simulink model "PMSMDriveThermal"  (R2025b)
(part 21 of 24)

  Battery (Table-Based)25 : batteryecm_lib/Battery (Table-Based)  SOC_vec=[0.1, 0.188889, 0.277778, 0.366667, 0.455556, 0.544444, 0.633333, 0.722222, 0.811111, 0.9]  T_dependence=simscape.enum.tablebattery.temperature_dependence.yes  prm_dir=simscape.enum.tablebattery.prm_dir.noCurrentDirectionality  T_vec=[30, 32.5, 35, 38] degC  V0_mat=|  V0_vec=[3.5057, 3.566, 3.6337, 3.7127, 3.9259, 4.0777, 4.1928] V  V_range=[0, inf] V  R0_mat=|  R0_vec=[.0085, .0085, .0087, .0082, .0083, .0085, .0085] Ohm  R0_dis_mat=[.0117, .0085, .009; .011, .0085, .009; .0114, .0087, .0092; .0107, .0082, .0088; .0107, .0083, .0091; .0113, .0085, .0089; .0116, .0085, .0089] Ohm  R0_dis_vec=[.0085, .0085, .0087, .0082, .0083, .0085, .0085] Ohm  R0_ch_mat=[.0117, .0085, .009; .011, .0085, .009; .0114, .0087, .0092; .0107, .0082, .0088; .0107, .0083, .0091; .0113, .0085, .0089; .0116, .0085, .0089] Ohm  R0_ch_vec=[.0085, .0085, .0087, .0082, .0083, .0085, .0085] Ohm  AH=5 A*hr  prm_leak=simscape.enum.tablebattery.prm_leak.disabled  Rleak_vec=[8000, 7000, 6000] Ohm  Rleak=7e3 Ohm  extrapolation_option=simscape.enum.extrapolation.nearest  SOC_port=simscape.enum.tablebattery.enable.no  prm_dyn=simscape.enum.tablebattery.prm_dyn.rc2  R1_mat=|  R1_vec=[.0029, .0024, .0026, .0016, .0023, .0018, .0017] Ohm  tau1_mat=|  tau1_vec=[36, 45, 105, 29, 77, 33, 39] s  R2_mat=|  R2_vec=[.0029, .0024, .0026, .0016, .0023, .0018, .0017] Ohm  tau2_mat=|  tau2_vec=[36, 45, 105, 29, 77, 33, 39] s  R3_mat=[.0109, .0029, .0013; .0069, .0024, .0012; .0047, .0026, .0013; .0034, .0016, .001; .0033, .0023, .0014; .0033, .0018, .0011; .0028, .0017, .0011] Ohm  R3_vec=[.0029, .0024, .0026, .0016, .0023, .0018, .0017] Ohm  tau3_mat=[20, 36, 39; 31, 45, 39; 109, 105, 61; 36, 29, 26; 59, 77, 67; 40, 33, 29; 25, 39, 33] s  tau3_vec=[36, 45, 105, 29, 77, 33, 39] s  R4_mat=[.0109, .0029, .0013; .0069, .0024, .0012; .0047, .0026, .0013; .0034, .0016, .001; .0033, .0023, .0014; .0033, .0018, .0011; .0028, .0017, .0011] Ohm  R4_vec=[.0029, .0024, .0026, .0016, .0023, .0018, .0017] Ohm  tau4_mat=[20, 36, 39; 31, 45, 39; 109, 105, 61; 36, 29, 26; 59, 77, 67; 40, 33, 29; 25, 39, 33] s  tau4_vec=[36, 45, 105, 29, 77, 33, 39] s  R5_mat=[.0109, .0029, .0013; .0069, .0024, .0012; .0047, .0026, .0013; .0034, .0016, .001; .0033, .0023, .0014; .0033, .0018, .0011; .0028, .0017, .0011] Ohm  R5_vec=[.0029, .0024, .0026, .0016, .0023, .0018, .0017] Ohm  tau5_mat=[20, 36, 39; 31, 45, 39; 109, 105, 61; 36, 29, 26; 59, 77, 67; 40, 33, 29; 25, 39, 33] s  tau5_vec=[36, 45, 105, 29, 77, 33, 39] s  prm_fade=simscape.enum.tablebattery.prm_fade.disabled  N0=100  dV0=0  dR0=0  dAH=0  dRleak=0  dR1=0  dR2=0  dR3=0  dR4=0  dR5=0  N0vec=[0, 100, 200, 300]  Tfadevec=[298.15, 323.15] K  dV0vec=[0, 0, 0, 0]  dR0vec=[0, 0, 0, 0]  dAHvec=[0, 0, 0, 0]  dRleakvec=[0, 0, 0, 0]  dR1vec=[0, 0, 0, 0]  dR2vec=[0, 0, 0, 0]  dR3vec=[0, 0, 0, 0]  dR4vec=[0, 0, 0, 0]  dR5vec=[0, 0, 0, 0]  dV0mat=[0, 0; 0, 0; 0, 0; 0, 0]  dR0mat=[0, 0; 0, 0; 0, 0; 0, 0]  dAHmat=[0, 0; 0, 0; 0, 0; 0, 0]  dRleakmat=[0, 0; 0, 0; 0, 0; 0, 0]  dR1mat=[0, 0; 0, 0; 0, 0; 0, 0]  dR2mat=[0, 0; 0, 0; 0, 0; 0, 0]  dR3mat=[0, 0; 0, 0; 0, 0; 0, 0]  dR4mat=[0, 0; 0, 0; 0, 0; 0, 0]  dR5mat=[0, 0; 0, 0; 0, 0; 0, 0]  prm_age_modeling=simscape.enum.tablebattery.prm_age_modeling.equation  storage_dt_age_vec=[0] d  storage_T_age_vec=[273] K  prm_age_OCV=simscape.enum.tablebattery.prm_age_OCV.OCV  OCV_age=0.9  SOC_age=0.6  prm_age_resistance=simscape.enum.tablebattery.prm_age.disabled  OCV_scaling_age_resistance=2.2134e6  OCV_offset_age_resistance=1.632e6  temp_exp_age_resistance=0.515833569 V  t_exp_age_resistance=0.75  T_age_vec_resistance=[273.15, 298.15, 323.15] K  dt_age_vec_resistance=[0, 90, 180, 270] d  dR0_age_vec=[0, 0, 0]  t_meas_dR0_age=100 d  dR0_age_mat=[0, 0, 0; 0, 0, 0; 0, 0, 0; 0, 0, 0]  prm_age_capacity=simscape.enum.tablebattery.prm_age.disabled  OCV_scaling_age_capacity=1.5097e07  OCV_offset_age_capacity=8.3625e06  temp_exp_age_capacity=0.6011 V  t_exp_age_capacity=0.75  T_age_vec_capacity=[273.15, 298.15, 323.15] K  dt_age_vec_capacity=[0, 90, 180, 270] d  dAH_age_vec=[0, 0, 0]  t_meas_dAH_age=100 d  dAH_age_mat=[0, 0, 0; 0, 0, 0; 0, 0, 0; 0, 0, 0]  thermal_port=simscape.enum.thermaleffects.omit  temperature=298.15 K  thermal_mass=100 J/K  i_specify=off  i_priority=None  i=0 A  i_nominal_specify=off  i_nominal_value=1  i_nominal_unit=A  v_specify=off  v_priority=None  v=0 V  v_nominal_specify=off  v_nominal_value=1  v_nominal_unit=V  stateOfCharge_specify=on  stateOfCharge_priority=High  stateOfCharge=1  stateOfCharge_nominal_specify=off  stateOfCharge_nominal_value=1  stateOfCharge_nominal_unit=1  num_cycles_specify=off  num_cycles_priority=High  num_cycles=0  num_cycles_nominal_specify=off  num_cycles_nominal_value=1  num_cycles_nominal_unit=1  cell_temperature_specify=off  cell_temperature_priority=High  cell_temperature=298.15 K  cell_temperature_nominal_specify=off  cell_temperature_nominal_value=1  cell_temperature_nominal_unit=K
      V0_mat=|
      | [3.0263, 3.218033, 3.364889, 3.493933, 3.610678, 3.733744, 3.85405, 3.950717, 4.040478, 4.0819;
      |  3.0376, 3.2248, 3.370311, 3.498533, 3.615311, 3.736956, 3.845633, 3.929256, 4.040056, 4.0821;
      |  3.0439, 3.227633, 3.3731, 3.5007, 3.616611, 3.737589, 3.8457, 3.9287, 4.039133, 4.0826;
      |  3.0283, 3.217989, 3.364589, 3.493767, 3.609467, 3.731156, 3.8417, 3.925833, 4.036322, 4.0821]' V
      R0_mat=|
      | [0.011867, 0.008993, 0.007674, 0.006911, 0.006648, 0.006648, 0.006528, 0.006157, 0.005996, 0.0073;
      |  0.0109, 0.006456, 0.005381, 0.005078, 0.005, 0.005044, 0.005511, 0.006407, 0.006522, 0.005367;
      |  0.0102, 0.007978, 0.006793, 0.0062, 0.006033, 0.005441, 0.0051, 0.005707, 0.005037, 0.005067;
      |  0.0101, 0.007759, 0.006637, 0.006022, 0.005741, 0.005667, 0.005311, 0.004911, 0.005859, 0.004733]' Ohm
      R1_mat=|
      | [0.007451, 0.008294, 0.007745, 0.007391;
      |  0.003783, 0.00363, 0.004415, 0.004051;
      |  0.002841, 0.00298, 0.003698, 0.003391;
      |  0.003185, 0.002661, 0.003493, 0.00379;
      |  0.00379, 0.003147, 0.004204, 0.004229;
      |  0.004015, 0.003677, 0.004233, 0.004481;
      |  0.003791, 0.004051, 0.003886, 0.004189;
      |  0.003416, 0.004883, 0.004387, 0.003743;
      |  0.00328, 0.005238, 0.003472, 0.004883;
      |  0.004816, 0.004218, 0.003847, 0.003891] Ohm
      tau1_mat=|
      | [8.156247, 6.866126, 6.747335, 6.573366;
      |  6.436096, 6.88158, 6.206576, 5.30011;
      |  7.074429, 7.267109, 6.564215, 5.759928;
      |  8.61232, 7.062398, 6.553799, 7.485573;
      |  10.88135, 8.569373, 8.681328, 8.99043;
      |  11.88702, 10.35435, 10.74073, 9.985533;
      |  11.15433, 10.61987, 10.52072, 10.95124;
      |  10.33388, 9.573709, 9.987626, 10.94588;
      |  9.883806, 9.219359, 8.513241, 9.109378;
      |  11.2706, 10.03414, 9.643065, 10.06297] s
      R2_mat=|
      | [0.040653, 0.04799, 0.046915, 0.044404;
      |  0.026828, 0.033189, 0.032279, 0.030363;
      |  0.019744, 0.025225, 0.021211, 0.019613;
      |  0.012414, 0.014827, 0.017004, 0.016763;
      |  0.007363, 0.008356, 0.01135, 0.010173;
      |  0.005882, 0.007703, 0.006532, 0.005526;
      |  0.006739, 0.007058, 0.006772, 0.005603;
      |  0.008222, 0.004287, 0.009601, 0.005034;
      |  0.008985, 0.007821, 0.008932, 0.006662;
      |  0.004704, 0.003171, 0.002422, 0.004036] Ohm
      tau2_mat=|
      | [131.6948, 137.0217, 141.2851, 129.3807;
      |  146.2759, 158.6208, 157.255, 143.944;
      |  158.5443, 177.3225, 156.7434, 144.0735;
      |  144.8009, 123.279, 145.0945, 176.1753;
      |  158.7596, 137.3241, 203.2495, 189.2199;
      |  149.8847, 154.5014, 161.1061, 146.3519;
      |  135.3572, 173.7062, 166.0613, 159.34;
      |  123.823, 144.5727, 209.652, 117.4544;
      |  111.7616, 98.04929, 114.3433, 98.05822;
      |  125.3862, 75.97092, 110.7081, 120.3015] s
      settings: InternalSimscapePortConfiguration="{\"Bottom\":[],\"Left\":[{\"id\":\"p\",\"label\":\"+\",\"type\":\"foundation.electrical.electrical\"}],\"Right\":[{\"id\":\"n\",\"label\":\"-\",\"type\":\"foundation.electrical.electrical\"}],\"Top\":[]}"
      settings: LibrarySourceBlock=|
      | batt_lib/Cells/Battery
      | (Table-Based)
  Battery (Table-Based)26 : batteryecm_lib/Battery (Table-Based)  SOC_vec=[0.1, 0.188889, 0.277778, 0.366667, 0.455556, 0.544444, 0.633333, 0.722222, 0.811111, 0.9]  T_dependence=simscape.enum.tablebattery.temperature_dependence.yes  prm_dir=simscape.enum.tablebattery.prm_dir.noCurrentDirectionality  T_vec=[30, 32.5, 35, 38] degC  V0_mat=|  V0_vec=[3.5057, 3.566, 3.6337, 3.7127, 3.9259, 4.0777, 4.1928] V  V_range=[0, inf] V  R0_mat=|  R0_vec=[.0085, .0085, .0087, .0082, .0083, .0085, .0085] Ohm  R0_dis_mat=[.0117, .0085, .009; .011, .0085, .009; .0114, .0087, .0092; .0107, .0082, .0088; .0107, .0083, .0091; .0113, .0085, .0089; .0116, .0085, .0089] Ohm  R0_dis_vec=[.0085, .0085, .0087, .0082, .0083, .0085, .0085] Ohm  R0_ch_mat=[.0117, .0085, .009; .011, .0085, .009; .0114, .0087, .0092; .0107, .0082, .0088; .0107, .0083, .0091; .0113, .0085, .0089; .0116, .0085, .0089] Ohm  R0_ch_vec=[.0085, .0085, .0087, .0082, .0083, .0085, .0085] Ohm  AH=5 A*hr  prm_leak=simscape.enum.tablebattery.prm_leak.disabled  Rleak_vec=[8000, 7000, 6000] Ohm  Rleak=7e3 Ohm  extrapolation_option=simscape.enum.extrapolation.nearest  SOC_port=simscape.enum.tablebattery.enable.no  prm_dyn=simscape.enum.tablebattery.prm_dyn.rc2  R1_mat=|  R1_vec=[.0029, .0024, .0026, .0016, .0023, .0018, .0017] Ohm  tau1_mat=|  tau1_vec=[36, 45, 105, 29, 77, 33, 39] s  R2_mat=|  R2_vec=[.0029, .0024, .0026, .0016, .0023, .0018, .0017] Ohm  tau2_mat=|  tau2_vec=[36, 45, 105, 29, 77, 33, 39] s  R3_mat=[.0109, .0029, .0013; .0069, .0024, .0012; .0047, .0026, .0013; .0034, .0016, .001; .0033, .0023, .0014; .0033, .0018, .0011; .0028, .0017, .0011] Ohm  R3_vec=[.0029, .0024, .0026, .0016, .0023, .0018, .0017] Ohm  tau3_mat=[20, 36, 39; 31, 45, 39; 109, 105, 61; 36, 29, 26; 59, 77, 67; 40, 33, 29; 25, 39, 33] s  tau3_vec=[36, 45, 105, 29, 77, 33, 39] s  R4_mat=[.0109, .0029, .0013; .0069, .0024, .0012; .0047, .0026, .0013; .0034, .0016, .001; .0033, .0023, .0014; .0033, .0018, .0011; .0028, .0017, .0011] Ohm  R4_vec=[.0029, .0024, .0026, .0016, .0023, .0018, .0017] Ohm  tau4_mat=[20, 36, 39; 31, 45, 39; 109, 105, 61; 36, 29, 26; 59, 77, 67; 40, 33, 29; 25, 39, 33] s  tau4_vec=[36, 45, 105, 29, 77, 33, 39] s  R5_mat=[.0109, .0029, .0013; .0069, .0024, .0012; .0047, .0026, .0013; .0034, .0016, .001; .0033, .0023, .0014; .0033, .0018, .0011; .0028, .0017, .0011] Ohm  R5_vec=[.0029, .0024, .0026, .0016, .0023, .0018, .0017] Ohm  tau5_mat=[20, 36, 39; 31, 45, 39; 109, 105, 61; 36, 29, 26; 59, 77, 67; 40, 33, 29; 25, 39, 33] s  tau5_vec=[36, 45, 105, 29, 77, 33, 39] s  prm_fade=simscape.enum.tablebattery.prm_fade.disabled  N0=100  dV0=0  dR0=0  dAH=0  dRleak=0  dR1=0  dR2=0  dR3=0  dR4=0  dR5=0  N0vec=[0, 100, 200, 300]  Tfadevec=[298.15, 323.15] K  dV0vec=[0, 0, 0, 0]  dR0vec=[0, 0, 0, 0]  dAHvec=[0, 0, 0, 0]  dRleakvec=[0, 0, 0, 0]  dR1vec=[0, 0, 0, 0]  dR2vec=[0, 0, 0, 0]  dR3vec=[0, 0, 0, 0]  dR4vec=[0, 0, 0, 0]  dR5vec=[0, 0, 0, 0]  dV0mat=[0, 0; 0, 0; 0, 0; 0, 0]  dR0mat=[0, 0; 0, 0; 0, 0; 0, 0]  dAHmat=[0, 0; 0, 0; 0, 0; 0, 0]  dRleakmat=[0, 0; 0, 0; 0, 0; 0, 0]  dR1mat=[0, 0; 0, 0; 0, 0; 0, 0]  dR2mat=[0, 0; 0, 0; 0, 0; 0, 0]  dR3mat=[0, 0; 0, 0; 0, 0; 0, 0]  dR4mat=[0, 0; 0, 0; 0, 0; 0, 0]  dR5mat=[0, 0; 0, 0; 0, 0; 0, 0]  prm_age_modeling=simscape.enum.tablebattery.prm_age_modeling.equation  storage_dt_age_vec=[0] d  storage_T_age_vec=[273] K  prm_age_OCV=simscape.enum.tablebattery.prm_age_OCV.OCV  OCV_age=0.9  SOC_age=0.6  prm_age_resistance=simscape.enum.tablebattery.prm_age.disabled  OCV_scaling_age_resistance=2.2134e6  OCV_offset_age_resistance=1.632e6  temp_exp_age_resistance=0.515833569 V  t_exp_age_resistance=0.75  T_age_vec_resistance=[273.15, 298.15, 323.15] K  dt_age_vec_resistance=[0, 90, 180, 270] d  dR0_age_vec=[0, 0, 0]  t_meas_dR0_age=100 d  dR0_age_mat=[0, 0, 0; 0, 0, 0; 0, 0, 0; 0, 0, 0]  prm_age_capacity=simscape.enum.tablebattery.prm_age.disabled  OCV_scaling_age_capacity=1.5097e07  OCV_offset_age_capacity=8.3625e06  temp_exp_age_capacity=0.6011 V  t_exp_age_capacity=0.75  T_age_vec_capacity=[273.15, 298.15, 323.15] K  dt_age_vec_capacity=[0, 90, 180, 270] d  dAH_age_vec=[0, 0, 0]  t_meas_dAH_age=100 d  dAH_age_mat=[0, 0, 0; 0, 0, 0; 0, 0, 0; 0, 0, 0]  thermal_port=simscape.enum.thermaleffects.omit  temperature=298.15 K  thermal_mass=100 J/K  i_specify=off  i_priority=None  i=0 A  i_nominal_specify=off  i_nominal_value=1  i_nominal_unit=A  v_specify=off  v_priority=None  v=0 V  v_nominal_specify=off  v_nominal_value=1  v_nominal_unit=V  stateOfCharge_specify=on  stateOfCharge_priority=High  stateOfCharge=1  stateOfCharge_nominal_specify=off  stateOfCharge_nominal_value=1  stateOfCharge_nominal_unit=1  num_cycles_specify=off  num_cycles_priority=High  num_cycles=0  num_cycles_nominal_specify=off  num_cycles_nominal_value=1  num_cycles_nominal_unit=1  cell_temperature_specify=off  cell_temperature_priority=High  cell_temperature=298.15 K  cell_temperature_nominal_specify=off  cell_temperature_nominal_value=1  cell_temperature_nominal_unit=K
      V0_mat=|
      | [3.0263, 3.218033, 3.364889, 3.493933, 3.610678, 3.733744, 3.85405, 3.950717, 4.040478, 4.0819;
      |  3.0376, 3.2248, 3.370311, 3.498533, 3.615311, 3.736956, 3.845633, 3.929256, 4.040056, 4.0821;
      |  3.0439, 3.227633, 3.3731, 3.5007, 3.616611, 3.737589, 3.8457, 3.9287, 4.039133, 4.0826;
      |  3.0283, 3.217989, 3.364589, 3.493767, 3.609467, 3.731156, 3.8417, 3.925833, 4.036322, 4.0821]' V
      R0_mat=|
      | [0.011867, 0.008993, 0.007674, 0.006911, 0.006648, 0.006648, 0.006528, 0.006157, 0.005996, 0.0073;
      |  0.0109, 0.006456, 0.005381, 0.005078, 0.005, 0.005044, 0.005511, 0.006407, 0.006522, 0.005367;
      |  0.0102, 0.007978, 0.006793, 0.0062, 0.006033, 0.005441, 0.0051, 0.005707, 0.005037, 0.005067;
      |  0.0101, 0.007759, 0.006637, 0.006022, 0.005741, 0.005667, 0.005311, 0.004911, 0.005859, 0.004733]' Ohm
      R1_mat=|
      | [0.007451, 0.008294, 0.007745, 0.007391;
      |  0.003783, 0.00363, 0.004415, 0.004051;
      |  0.002841, 0.00298, 0.003698, 0.003391;
      |  0.003185, 0.002661, 0.003493, 0.00379;
      |  0.00379, 0.003147, 0.004204, 0.004229;
      |  0.004015, 0.003677, 0.004233, 0.004481;
      |  0.003791, 0.004051, 0.003886, 0.004189;
      |  0.003416, 0.004883, 0.004387, 0.003743;
      |  0.00328, 0.005238, 0.003472, 0.004883;
      |  0.004816, 0.004218, 0.003847, 0.003891] Ohm
      tau1_mat=|
      | [8.156247, 6.866126, 6.747335, 6.573366;
      |  6.436096, 6.88158, 6.206576, 5.30011;
      |  7.074429, 7.267109, 6.564215, 5.759928;
      |  8.61232, 7.062398, 6.553799, 7.485573;
      |  10.88135, 8.569373, 8.681328, 8.99043;
      |  11.88702, 10.35435, 10.74073, 9.985533;
      |  11.15433, 10.61987, 10.52072, 10.95124;
      |  10.33388, 9.573709, 9.987626, 10.94588;
      |  9.883806, 9.219359, 8.513241, 9.109378;
      |  11.2706, 10.03414, 9.643065, 10.06297] s
      R2_mat=|
      | [0.040653, 0.04799, 0.046915, 0.044404;
      |  0.026828, 0.033189, 0.032279, 0.030363;
      |  0.019744, 0.025225, 0.021211, 0.019613;
      |  0.012414, 0.014827, 0.017004, 0.016763;
      |  0.007363, 0.008356, 0.01135, 0.010173;
      |  0.005882, 0.007703, 0.006532, 0.005526;
      |  0.006739, 0.007058, 0.006772, 0.005603;
      |  0.008222, 0.004287, 0.009601, 0.005034;
      |  0.008985, 0.007821, 0.008932, 0.006662;
      |  0.004704, 0.003171, 0.002422, 0.004036] Ohm
      tau2_mat=|
      | [131.6948, 137.0217, 141.2851, 129.3807;
      |  146.2759, 158.6208, 157.255, 143.944;
      |  158.5443, 177.3225, 156.7434, 144.0735;
      |  144.8009, 123.279, 145.0945, 176.1753;
      |  158.7596, 137.3241, 203.2495, 189.2199;
      |  149.8847, 154.5014, 161.1061, 146.3519;
      |  135.3572, 173.7062, 166.0613, 159.34;
      |  123.823, 144.5727, 209.652, 117.4544;
      |  111.7616, 98.04929, 114.3433, 98.05822;
      |  125.3862, 75.97092, 110.7081, 120.3015] s
      settings: InternalSimscapePortConfiguration="{\"Bottom\":[],\"Left\":[{\"id\":\"p\",\"label\":\"+\",\"type\":\"foundation.electrical.electrical\"}],\"Right\":[{\"id\":\"n\",\"label\":\"-\",\"type\":\"foundation.electrical.electrical\"}],\"Top\":[]}"
      settings: LibrarySourceBlock=|
      | batt_lib/Cells/Battery
      | (Table-Based)
  Battery (Table-Based)27 : batteryecm_lib/Battery (Table-Based)  SOC_vec=[0.1, 0.188889, 0.277778, 0.366667, 0.455556, 0.544444, 0.633333, 0.722222, 0.811111, 0.9]  T_dependence=simscape.enum.tablebattery.temperature_dependence.yes  prm_dir=simscape.enum.tablebattery.prm_dir.noCurrentDirectionality  T_vec=[30, 32.5, 35, 38] degC  V0_mat=|  V0_vec=[3.5057, 3.566, 3.6337, 3.7127, 3.9259, 4.0777, 4.1928] V  V_range=[0, inf] V  R0_mat=|  R0_vec=[.0085, .0085, .0087, .0082, .0083, .0085, .0085] Ohm  R0_dis_mat=[.0117, .0085, .009; .011, .0085, .009; .0114, .0087, .0092; .0107, .0082, .0088; .0107, .0083, .0091; .0113, .0085, .0089; .0116, .0085, .0089] Ohm  R0_dis_vec=[.0085, .0085, .0087, .0082, .0083, .0085, .0085] Ohm  R0_ch_mat=[.0117, .0085, .009; .011, .0085, .009; .0114, .0087, .0092; .0107, .0082, .0088; .0107, .0083, .0091; .0113, .0085, .0089; .0116, .0085, .0089] Ohm  R0_ch_vec=[.0085, .0085, .0087, .0082, .0083, .0085, .0085] Ohm  AH=5 A*hr  prm_leak=simscape.enum.tablebattery.prm_leak.disabled  Rleak_vec=[8000, 7000, 6000] Ohm  Rleak=7e3 Ohm  extrapolation_option=simscape.enum.extrapolation.nearest  SOC_port=simscape.enum.tablebattery.enable.no  prm_dyn=simscape.enum.tablebattery.prm_dyn.rc2  R1_mat=|  R1_vec=[.0029, .0024, .0026, .0016, .0023, .0018, .0017] Ohm  tau1_mat=|  tau1_vec=[36, 45, 105, 29, 77, 33, 39] s  R2_mat=|  R2_vec=[.0029, .0024, .0026, .0016, .0023, .0018, .0017] Ohm  tau2_mat=|  tau2_vec=[36, 45, 105, 29, 77, 33, 39] s  R3_mat=[.0109, .0029, .0013; .0069, .0024, .0012; .0047, .0026, .0013; .0034, .0016, .001; .0033, .0023, .0014; .0033, .0018, .0011; .0028, .0017, .0011] Ohm  R3_vec=[.0029, .0024, .0026, .0016, .0023, .0018, .0017] Ohm  tau3_mat=[20, 36, 39; 31, 45, 39; 109, 105, 61; 36, 29, 26; 59, 77, 67; 40, 33, 29; 25, 39, 33] s  tau3_vec=[36, 45, 105, 29, 77, 33, 39] s  R4_mat=[.0109, .0029, .0013; .0069, .0024, .0012; .0047, .0026, .0013; .0034, .0016, .001; .0033, .0023, .0014; .0033, .0018, .0011; .0028, .0017, .0011] Ohm  R4_vec=[.0029, .0024, .0026, .0016, .0023, .0018, .0017] Ohm  tau4_mat=[20, 36, 39; 31, 45, 39; 109, 105, 61; 36, 29, 26; 59, 77, 67; 40, 33, 29; 25, 39, 33] s  tau4_vec=[36, 45, 105, 29, 77, 33, 39] s  R5_mat=[.0109, .0029, .0013; .0069, .0024, .0012; .0047, .0026, .0013; .0034, .0016, .001; .0033, .0023, .0014; .0033, .0018, .0011; .0028, .0017, .0011] Ohm  R5_vec=[.0029, .0024, .0026, .0016, .0023, .0018, .0017] Ohm  tau5_mat=[20, 36, 39; 31, 45, 39; 109, 105, 61; 36, 29, 26; 59, 77, 67; 40, 33, 29; 25, 39, 33] s  tau5_vec=[36, 45, 105, 29, 77, 33, 39] s  prm_fade=simscape.enum.tablebattery.prm_fade.disabled  N0=100  dV0=0  dR0=0  dAH=0  dRleak=0  dR1=0  dR2=0  dR3=0  dR4=0  dR5=0  N0vec=[0, 100, 200, 300]  Tfadevec=[298.15, 323.15] K  dV0vec=[0, 0, 0, 0]  dR0vec=[0, 0, 0, 0]  dAHvec=[0, 0, 0, 0]  dRleakvec=[0, 0, 0, 0]  dR1vec=[0, 0, 0, 0]  dR2vec=[0, 0, 0, 0]  dR3vec=[0, 0, 0, 0]  dR4vec=[0, 0, 0, 0]  dR5vec=[0, 0, 0, 0]  dV0mat=[0, 0; 0, 0; 0, 0; 0, 0]  dR0mat=[0, 0; 0, 0; 0, 0; 0, 0]  dAHmat=[0, 0; 0, 0; 0, 0; 0, 0]  dRleakmat=[0, 0; 0, 0; 0, 0; 0, 0]  dR1mat=[0, 0; 0, 0; 0, 0; 0, 0]  dR2mat=[0, 0; 0, 0; 0, 0; 0, 0]  dR3mat=[0, 0; 0, 0; 0, 0; 0, 0]  dR4mat=[0, 0; 0, 0; 0, 0; 0, 0]  dR5mat=[0, 0; 0, 0; 0, 0; 0, 0]  prm_age_modeling=simscape.enum.tablebattery.prm_age_modeling.equation  storage_dt_age_vec=[0] d  storage_T_age_vec=[273] K  prm_age_OCV=simscape.enum.tablebattery.prm_age_OCV.OCV  OCV_age=0.9  SOC_age=0.6  prm_age_resistance=simscape.enum.tablebattery.prm_age.disabled  OCV_scaling_age_resistance=2.2134e6  OCV_offset_age_resistance=1.632e6  temp_exp_age_resistance=0.515833569 V  t_exp_age_resistance=0.75  T_age_vec_resistance=[273.15, 298.15, 323.15] K  dt_age_vec_resistance=[0, 90, 180, 270] d  dR0_age_vec=[0, 0, 0]  t_meas_dR0_age=100 d  dR0_age_mat=[0, 0, 0; 0, 0, 0; 0, 0, 0; 0, 0, 0]  prm_age_capacity=simscape.enum.tablebattery.prm_age.disabled  OCV_scaling_age_capacity=1.5097e07  OCV_offset_age_capacity=8.3625e06  temp_exp_age_capacity=0.6011 V  t_exp_age_capacity=0.75  T_age_vec_capacity=[273.15, 298.15, 323.15] K  dt_age_vec_capacity=[0, 90, 180, 270] d  dAH_age_vec=[0, 0, 0]  t_meas_dAH_age=100 d  dAH_age_mat=[0, 0, 0; 0, 0, 0; 0, 0, 0; 0, 0, 0]  thermal_port=simscape.enum.thermaleffects.omit  temperature=298.15 K  thermal_mass=100 J/K  i_specify=off  i_priority=None  i=0 A  i_nominal_specify=off  i_nominal_value=1  i_nominal_unit=A  v_specify=off  v_priority=None  v=0 V  v_nominal_specify=off  v_nominal_value=1  v_nominal_unit=V  stateOfCharge_specify=on  stateOfCharge_priority=High  stateOfCharge=1  stateOfCharge_nominal_specify=off  stateOfCharge_nominal_value=1  stateOfCharge_nominal_unit=1  num_cycles_specify=off  num_cycles_priority=High  num_cycles=0  num_cycles_nominal_specify=off  num_cycles_nominal_value=1  num_cycles_nominal_unit=1  cell_temperature_specify=off  cell_temperature_priority=High  cell_temperature=298.15 K  cell_temperature_nominal_specify=off  cell_temperature_nominal_value=1  cell_temperature_nominal_unit=K
      V0_mat=|
      | [3.0263, 3.218033, 3.364889, 3.493933, 3.610678, 3.733744, 3.85405, 3.950717, 4.040478, 4.0819;
      |  3.0376, 3.2248, 3.370311, 3.498533, 3.615311, 3.736956, 3.845633, 3.929256, 4.040056, 4.0821;
      |  3.0439, 3.227633, 3.3731, 3.5007, 3.616611, 3.737589, 3.8457, 3.9287, 4.039133, 4.0826;
      |  3.0283, 3.217989, 3.364589, 3.493767, 3.609467, 3.731156, 3.8417, 3.925833, 4.036322, 4.0821]' V
      R0_mat=|
      | [0.011867, 0.008993, 0.007674, 0.006911, 0.006648, 0.006648, 0.006528, 0.006157, 0.005996, 0.0073;
      |  0.0109, 0.006456, 0.005381, 0.005078, 0.005, 0.005044, 0.005511, 0.006407, 0.006522, 0.005367;
      |  0.0102, 0.007978, 0.006793, 0.0062, 0.006033, 0.005441, 0.0051, 0.005707, 0.005037, 0.005067;
      |  0.0101, 0.007759, 0.006637, 0.006022, 0.005741, 0.005667, 0.005311, 0.004911, 0.005859, 0.004733]' Ohm
      R1_mat=|
      | [0.007451, 0.008294, 0.007745, 0.007391;
      |  0.003783, 0.00363, 0.004415, 0.004051;
      |  0.002841, 0.00298, 0.003698, 0.003391;
      |  0.003185, 0.002661, 0.003493, 0.00379;
      |  0.00379, 0.003147, 0.004204, 0.004229;
      |  0.004015, 0.003677, 0.004233, 0.004481;
      |  0.003791, 0.004051, 0.003886, 0.004189;
      |  0.003416, 0.004883, 0.004387, 0.003743;
      |  0.00328, 0.005238, 0.003472, 0.004883;
      |  0.004816, 0.004218, 0.003847, 0.003891] Ohm
      tau1_mat=|
      | [8.156247, 6.866126, 6.747335, 6.573366;
      |  6.436096, 6.88158, 6.206576, 5.30011;
      |  7.074429, 7.267109, 6.564215, 5.759928;
      |  8.61232, 7.062398, 6.553799, 7.485573;
      |  10.88135, 8.569373, 8.681328, 8.99043;
      |  11.88702, 10.35435, 10.74073, 9.985533;
      |  11.15433, 10.61987, 10.52072, 10.95124;
      |  10.33388, 9.573709, 9.987626, 10.94588;
      |  9.883806, 9.219359, 8.513241, 9.109378;
      |  11.2706, 10.03414, 9.643065, 10.06297] s
      R2_mat=|
      | [0.040653, 0.04799, 0.046915, 0.044404;
      |  0.026828, 0.033189, 0.032279, 0.030363;
      |  0.019744, 0.025225, 0.021211, 0.019613;
      |  0.012414, 0.014827, 0.017004, 0.016763;
      |  0.007363, 0.008356, 0.01135, 0.010173;
      |  0.005882, 0.007703, 0.006532, 0.005526;
      |  0.006739, 0.007058, 0.006772, 0.005603;
      |  0.008222, 0.004287, 0.009601, 0.005034;
      |  0.008985, 0.007821, 0.008932, 0.006662;
      |  0.004704, 0.003171, 0.002422, 0.004036] Ohm
      tau2_mat=|
      | [131.6948, 137.0217, 141.2851, 129.3807;
      |  146.2759, 158.6208, 157.255, 143.944;
      |  158.5443, 177.3225, 156.7434, 144.0735;
      |  144.8009, 123.279, 145.0945, 176.1753;
      |  158.7596, 137.3241, 203.2495, 189.2199;
      |  149.8847, 154.5014, 161.1061, 146.3519;
      |  135.3572, 173.7062, 166.0613, 159.34;
      |  123.823, 144.5727, 209.652, 117.4544;
      |  111.7616, 98.04929, 114.3433, 98.05822;
      |  125.3862, 75.97092, 110.7081, 120.3015] s
      settings: InternalSimscapePortConfiguration="{\"Bottom\":[],\"Left\":[{\"id\":\"p\",\"label\":\"+\",\"type\":\"foundation.electrical.electrical\"}],\"Right\":[{\"id\":\"n\",\"label\":\"-\",\"type\":\"foundation.electrical.electrical\"}],\"Top\":[]}"
      settings: LibrarySourceBlock=|
      | batt_lib/Cells/Battery
      | (Table-Based)
  Battery (Table-Based)28 : batteryecm_lib/Battery (Table-Based)  SOC_vec=[0.1, 0.188889, 0.277778, 0.366667, 0.455556, 0.544444, 0.633333, 0.722222, 0.811111, 0.9]  T_dependence=simscape.enum.tablebattery.temperature_dependence.yes  prm_dir=simscape.enum.tablebattery.prm_dir.noCurrentDirectionality  T_vec=[30, 32.5, 35, 38] degC  V0_mat=|  V0_vec=[3.5057, 3.566, 3.6337, 3.7127, 3.9259, 4.0777, 4.1928] V  V_range=[0, inf] V  R0_mat=|  R0_vec=[.0085, .0085, .0087, .0082, .0083, .0085, .0085] Ohm  R0_dis_mat=[.0117, .0085, .009; .011, .0085, .009; .0114, .0087, .0092; .0107, .0082, .0088; .0107, .0083, .0091; .0113, .0085, .0089; .0116, .0085, .0089] Ohm  R0_dis_vec=[.0085, .0085, .0087, .0082, .0083, .0085, .0085] Ohm  R0_ch_mat=[.0117, .0085, .009; .011, .0085, .009; .0114, .0087, .0092; .0107, .0082, .0088; .0107, .0083, .0091; .0113, .0085, .0089; .0116, .0085, .0089] Ohm  R0_ch_vec=[.0085, .0085, .0087, .0082, .0083, .0085, .0085] Ohm  AH=5 A*hr  prm_leak=simscape.enum.tablebattery.prm_leak.disabled  Rleak_vec=[8000, 7000, 6000] Ohm  Rleak=7e3 Ohm  extrapolation_option=simscape.enum.extrapolation.nearest  SOC_port=simscape.enum.tablebattery.enable.no  prm_dyn=simscape.enum.tablebattery.prm_dyn.rc2  R1_mat=|  R1_vec=[.0029, .0024, .0026, .0016, .0023, .0018, .0017] Ohm  tau1_mat=|  tau1_vec=[36, 45, 105, 29, 77, 33, 39] s  R2_mat=|  R2_vec=[.0029, .0024, .0026, .0016, .0023, .0018, .0017] Ohm  tau2_mat=|  tau2_vec=[36, 45, 105, 29, 77, 33, 39] s  R3_mat=[.0109, .0029, .0013; .0069, .0024, .0012; .0047, .0026, .0013; .0034, .0016, .001; .0033, .0023, .0014; .0033, .0018, .0011; .0028, .0017, .0011] Ohm  R3_vec=[.0029, .0024, .0026, .0016, .0023, .0018, .0017] Ohm  tau3_mat=[20, 36, 39; 31, 45, 39; 109, 105, 61; 36, 29, 26; 59, 77, 67; 40, 33, 29; 25, 39, 33] s  tau3_vec=[36, 45, 105, 29, 77, 33, 39] s  R4_mat=[.0109, .0029, .0013; .0069, .0024, .0012; .0047, .0026, .0013; .0034, .0016, .001; .0033, .0023, .0014; .0033, .0018, .0011; .0028, .0017, .0011] Ohm  R4_vec=[.0029, .0024, .0026, .0016, .0023, .0018, .0017] Ohm  tau4_mat=[20, 36, 39; 31, 45, 39; 109, 105, 61; 36, 29, 26; 59, 77, 67; 40, 33, 29; 25, 39, 33] s  tau4_vec=[36, 45, 105, 29, 77, 33, 39] s  R5_mat=[.0109, .0029, .0013; .0069, .0024, .0012; .0047, .0026, .0013; .0034, .0016, .001; .0033, .0023, .0014; .0033, .0018, .0011; .0028, .0017, .0011] Ohm  R5_vec=[.0029, .0024, .0026, .0016, .0023, .0018, .0017] Ohm  tau5_mat=[20, 36, 39; 31, 45, 39; 109, 105, 61; 36, 29, 26; 59, 77, 67; 40, 33, 29; 25, 39, 33] s  tau5_vec=[36, 45, 105, 29, 77, 33, 39] s  prm_fade=simscape.enum.tablebattery.prm_fade.disabled  N0=100  dV0=0  dR0=0  dAH=0  dRleak=0  dR1=0  dR2=0  dR3=0  dR4=0  dR5=0  N0vec=[0, 100, 200, 300]  Tfadevec=[298.15, 323.15] K  dV0vec=[0, 0, 0, 0]  dR0vec=[0, 0, 0, 0]  dAHvec=[0, 0, 0, 0]  dRleakvec=[0, 0, 0, 0]  dR1vec=[0, 0, 0, 0]  dR2vec=[0, 0, 0, 0]  dR3vec=[0, 0, 0, 0]  dR4vec=[0, 0, 0, 0]  dR5vec=[0, 0, 0, 0]  dV0mat=[0, 0; 0, 0; 0, 0; 0, 0]  dR0mat=[0, 0; 0, 0; 0, 0; 0, 0]  dAHmat=[0, 0; 0, 0; 0, 0; 0, 0]  dRleakmat=[0, 0; 0, 0; 0, 0; 0, 0]  dR1mat=[0, 0; 0, 0; 0, 0; 0, 0]  dR2mat=[0, 0; 0, 0; 0, 0; 0, 0]  dR3mat=[0, 0; 0, 0; 0, 0; 0, 0]  dR4mat=[0, 0; 0, 0; 0, 0; 0, 0]  dR5mat=[0, 0; 0, 0; 0, 0; 0, 0]  prm_age_modeling=simscape.enum.tablebattery.prm_age_modeling.equation  storage_dt_age_vec=[0] d  storage_T_age_vec=[273] K  prm_age_OCV=simscape.enum.tablebattery.prm_age_OCV.OCV  OCV_age=0.9  SOC_age=0.6  prm_age_resistance=simscape.enum.tablebattery.prm_age.disabled  OCV_scaling_age_resistance=2.2134e6  OCV_offset_age_resistance=1.632e6  temp_exp_age_resistance=0.515833569 V  t_exp_age_resistance=0.75  T_age_vec_resistance=[273.15, 298.15, 323.15] K  dt_age_vec_resistance=[0, 90, 180, 270] d  dR0_age_vec=[0, 0, 0]  t_meas_dR0_age=100 d  dR0_age_mat=[0, 0, 0; 0, 0, 0; 0, 0, 0; 0, 0, 0]  prm_age_capacity=simscape.enum.tablebattery.prm_age.disabled  OCV_scaling_age_capacity=1.5097e07  OCV_offset_age_capacity=8.3625e06  temp_exp_age_capacity=0.6011 V  t_exp_age_capacity=0.75  T_age_vec_capacity=[273.15, 298.15, 323.15] K  dt_age_vec_capacity=[0, 90, 180, 270] d  dAH_age_vec=[0, 0, 0]  t_meas_dAH_age=100 d  dAH_age_mat=[0, 0, 0; 0, 0, 0; 0, 0, 0; 0, 0, 0]  thermal_port=simscape.enum.thermaleffects.omit  temperature=298.15 K  thermal_mass=100 J/K  i_specify=off  i_priority=None  i=0 A  i_nominal_specify=off  i_nominal_value=1  i_nominal_unit=A  v_specify=off  v_priority=None  v=0 V  v_nominal_specify=off  v_nominal_value=1  v_nominal_unit=V  stateOfCharge_specify=off  stateOfCharge_priority=High  stateOfCharge=1  stateOfCharge_nominal_specify=off  stateOfCharge_nominal_value=1  stateOfCharge_nominal_unit=1  num_cycles_specify=off  num_cycles_priority=High  num_cycles=0  num_cycles_nominal_specify=off  num_cycles_nominal_value=1  num_cycles_nominal_unit=1  cell_temperature_specify=off  cell_temperature_priority=High  cell_temperature=298.15 K  cell_temperature_nominal_specify=off  cell_temperature_nominal_value=1  cell_temperature_nominal_unit=K
      V0_mat=|
      | [3.0263, 3.218033, 3.364889, 3.493933, 3.610678, 3.733744, 3.85405, 3.950717, 4.040478, 4.0819;
      |  3.0376, 3.2248, 3.370311, 3.498533, 3.615311, 3.736956, 3.845633, 3.929256, 4.040056, 4.0821;
      |  3.0439, 3.227633, 3.3731, 3.5007, 3.616611, 3.737589, 3.8457, 3.9287, 4.039133, 4.0826;
      |  3.0283, 3.217989, 3.364589, 3.493767, 3.609467, 3.731156, 3.8417, 3.925833, 4.036322, 4.0821]' V
      R0_mat=|
      | [0.011867, 0.008993, 0.007674, 0.006911, 0.006648, 0.006648, 0.006528, 0.006157, 0.005996, 0.0073;
      |  0.0109, 0.006456, 0.005381, 0.005078, 0.005, 0.005044, 0.005511, 0.006407, 0.006522, 0.005367;
      |  0.0102, 0.007978, 0.006793, 0.0062, 0.006033, 0.005441, 0.0051, 0.005707, 0.005037, 0.005067;
      |  0.0101, 0.007759, 0.006637, 0.006022, 0.005741, 0.005667, 0.005311, 0.004911, 0.005859, 0.004733]' Ohm
      R1_mat=|
      | [0.007451, 0.008294, 0.007745, 0.007391;
      |  0.003783, 0.00363, 0.004415, 0.004051;
      |  0.002841, 0.00298, 0.003698, 0.003391;
      |  0.003185, 0.002661, 0.003493, 0.00379;
      |  0.00379, 0.003147, 0.004204, 0.004229;
      |  0.004015, 0.003677, 0.004233, 0.004481;
      |  0.003791, 0.004051, 0.003886, 0.004189;
      |  0.003416, 0.004883, 0.004387, 0.003743;
      |  0.00328, 0.005238, 0.003472, 0.004883;
      |  0.004816, 0.004218, 0.003847, 0.003891] Ohm
      tau1_mat=|
      | [8.156247, 6.866126, 6.747335, 6.573366;
      |  6.436096, 6.88158, 6.206576, 5.30011;
      |  7.074429, 7.267109, 6.564215, 5.759928;
      |  8.61232, 7.062398, 6.553799, 7.485573;
      |  10.88135, 8.569373, 8.681328, 8.99043;
      |  11.88702, 10.35435, 10.74073, 9.985533;
      |  11.15433, 10.61987, 10.52072, 10.95124;
      |  10.33388, 9.573709, 9.987626, 10.94588;
      |  9.883806, 9.219359, 8.513241, 9.109378;
      |  11.2706, 10.03414, 9.643065, 10.06297] s
      R2_mat=|
      | [0.040653, 0.04799, 0.046915, 0.044404;
      |  0.026828, 0.033189, 0.032279, 0.030363;
      |  0.019744, 0.025225, 0.021211, 0.019613;
      |  0.012414, 0.014827, 0.017004, 0.016763;
      |  0.007363, 0.008356, 0.01135, 0.010173;
      |  0.005882, 0.007703, 0.006532, 0.005526;
      |  0.006739, 0.007058, 0.006772, 0.005603;
      |  0.008222, 0.004287, 0.009601, 0.005034;
      |  0.008985, 0.007821, 0.008932, 0.006662;
      |  0.004704, 0.003171, 0.002422, 0.004036] Ohm
      tau2_mat=|
      | [131.6948, 137.0217, 141.2851, 129.3807;
      |  146.2759, 158.6208, 157.255, 143.944;
      |  158.5443, 177.3225, 156.7434, 144.0735;
      |  144.8009, 123.279, 145.0945, 176.1753;
      |  158.7596, 137.3241, 203.2495, 189.2199;
      |  149.8847, 154.5014, 161.1061, 146.3519;
      |  135.3572, 173.7062, 166.0613, 159.34;
      |  123.823, 144.5727, 209.652, 117.4544;
      |  111.7616, 98.04929, 114.3433, 98.05822;
      |  125.3862, 75.97092, 110.7081, 120.3015] s
      settings: InternalSimscapePortConfiguration="{\"Bottom\":[],\"Left\":[{\"id\":\"p\",\"label\":\"+\",\"type\":\"foundation.electrical.electrical\"}],\"Right\":[{\"id\":\"n\",\"label\":\"-\",\"type\":\"foundation.electrical.electrical\"}],\"Top\":[]}"
      settings: LibrarySourceBlock=|
      | batt_lib/Cells/Battery
      | (Table-Based)
  Battery (Table-Based)29 : batteryecm_lib/Battery (Table-Based)  SOC_vec=[0.1, 0.188889, 0.277778, 0.366667, 0.455556, 0.544444, 0.633333, 0.722222, 0.811111, 0.9]  T_dependence=simscape.enum.tablebattery.temperature_dependence.yes  prm_dir=simscape.enum.tablebattery.prm_dir.noCurrentDirectionality  T_vec=[30, 32.5, 35, 38] degC  V0_mat=|  V0_vec=[3.5057, 3.566, 3.6337, 3.7127, 3.9259, 4.0777, 4.1928] V  V_range=[0, inf] V  R0_mat=|  R0_vec=[.0085, .0085, .0087, .0082, .0083, .0085, .0085] Ohm  R0_dis_mat=[.0117, .0085, .009; .011, .0085, .009; .0114, .0087, .0092; .0107, .0082, .0088; .0107, .0083, .0091; .0113, .0085, .0089; .0116, .0085, .0089] Ohm  R0_dis_vec=[.0085, .0085, .0087, .0082, .0083, .0085, .0085] Ohm  R0_ch_mat=[.0117, .0085, .009; .011, .0085, .009; .0114, .0087, .0092; .0107, .0082, .0088; .0107, .0083, .0091; .0113, .0085, .0089; .0116, .0085, .0089] Ohm  R0_ch_vec=[.0085, .0085, .0087, .0082, .0083, .0085, .0085] Ohm  AH=5 A*hr  prm_leak=simscape.enum.tablebattery.prm_leak.disabled  Rleak_vec=[8000, 7000, 6000] Ohm  Rleak=7e3 Ohm  extrapolation_option=simscape.enum.extrapolation.nearest  SOC_port=simscape.enum.tablebattery.enable.no  prm_dyn=simscape.enum.tablebattery.prm_dyn.rc2  R1_mat=|  R1_vec=[.0029, .0024, .0026, .0016, .0023, .0018, .0017] Ohm  tau1_mat=|  tau1_vec=[36, 45, 105, 29, 77, 33, 39] s  R2_mat=|  R2_vec=[.0029, .0024, .0026, .0016, .0023, .0018, .0017] Ohm  tau2_mat=|  tau2_vec=[36, 45, 105, 29, 77, 33, 39] s  R3_mat=[.0109, .0029, .0013; .0069, .0024, .0012; .0047, .0026, .0013; .0034, .0016, .001; .0033, .0023, .0014; .0033, .0018, .0011; .0028, .0017, .0011] Ohm  R3_vec=[.0029, .0024, .0026, .0016, .0023, .0018, .0017] Ohm  tau3_mat=[20, 36, 39; 31, 45, 39; 109, 105, 61; 36, 29, 26; 59, 77, 67; 40, 33, 29; 25, 39, 33] s  tau3_vec=[36, 45, 105, 29, 77, 33, 39] s  R4_mat=[.0109, .0029, .0013; .0069, .0024, .0012; .0047, .0026, .0013; .0034, .0016, .001; .0033, .0023, .0014; .0033, .0018, .0011; .0028, .0017, .0011] Ohm  R4_vec=[.0029, .0024, .0026, .0016, .0023, .0018, .0017] Ohm  tau4_mat=[20, 36, 39; 31, 45, 39; 109, 105, 61; 36, 29, 26; 59, 77, 67; 40, 33, 29; 25, 39, 33] s  tau4_vec=[36, 45, 105, 29, 77, 33, 39] s  R5_mat=[.0109, .0029, .0013; .0069, .0024, .0012; .0047, .0026, .0013; .0034, .0016, .001; .0033, .0023, .0014; .0033, .0018, .0011; .0028, .0017, .0011] Ohm  R5_vec=[.0029, .0024, .0026, .0016, .0023, .0018, .0017] Ohm  tau5_mat=[20, 36, 39; 31, 45, 39; 109, 105, 61; 36, 29, 26; 59, 77, 67; 40, 33, 29; 25, 39, 33] s  tau5_vec=[36, 45, 105, 29, 77, 33, 39] s  prm_fade=simscape.enum.tablebattery.prm_fade.disabled  N0=100  dV0=0  dR0=0  dAH=0  dRleak=0  dR1=0  dR2=0  dR3=0  dR4=0  dR5=0  N0vec=[0, 100, 200, 300]  Tfadevec=[298.15, 323.15] K  dV0vec=[0, 0, 0, 0]  dR0vec=[0, 0, 0, 0]  dAHvec=[0, 0, 0, 0]  dRleakvec=[0, 0, 0, 0]  dR1vec=[0, 0, 0, 0]  dR2vec=[0, 0, 0, 0]  dR3vec=[0, 0, 0, 0]  dR4vec=[0, 0, 0, 0]  dR5vec=[0, 0, 0, 0]  dV0mat=[0, 0; 0, 0; 0, 0; 0, 0]  dR0mat=[0, 0; 0, 0; 0, 0; 0, 0]  dAHmat=[0, 0; 0, 0; 0, 0; 0, 0]  dRleakmat=[0, 0; 0, 0; 0, 0; 0, 0]  dR1mat=[0, 0; 0, 0; 0, 0; 0, 0]  dR2mat=[0, 0; 0, 0; 0, 0; 0, 0]  dR3mat=[0, 0; 0, 0; 0, 0; 0, 0]  dR4mat=[0, 0; 0, 0; 0, 0; 0, 0]  dR5mat=[0, 0; 0, 0; 0, 0; 0, 0]  prm_age_modeling=simscape.enum.tablebattery.prm_age_modeling.equation  storage_dt_age_vec=[0] d  storage_T_age_vec=[273] K  prm_age_OCV=simscape.enum.tablebattery.prm_age_OCV.OCV  OCV_age=0.9  SOC_age=0.6  prm_age_resistance=simscape.enum.tablebattery.prm_age.disabled  OCV_scaling_age_resistance=2.2134e6  OCV_offset_age_resistance=1.632e6  temp_exp_age_resistance=0.515833569 V  t_exp_age_resistance=0.75  T_age_vec_resistance=[273.15, 298.15, 323.15] K  dt_age_vec_resistance=[0, 90, 180, 270] d  dR0_age_vec=[0, 0, 0]  t_meas_dR0_age=100 d  dR0_age_mat=[0, 0, 0; 0, 0, 0; 0, 0, 0; 0, 0, 0]  prm_age_capacity=simscape.enum.tablebattery.prm_age.disabled  OCV_scaling_age_capacity=1.5097e07  OCV_offset_age_capacity=8.3625e06  temp_exp_age_capacity=0.6011 V  t_exp_age_capacity=0.75  T_age_vec_capacity=[273.15, 298.15, 323.15] K  dt_age_vec_capacity=[0, 90, 180, 270] d  dAH_age_vec=[0, 0, 0]  t_meas_dAH_age=100 d  dAH_age_mat=[0, 0, 0; 0, 0, 0; 0, 0, 0; 0, 0, 0]  thermal_port=simscape.enum.thermaleffects.omit  temperature=298.15 K  thermal_mass=100 J/K  i_specify=off  i_priority=None  i=0 A  i_nominal_specify=off  i_nominal_value=1  i_nominal_unit=A  v_specify=off  v_priority=None  v=0 V  v_nominal_specify=off  v_nominal_value=1  v_nominal_unit=V  stateOfCharge_specify=on  stateOfCharge_priority=High  stateOfCharge=1  stateOfCharge_nominal_specify=off  stateOfCharge_nominal_value=1  stateOfCharge_nominal_unit=1  num_cycles_specify=off  num_cycles_priority=High  num_cycles=0  num_cycles_nominal_specify=off  num_cycles_nominal_value=1  num_cycles_nominal_unit=1  cell_temperature_specify=off  cell_temperature_priority=High  cell_temperature=298.15 K  cell_temperature_nominal_specify=off  cell_temperature_nominal_value=1  cell_temperature_nominal_unit=K
      V0_mat=|
      | [3.0263, 3.218033, 3.364889, 3.493933, 3.610678, 3.733744, 3.85405, 3.950717, 4.040478, 4.0819;
      |  3.0376, 3.2248, 3.370311, 3.498533, 3.615311, 3.736956, 3.845633, 3.929256, 4.040056, 4.0821;
      |  3.0439, 3.227633, 3.3731, 3.5007, 3.616611, 3.737589, 3.8457, 3.9287, 4.039133, 4.0826;
      |  3.0283, 3.217989, 3.364589, 3.493767, 3.609467, 3.731156, 3.8417, 3.925833, 4.036322, 4.0821]' V
      R0_mat=|
      | [0.011867, 0.008993, 0.007674, 0.006911, 0.006648, 0.006648, 0.006528, 0.006157, 0.005996, 0.0073;
      |  0.0109, 0.006456, 0.005381, 0.005078, 0.005, 0.005044, 0.005511, 0.006407, 0.006522, 0.005367;
      |  0.0102, 0.007978, 0.006793, 0.0062, 0.006033, 0.005441, 0.0051, 0.005707, 0.005037, 0.005067;
      |  0.0101, 0.007759, 0.006637, 0.006022, 0.005741, 0.005667, 0.005311, 0.004911, 0.005859, 0.004733]' Ohm
      R1_mat=|
      | [0.007451, 0.008294, 0.007745, 0.007391;
      |  0.003783, 0.00363, 0.004415, 0.004051;
      |  0.002841, 0.00298, 0.003698, 0.003391;
      |  0.003185, 0.002661, 0.003493, 0.00379;
      |  0.00379, 0.003147, 0.004204, 0.004229;
      |  0.004015, 0.003677, 0.004233, 0.004481;
      |  0.003791, 0.004051, 0.003886, 0.004189;
      |  0.003416, 0.004883, 0.004387, 0.003743;
      |  0.00328, 0.005238, 0.003472, 0.004883;
      |  0.004816, 0.004218, 0.003847, 0.003891] Ohm
      tau1_mat=|
      | [8.156247, 6.866126, 6.747335, 6.573366;
      |  6.436096, 6.88158, 6.206576, 5.30011;
      |  7.074429, 7.267109, 6.564215, 5.759928;
      |  8.61232, 7.062398, 6.553799, 7.485573;
      |  10.88135, 8.569373, 8.681328, 8.99043;
      |  11.88702, 10.35435, 10.74073, 9.985533;
      |  11.15433, 10.61987, 10.52072, 10.95124;
      |  10.33388, 9.573709, 9.987626, 10.94588;
      |  9.883806, 9.219359, 8.513241, 9.109378;
      |  11.2706, 10.03414, 9.643065, 10.06297] s
      R2_mat=|
      | [0.040653, 0.04799, 0.046915, 0.044404;
      |  0.026828, 0.033189, 0.032279, 0.030363;
      |  0.019744, 0.025225, 0.021211, 0.019613;
      |  0.012414, 0.014827, 0.017004, 0.016763;
      |  0.007363, 0.008356, 0.01135, 0.010173;
      |  0.005882, 0.007703, 0.006532, 0.005526;
      |  0.006739, 0.007058, 0.006772, 0.005603;
      |  0.008222, 0.004287, 0.009601, 0.005034;
      |  0.008985, 0.007821, 0.008932, 0.006662;
      |  0.004704, 0.003171, 0.002422, 0.004036] Ohm
      tau2_mat=|
      | [131.6948, 137.0217, 141.2851, 129.3807;
      |  146.2759, 158.6208, 157.255, 143.944;
      |  158.5443, 177.3225, 156.7434, 144.0735;
      |  144.8009, 123.279, 145.0945, 176.1753;
      |  158.7596, 137.3241, 203.2495, 189.2199;
      |  149.8847, 154.5014, 161.1061, 146.3519;
      |  135.3572, 173.7062, 166.0613, 159.34;
      |  123.823, 144.5727, 209.652, 117.4544;
      |  111.7616, 98.04929, 114.3433, 98.05822;
      |  125.3862, 75.97092, 110.7081, 120.3015] s
      settings: InternalSimscapePortConfiguration="{\"Bottom\":[],\"Left\":[{\"id\":\"p\",\"label\":\"+\",\"type\":\"foundation.electrical.electrical\"}],\"Right\":[{\"id\":\"n\",\"label\":\"-\",\"type\":\"foundation.electrical.electrical\"}],\"Top\":[]}"
      settings: LibrarySourceBlock=|
      | batt_lib/Cells/Battery
      | (Table-Based)
  Battery (Table-Based)3 : batteryecm_lib/Battery (Table-Based)  SOC_vec=[0.1, 0.188889, 0.277778, 0.366667, 0.455556, 0.544444, 0.633333, 0.722222, 0.811111, 0.9]  T_dependence=simscape.enum.tablebattery.temperature_dependence.yes  prm_dir=simscape.enum.tablebattery.prm_dir.noCurrentDirectionality  T_vec=[30, 32.5, 35, 38] degC  V0_mat=|  V0_vec=[3.5057, 3.566, 3.6337, 3.7127, 3.9259, 4.0777, 4.1928] V  V_range=[0, inf] V  R0_mat=|  R0_vec=[.0085, .0085, .0087, .0082, .0083, .0085, .0085] Ohm  R0_dis_mat=[.0117, .0085, .009; .011, .0085, .009; .0114, .0087, .0092; .0107, .0082, .0088; .0107, .0083, .0091; .0113, .0085, .0089; .0116, .0085, .0089] Ohm  R0_dis_vec=[.0085, .0085, .0087, .0082, .0083, .0085, .0085] Ohm  R0_ch_mat=[.0117, .0085, .009; .011, .0085, .009; .0114, .0087, .0092; .0107, .0082, .0088; .0107, .0083, .0091; .0113, .0085, .0089; .0116, .0085, .0089] Ohm  R0_ch_vec=[.0085, .0085, .0087, .0082, .0083, .0085, .0085] Ohm  AH=5 A*hr  prm_leak=simscape.enum.tablebattery.prm_leak.disabled  Rleak_vec=[8000, 7000, 6000] Ohm  Rleak=7e3 Ohm  extrapolation_option=simscape.enum.extrapolation.nearest  SOC_port=simscape.enum.tablebattery.enable.no  prm_dyn=simscape.enum.tablebattery.prm_dyn.rc2  R1_mat=|  R1_vec=[.0029, .0024, .0026, .0016, .0023, .0018, .0017] Ohm  tau1_mat=|  tau1_vec=[36, 45, 105, 29, 77, 33, 39] s  R2_mat=|  R2_vec=[.0029, .0024, .0026, .0016, .0023, .0018, .0017] Ohm  tau2_mat=|  tau2_vec=[36, 45, 105, 29, 77, 33, 39] s  R3_mat=[.0109, .0029, .0013; .0069, .0024, .0012; .0047, .0026, .0013; .0034, .0016, .001; .0033, .0023, .0014; .0033, .0018, .0011; .0028, .0017, .0011] Ohm  R3_vec=[.0029, .0024, .0026, .0016, .0023, .0018, .0017] Ohm  tau3_mat=[20, 36, 39; 31, 45, 39; 109, 105, 61; 36, 29, 26; 59, 77, 67; 40, 33, 29; 25, 39, 33] s  tau3_vec=[36, 45, 105, 29, 77, 33, 39] s  R4_mat=[.0109, .0029, .0013; .0069, .0024, .0012; .0047, .0026, .0013; .0034, .0016, .001; .0033, .0023, .0014; .0033, .0018, .0011; .0028, .0017, .0011] Ohm  R4_vec=[.0029, .0024, .0026, .0016, .0023, .0018, .0017] Ohm  tau4_mat=[20, 36, 39; 31, 45, 39; 109, 105, 61; 36, 29, 26; 59, 77, 67; 40, 33, 29; 25, 39, 33] s  tau4_vec=[36, 45, 105, 29, 77, 33, 39] s  R5_mat=[.0109, .0029, .0013; .0069, .0024, .0012; .0047, .0026, .0013; .0034, .0016, .001; .0033, .0023, .0014; .0033, .0018, .0011; .0028, .0017, .0011] Ohm  R5_vec=[.0029, .0024, .0026, .0016, .0023, .0018, .0017] Ohm  tau5_mat=[20, 36, 39; 31, 45, 39; 109, 105, 61; 36, 29, 26; 59, 77, 67; 40, 33, 29; 25, 39, 33] s  tau5_vec=[36, 45, 105, 29, 77, 33, 39] s  prm_fade=simscape.enum.tablebattery.prm_fade.disabled  N0=100  dV0=0  dR0=0  dAH=0  dRleak=0  dR1=0  dR2=0  dR3=0  dR4=0  dR5=0  N0vec=[0, 100, 200, 300]  Tfadevec=[298.15, 323.15] K  dV0vec=[0, 0, 0, 0]  dR0vec=[0, 0, 0, 0]  dAHvec=[0, 0, 0, 0]  dRleakvec=[0, 0, 0, 0]  dR1vec=[0, 0, 0, 0]  dR2vec=[0, 0, 0, 0]  dR3vec=[0, 0, 0, 0]  dR4vec=[0, 0, 0, 0]  dR5vec=[0, 0, 0, 0]  dV0mat=[0, 0; 0, 0; 0, 0; 0, 0]  dR0mat=[0, 0; 0, 0; 0, 0; 0, 0]  dAHmat=[0, 0; 0, 0; 0, 0; 0, 0]  dRleakmat=[0, 0; 0, 0; 0, 0; 0, 0]  dR1mat=[0, 0; 0, 0; 0, 0; 0, 0]  dR2mat=[0, 0; 0, 0; 0, 0; 0, 0]  dR3mat=[0, 0; 0, 0; 0, 0; 0, 0]  dR4mat=[0, 0; 0, 0; 0, 0; 0, 0]  dR5mat=[0, 0; 0, 0; 0, 0; 0, 0]  prm_age_modeling=simscape.enum.tablebattery.prm_age_modeling.equation  storage_dt_age_vec=[0] d  storage_T_age_vec=[273] K  prm_age_OCV=simscape.enum.tablebattery.prm_age_OCV.OCV  OCV_age=0.9  SOC_age=0.6  prm_age_resistance=simscape.enum.tablebattery.prm_age.disabled  OCV_scaling_age_resistance=2.2134e6  OCV_offset_age_resistance=1.632e6  temp_exp_age_resistance=0.515833569 V  t_exp_age_resistance=0.75  T_age_vec_resistance=[273.15, 298.15, 323.15] K  dt_age_vec_resistance=[0, 90, 180, 270] d  dR0_age_vec=[0, 0, 0]  t_meas_dR0_age=100 d  dR0_age_mat=[0, 0, 0; 0, 0, 0; 0, 0, 0; 0, 0, 0]  prm_age_capacity=simscape.enum.tablebattery.prm_age.disabled  OCV_scaling_age_capacity=1.5097e07  OCV_offset_age_capacity=8.3625e06  temp_exp_age_capacity=0.6011 V  t_exp_age_capacity=0.75  T_age_vec_capacity=[273.15, 298.15, 323.15] K  dt_age_vec_capacity=[0, 90, 180, 270] d  dAH_age_vec=[0, 0, 0]  t_meas_dAH_age=100 d  dAH_age_mat=[0, 0, 0; 0, 0, 0; 0, 0, 0; 0, 0, 0]  thermal_port=simscape.enum.thermaleffects.omit  temperature=298.15 K  thermal_mass=100 J/K  i_specify=off  i_priority=None  i=0 A  i_nominal_specify=off  i_nominal_value=1  i_nominal_unit=A  v_specify=off  v_priority=None  v=0 V  v_nominal_specify=off  v_nominal_value=1  v_nominal_unit=V  stateOfCharge_specify=on  stateOfCharge_priority=High  stateOfCharge=1  stateOfCharge_nominal_specify=off  stateOfCharge_nominal_value=1  stateOfCharge_nominal_unit=1  num_cycles_specify=off  num_cycles_priority=High  num_cycles=0  num_cycles_nominal_specify=off  num_cycles_nominal_value=1  num_cycles_nominal_unit=1  cell_temperature_specify=off  cell_temperature_priority=High  cell_temperature=298.15 K  cell_temperature_nominal_specify=off  cell_temperature_nominal_value=1  cell_temperature_nominal_unit=K
      V0_mat=|
      | [3.0263, 3.218033, 3.364889, 3.493933, 3.610678, 3.733744, 3.85405, 3.950717, 4.040478, 4.0819;
      |  3.0376, 3.2248, 3.370311, 3.498533, 3.615311, 3.736956, 3.845633, 3.929256, 4.040056, 4.0821;
      |  3.0439, 3.227633, 3.3731, 3.5007, 3.616611, 3.737589, 3.8457, 3.9287, 4.039133, 4.0826;
      |  3.0283, 3.217989, 3.364589, 3.493767, 3.609467, 3.731156, 3.8417, 3.925833, 4.036322, 4.0821]' V
      R0_mat=|
      | [0.011867, 0.008993, 0.007674, 0.006911, 0.006648, 0.006648, 0.006528, 0.006157, 0.005996, 0.0073;
      |  0.0109, 0.006456, 0.005381, 0.005078, 0.005, 0.005044, 0.005511, 0.006407, 0.006522, 0.005367;
      |  0.0102, 0.007978, 0.006793, 0.0062, 0.006033, 0.005441, 0.0051, 0.005707, 0.005037, 0.005067;
      |  0.0101, 0.007759, 0.006637, 0.006022, 0.005741, 0.005667, 0.005311, 0.004911, 0.005859, 0.004733]' Ohm
      R1_mat=|
      | [0.007451, 0.008294, 0.007745, 0.007391;
      |  0.003783, 0.00363, 0.004415, 0.004051;
      |  0.002841, 0.00298, 0.003698, 0.003391;
      |  0.003185, 0.002661, 0.003493, 0.00379;
      |  0.00379, 0.003147, 0.004204, 0.004229;
      |  0.004015, 0.003677, 0.004233, 0.004481;
      |  0.003791, 0.004051, 0.003886, 0.004189;
      |  0.003416, 0.004883, 0.004387, 0.003743;
      |  0.00328, 0.005238, 0.003472, 0.004883;
      |  0.004816, 0.004218, 0.003847, 0.003891] Ohm
      tau1_mat=|
      | [8.156247, 6.866126, 6.747335, 6.573366;
      |  6.436096, 6.88158, 6.206576, 5.30011;
      |  7.074429, 7.267109, 6.564215, 5.759928;
      |  8.61232, 7.062398, 6.553799, 7.485573;
      |  10.88135, 8.569373, 8.681328, 8.99043;
      |  11.88702, 10.35435, 10.74073, 9.985533;
      |  11.15433, 10.61987, 10.52072, 10.95124;
      |  10.33388, 9.573709, 9.987626, 10.94588;
      |  9.883806, 9.219359, 8.513241, 9.109378;
      |  11.2706, 10.03414, 9.643065, 10.06297] s
      R2_mat=|
      | [0.040653, 0.04799, 0.046915, 0.044404;
      |  0.026828, 0.033189, 0.032279, 0.030363;
      |  0.019744, 0.025225, 0.021211, 0.019613;
      |  0.012414, 0.014827, 0.017004, 0.016763;
      |  0.007363, 0.008356, 0.01135, 0.010173;
      |  0.005882, 0.007703, 0.006532, 0.005526;
      |  0.006739, 0.007058, 0.006772, 0.005603;
      |  0.008222, 0.004287, 0.009601, 0.005034;
      |  0.008985, 0.007821, 0.008932, 0.006662;
      |  0.004704, 0.003171, 0.002422, 0.004036] Ohm
      tau2_mat=|
      | [131.6948, 137.0217, 141.2851, 129.3807;
      |  146.2759, 158.6208, 157.255, 143.944;
      |  158.5443, 177.3225, 156.7434, 144.0735;
      |  144.8009, 123.279, 145.0945, 176.1753;
      |  158.7596, 137.3241, 203.2495, 189.2199;
      |  149.8847, 154.5014, 161.1061, 146.3519;
      |  135.3572, 173.7062, 166.0613, 159.34;
      |  123.823, 144.5727, 209.652, 117.4544;
      |  111.7616, 98.04929, 114.3433, 98.05822;
      |  125.3862, 75.97092, 110.7081, 120.3015] s
      settings: InternalSimscapePortConfiguration="{\"Bottom\":[],\"Left\":[{\"id\":\"p\",\"label\":\"+\",\"type\":\"foundation.electrical.electrical\"}],\"Right\":[{\"id\":\"n\",\"label\":\"-\",\"type\":\"foundation.electrical.electrical\"}],\"Top\":[]}"
      settings: LibrarySourceBlock=|
      | batt_lib/Cells/Battery
      | (Table-Based)
  Battery (Table-Based)30 : batteryecm_lib/Battery (Table-Based)  SOC_vec=[0.1, 0.188889, 0.277778, 0.366667, 0.455556, 0.544444, 0.633333, 0.722222, 0.811111, 0.9]  T_dependence=simscape.enum.tablebattery.temperature_dependence.yes  prm_dir=simscape.enum.tablebattery.prm_dir.noCurrentDirectionality  T_vec=[30, 32.5, 35, 38] degC  V0_mat=|  V0_vec=[3.5057, 3.566, 3.6337, 3.7127, 3.9259, 4.0777, 4.1928] V  V_range=[0, inf] V  R0_mat=|  R0_vec=[.0085, .0085, .0087, .0082, .0083, .0085, .0085] Ohm  R0_dis_mat=[.0117, .0085, .009; .011, .0085, .009; .0114, .0087, .0092; .0107, .0082, .0088; .0107, .0083, .0091; .0113, .0085, .0089; .0116, .0085, .0089] Ohm  R0_dis_vec=[.0085, .0085, .0087, .0082, .0083, .0085, .0085] Ohm  R0_ch_mat=[.0117, .0085, .009; .011, .0085, .009; .0114, .0087, .0092; .0107, .0082, .0088; .0107, .0083, .0091; .0113, .0085, .0089; .0116, .0085, .0089] Ohm  R0_ch_vec=[.0085, .0085, .0087, .0082, .0083, .0085, .0085] Ohm  AH=5 A*hr  prm_leak=simscape.enum.tablebattery.prm_leak.disabled  Rleak_vec=[8000, 7000, 6000] Ohm  Rleak=7e3 Ohm  extrapolation_option=simscape.enum.extrapolation.nearest  SOC_port=simscape.enum.tablebattery.enable.no  prm_dyn=simscape.enum.tablebattery.prm_dyn.rc2  R1_mat=|  R1_vec=[.0029, .0024, .0026, .0016, .0023, .0018, .0017] Ohm  tau1_mat=|  tau1_vec=[36, 45, 105, 29, 77, 33, 39] s  R2_mat=|  R2_vec=[.0029, .0024, .0026, .0016, .0023, .0018, .0017] Ohm  tau2_mat=|  tau2_vec=[36, 45, 105, 29, 77, 33, 39] s  R3_mat=[.0109, .0029, .0013; .0069, .0024, .0012; .0047, .0026, .0013; .0034, .0016, .001; .0033, .0023, .0014; .0033, .0018, .0011; .0028, .0017, .0011] Ohm  R3_vec=[.0029, .0024, .0026, .0016, .0023, .0018, .0017] Ohm  tau3_mat=[20, 36, 39; 31, 45, 39; 109, 105, 61; 36, 29, 26; 59, 77, 67; 40, 33, 29; 25, 39, 33] s  tau3_vec=[36, 45, 105, 29, 77, 33, 39] s  R4_mat=[.0109, .0029, .0013; .0069, .0024, .0012; .0047, .0026, .0013; .0034, .0016, .001; .0033, .0023, .0014; .0033, .0018, .0011; .0028, .0017, .0011] Ohm  R4_vec=[.0029, .0024, .0026, .0016, .0023, .0018, .0017] Ohm  tau4_mat=[20, 36, 39; 31, 45, 39; 109, 105, 61; 36, 29, 26; 59, 77, 67; 40, 33, 29; 25, 39, 33] s  tau4_vec=[36, 45, 105, 29, 77, 33, 39] s  R5_mat=[.0109, .0029, .0013; .0069, .0024, .0012; .0047, .0026, .0013; .0034, .0016, .001; .0033, .0023, .0014; .0033, .0018, .0011; .0028, .0017, .0011] Ohm  R5_vec=[.0029, .0024, .0026, .0016, .0023, .0018, .0017] Ohm  tau5_mat=[20, 36, 39; 31, 45, 39; 109, 105, 61; 36, 29, 26; 59, 77, 67; 40, 33, 29; 25, 39, 33] s  tau5_vec=[36, 45, 105, 29, 77, 33, 39] s  prm_fade=simscape.enum.tablebattery.prm_fade.disabled  N0=100  dV0=0  dR0=0  dAH=0  dRleak=0  dR1=0  dR2=0  dR3=0  dR4=0  dR5=0  N0vec=[0, 100, 200, 300]  Tfadevec=[298.15, 323.15] K  dV0vec=[0, 0, 0, 0]  dR0vec=[0, 0, 0, 0]  dAHvec=[0, 0, 0, 0]  dRleakvec=[0, 0, 0, 0]  dR1vec=[0, 0, 0, 0]  dR2vec=[0, 0, 0, 0]  dR3vec=[0, 0, 0, 0]  dR4vec=[0, 0, 0, 0]  dR5vec=[0, 0, 0, 0]  dV0mat=[0, 0; 0, 0; 0, 0; 0, 0]  dR0mat=[0, 0; 0, 0; 0, 0; 0, 0]  dAHmat=[0, 0; 0, 0; 0, 0; 0, 0]  dRleakmat=[0, 0; 0, 0; 0, 0; 0, 0]  dR1mat=[0, 0; 0, 0; 0, 0; 0, 0]  dR2mat=[0, 0; 0, 0; 0, 0; 0, 0]  dR3mat=[0, 0; 0, 0; 0, 0; 0, 0]  dR4mat=[0, 0; 0, 0; 0, 0; 0, 0]  dR5mat=[0, 0; 0, 0; 0, 0; 0, 0]  prm_age_modeling=simscape.enum.tablebattery.prm_age_modeling.equation  storage_dt_age_vec=[0] d  storage_T_age_vec=[273] K  prm_age_OCV=simscape.enum.tablebattery.prm_age_OCV.OCV  OCV_age=0.9  SOC_age=0.6  prm_age_resistance=simscape.enum.tablebattery.prm_age.disabled  OCV_scaling_age_resistance=2.2134e6  OCV_offset_age_resistance=1.632e6  temp_exp_age_resistance=0.515833569 V  t_exp_age_resistance=0.75  T_age_vec_resistance=[273.15, 298.15, 323.15] K  dt_age_vec_resistance=[0, 90, 180, 270] d  dR0_age_vec=[0, 0, 0]  t_meas_dR0_age=100 d  dR0_age_mat=[0, 0, 0; 0, 0, 0; 0, 0, 0; 0, 0, 0]  prm_age_capacity=simscape.enum.tablebattery.prm_age.disabled  OCV_scaling_age_capacity=1.5097e07  OCV_offset_age_capacity=8.3625e06  temp_exp_age_capacity=0.6011 V  t_exp_age_capacity=0.75  T_age_vec_capacity=[273.15, 298.15, 323.15] K  dt_age_vec_capacity=[0, 90, 180, 270] d  dAH_age_vec=[0, 0, 0]  t_meas_dAH_age=100 d  dAH_age_mat=[0, 0, 0; 0, 0, 0; 0, 0, 0; 0, 0, 0]  thermal_port=simscape.enum.thermaleffects.omit  temperature=298.15 K  thermal_mass=100 J/K  i_specify=off  i_priority=None  i=0 A  i_nominal_specify=off  i_nominal_value=1  i_nominal_unit=A  v_specify=off  v_priority=None  v=0 V  v_nominal_specify=off  v_nominal_value=1  v_nominal_unit=V  stateOfCharge_specify=on  stateOfCharge_priority=High  stateOfCharge=1  stateOfCharge_nominal_specify=off  stateOfCharge_nominal_value=1  stateOfCharge_nominal_unit=1  num_cycles_specify=off  num_cycles_priority=High  num_cycles=0  num_cycles_nominal_specify=off  num_cycles_nominal_value=1  num_cycles_nominal_unit=1  cell_temperature_specify=off  cell_temperature_priority=High  cell_temperature=298.15 K  cell_temperature_nominal_specify=off  cell_temperature_nominal_value=1  cell_temperature_nominal_unit=K
      V0_mat=|
      | [3.0263, 3.218033, 3.364889, 3.493933, 3.610678, 3.733744, 3.85405, 3.950717, 4.040478, 4.0819;
      |  3.0376, 3.2248, 3.370311, 3.498533, 3.615311, 3.736956, 3.845633, 3.929256, 4.040056, 4.0821;
      |  3.0439, 3.227633, 3.3731, 3.5007, 3.616611, 3.737589, 3.8457, 3.9287, 4.039133, 4.0826;
      |  3.0283, 3.217989, 3.364589, 3.493767, 3.609467, 3.731156, 3.8417, 3.925833, 4.036322, 4.0821]' V
      R0_mat=|
      | [0.011867, 0.008993, 0.007674, 0.006911, 0.006648, 0.006648, 0.006528, 0.006157, 0.005996, 0.0073;
      |  0.0109, 0.006456, 0.005381, 0.005078, 0.005, 0.005044, 0.005511, 0.006407, 0.006522, 0.005367;
      |  0.0102, 0.007978, 0.006793, 0.0062, 0.006033, 0.005441, 0.0051, 0.005707, 0.005037, 0.005067;
      |  0.0101, 0.007759, 0.006637, 0.006022, 0.005741, 0.005667, 0.005311, 0.004911, 0.005859, 0.004733]' Ohm
      R1_mat=|
      | [0.007451, 0.008294, 0.007745, 0.007391;
      |  0.003783, 0.00363, 0.004415, 0.004051;
      |  0.002841, 0.00298, 0.003698, 0.003391;
      |  0.003185, 0.002661, 0.003493, 0.00379;
      |  0.00379, 0.003147, 0.004204, 0.004229;
      |  0.004015, 0.003677, 0.004233, 0.004481;
      |  0.003791, 0.004051, 0.003886, 0.004189;
      |  0.003416, 0.004883, 0.004387, 0.003743;
      |  0.00328, 0.005238, 0.003472, 0.004883;
      |  0.004816, 0.004218, 0.003847, 0.003891] Ohm
      tau1_mat=|
      | [8.156247, 6.866126, 6.747335, 6.573366;
      |  6.436096, 6.88158, 6.206576, 5.30011;
      |  7.074429, 7.267109, 6.564215, 5.759928;
      |  8.61232, 7.062398, 6.553799, 7.485573;
      |  10.88135, 8.569373, 8.681328, 8.99043;
      |  11.88702, 10.35435, 10.74073, 9.985533;
      |  11.15433, 10.61987, 10.52072, 10.95124;
      |  10.33388, 9.573709, 9.987626, 10.94588;
      |  9.883806, 9.219359, 8.513241, 9.109378;
      |  11.2706, 10.03414, 9.643065, 10.06297] s
      R2_mat=|
      | [0.040653, 0.04799, 0.046915, 0.044404;
      |  0.026828, 0.033189, 0.032279, 0.030363;
      |  0.019744, 0.025225, 0.021211, 0.019613;
      |  0.012414, 0.014827, 0.017004, 0.016763;
      |  0.007363, 0.008356, 0.01135, 0.010173;
      |  0.005882, 0.007703, 0.006532, 0.005526;
      |  0.006739, 0.007058, 0.006772, 0.005603;
      |  0.008222, 0.004287, 0.009601, 0.005034;
      |  0.008985, 0.007821, 0.008932, 0.006662;
      |  0.004704, 0.003171, 0.002422, 0.004036] Ohm
      tau2_mat=|
      | [131.6948, 137.0217, 141.2851, 129.3807;
      |  146.2759, 158.6208, 157.255, 143.944;
      |  158.5443, 177.3225, 156.7434, 144.0735;
      |  144.8009, 123.279, 145.0945, 176.1753;
      |  158.7596, 137.3241, 203.2495, 189.2199;
      |  149.8847, 154.5014, 161.1061, 146.3519;
      |  135.3572, 173.7062, 166.0613, 159.34;
      |  123.823, 144.5727, 209.652, 117.4544;
      |  111.7616, 98.04929, 114.3433, 98.05822;
      |  125.3862, 75.97092, 110.7081, 120.3015] s
      settings: InternalSimscapePortConfiguration="{\"Bottom\":[],\"Left\":[{\"id\":\"p\",\"label\":\"+\",\"type\":\"foundation.electrical.electrical\"}],\"Right\":[{\"id\":\"n\",\"label\":\"-\",\"type\":\"foundation.electrical.electrical\"}],\"Top\":[]}"
      settings: LibrarySourceBlock=|
      | batt_lib/Cells/Battery
      | (Table-Based)
  Battery (Table-Based)31 : batteryecm_lib/Battery (Table-Based)  SOC_vec=[0.1, 0.188889, 0.277778, 0.366667, 0.455556, 0.544444, 0.633333, 0.722222, 0.811111, 0.9]  T_dependence=simscape.enum.tablebattery.temperature_dependence.yes  prm_dir=simscape.enum.tablebattery.prm_dir.noCurrentDirectionality  T_vec=[30, 32.5, 35, 38] degC  V0_mat=|  V0_vec=[3.5057, 3.566, 3.6337, 3.7127, 3.9259, 4.0777, 4.1928] V  V_range=[0, inf] V  R0_mat=|  R0_vec=[.0085, .0085, .0087, .0082, .0083, .0085, .0085] Ohm  R0_dis_mat=[.0117, .0085, .009; .011, .0085, .009; .0114, .0087, .0092; .0107, .0082, .0088; .0107, .0083, .0091; .0113, .0085, .0089; .0116, .0085, .0089] Ohm  R0_dis_vec=[.0085, .0085, .0087, .0082, .0083, .0085, .0085] Ohm  R0_ch_mat=[.0117, .0085, .009; .011, .0085, .009; .0114, .0087, .0092; .0107, .0082, .0088; .0107, .0083, .0091; .0113, .0085, .0089; .0116, .0085, .0089] Ohm  R0_ch_vec=[.0085, .0085, .0087, .0082, .0083, .0085, .0085] Ohm  AH=5 A*hr  prm_leak=simscape.enum.tablebattery.prm_leak.disabled  Rleak_vec=[8000, 7000, 6000] Ohm  Rleak=7e3 Ohm  extrapolation_option=simscape.enum.extrapolation.nearest  SOC_port=simscape.enum.tablebattery.enable.no  prm_dyn=simscape.enum.tablebattery.prm_dyn.rc2  R1_mat=|  R1_vec=[.0029, .0024, .0026, .0016, .0023, .0018, .0017] Ohm  tau1_mat=|  tau1_vec=[36, 45, 105, 29, 77, 33, 39] s  R2_mat=|  R2_vec=[.0029, .0024, .0026, .0016, .0023, .0018, .0017] Ohm  tau2_mat=|  tau2_vec=[36, 45, 105, 29, 77, 33, 39] s  R3_mat=[.0109, .0029, .0013; .0069, .0024, .0012; .0047, .0026, .0013; .0034, .0016, .001; .0033, .0023, .0014; .0033, .0018, .0011; .0028, .0017, .0011] Ohm  R3_vec=[.0029, .0024, .0026, .0016, .0023, .0018, .0017] Ohm  tau3_mat=[20, 36, 39; 31, 45, 39; 109, 105, 61; 36, 29, 26; 59, 77, 67; 40, 33, 29; 25, 39, 33] s  tau3_vec=[36, 45, 105, 29, 77, 33, 39] s  R4_mat=[.0109, .0029, .0013; .0069, .0024, .0012; .0047, .0026, .0013; .0034, .0016, .001; .0033, .0023, .0014; .0033, .0018, .0011; .0028, .0017, .0011] Ohm  R4_vec=[.0029, .0024, .0026, .0016, .0023, .0018, .0017] Ohm  tau4_mat=[20, 36, 39; 31, 45, 39; 109, 105, 61; 36, 29, 26; 59, 77, 67; 40, 33, 29; 25, 39, 33] s  tau4_vec=[36, 45, 105, 29, 77, 33, 39] s  R5_mat=[.0109, .0029, .0013; .0069, .0024, .0012; .0047, .0026, .0013; .0034, .0016, .001; .0033, .0023, .0014; .0033, .0018, .0011; .0028, .0017, .0011] Ohm  R5_vec=[.0029, .0024, .0026, .0016, .0023, .0018, .0017] Ohm  tau5_mat=[20, 36, 39; 31, 45, 39; 109, 105, 61; 36, 29, 26; 59, 77, 67; 40, 33, 29; 25, 39, 33] s  tau5_vec=[36, 45, 105, 29, 77, 33, 39] s  prm_fade=simscape.enum.tablebattery.prm_fade.disabled  N0=100  dV0=0  dR0=0  dAH=0  dRleak=0  dR1=0  dR2=0  dR3=0  dR4=0  dR5=0  N0vec=[0, 100, 200, 300]  Tfadevec=[298.15, 323.15] K  dV0vec=[0, 0, 0, 0]  dR0vec=[0, 0, 0, 0]  dAHvec=[0, 0, 0, 0]  dRleakvec=[0, 0, 0, 0]  dR1vec=[0, 0, 0, 0]  dR2vec=[0, 0, 0, 0]  dR3vec=[0, 0, 0, 0]  dR4vec=[0, 0, 0, 0]  dR5vec=[0, 0, 0, 0]  dV0mat=[0, 0; 0, 0; 0, 0; 0, 0]  dR0mat=[0, 0; 0, 0; 0, 0; 0, 0]  dAHmat=[0, 0; 0, 0; 0, 0; 0, 0]  dRleakmat=[0, 0; 0, 0; 0, 0; 0, 0]  dR1mat=[0, 0; 0, 0; 0, 0; 0, 0]  dR2mat=[0, 0; 0, 0; 0, 0; 0, 0]  dR3mat=[0, 0; 0, 0; 0, 0; 0, 0]  dR4mat=[0, 0; 0, 0; 0, 0; 0, 0]  dR5mat=[0, 0; 0, 0; 0, 0; 0, 0]  prm_age_modeling=simscape.enum.tablebattery.prm_age_modeling.equation  storage_dt_age_vec=[0] d  storage_T_age_vec=[273] K  prm_age_OCV=simscape.enum.tablebattery.prm_age_OCV.OCV  OCV_age=0.9  SOC_age=0.6  prm_age_resistance=simscape.enum.tablebattery.prm_age.disabled  OCV_scaling_age_resistance=2.2134e6  OCV_offset_age_resistance=1.632e6  temp_exp_age_resistance=0.515833569 V  t_exp_age_resistance=0.75  T_age_vec_resistance=[273.15, 298.15, 323.15] K  dt_age_vec_resistance=[0, 90, 180, 270] d  dR0_age_vec=[0, 0, 0]  t_meas_dR0_age=100 d  dR0_age_mat=[0, 0, 0; 0, 0, 0; 0, 0, 0; 0, 0, 0]  prm_age_capacity=simscape.enum.tablebattery.prm_age.disabled  OCV_scaling_age_capacity=1.5097e07  OCV_offset_age_capacity=8.3625e06  temp_exp_age_capacity=0.6011 V  t_exp_age_capacity=0.75  T_age_vec_capacity=[273.15, 298.15, 323.15] K  dt_age_vec_capacity=[0, 90, 180, 270] d  dAH_age_vec=[0, 0, 0]  t_meas_dAH_age=100 d  dAH_age_mat=[0, 0, 0; 0, 0, 0; 0, 0, 0; 0, 0, 0]  thermal_port=simscape.enum.thermaleffects.omit  temperature=298.15 K  thermal_mass=100 J/K  i_specify=off  i_priority=None  i=0 A  i_nominal_specify=off  i_nominal_value=1  i_nominal_unit=A  v_specify=off  v_priority=None  v=0 V  v_nominal_specify=off  v_nominal_value=1  v_nominal_unit=V  stateOfCharge_specify=on  stateOfCharge_priority=High  stateOfCharge=1  stateOfCharge_nominal_specify=off  stateOfCharge_nominal_value=1  stateOfCharge_nominal_unit=1  num_cycles_specify=off  num_cycles_priority=High  num_cycles=0  num_cycles_nominal_specify=off  num_cycles_nominal_value=1  num_cycles_nominal_unit=1  cell_temperature_specify=off  cell_temperature_priority=High  cell_temperature=298.15 K  cell_temperature_nominal_specify=off  cell_temperature_nominal_value=1  cell_temperature_nominal_unit=K
      V0_mat=|
      | [3.0263, 3.218033, 3.364889, 3.493933, 3.610678, 3.733744, 3.85405, 3.950717, 4.040478, 4.0819;
      |  3.0376, 3.2248, 3.370311, 3.498533, 3.615311, 3.736956, 3.845633, 3.929256, 4.040056, 4.0821;
      |  3.0439, 3.227633, 3.3731, 3.5007, 3.616611, 3.737589, 3.8457, 3.9287, 4.039133, 4.0826;
      |  3.0283, 3.217989, 3.364589, 3.493767, 3.609467, 3.731156, 3.8417, 3.925833, 4.036322, 4.0821]' V
      R0_mat=|
      | [0.011867, 0.008993, 0.007674, 0.006911, 0.006648, 0.006648, 0.006528, 0.006157, 0.005996, 0.0073;
      |  0.0109, 0.006456, 0.005381, 0.005078, 0.005, 0.005044, 0.005511, 0.006407, 0.006522, 0.005367;
      |  0.0102, 0.007978, 0.006793, 0.0062, 0.006033, 0.005441, 0.0051, 0.005707, 0.005037, 0.005067;
      |  0.0101, 0.007759, 0.006637, 0.006022, 0.005741, 0.005667, 0.005311, 0.004911, 0.005859, 0.004733]' Ohm
      R1_mat=|
      | [0.007451, 0.008294, 0.007745, 0.007391;
      |  0.003783, 0.00363, 0.004415, 0.004051;
      |  0.002841, 0.00298, 0.003698, 0.003391;
      |  0.003185, 0.002661, 0.003493, 0.00379;
      |  0.00379, 0.003147, 0.004204, 0.004229;
      |  0.004015, 0.003677, 0.004233, 0.004481;
      |  0.003791, 0.004051, 0.003886, 0.004189;
      |  0.003416, 0.004883, 0.004387, 0.003743;
      |  0.00328, 0.005238, 0.003472, 0.004883;
      |  0.004816, 0.004218, 0.003847, 0.003891] Ohm
      tau1_mat=|
      | [8.156247, 6.866126, 6.747335, 6.573366;
      |  6.436096, 6.88158, 6.206576, 5.30011;
      |  7.074429, 7.267109, 6.564215, 5.759928;
      |  8.61232, 7.062398, 6.553799, 7.485573;
      |  10.88135, 8.569373, 8.681328, 8.99043;
      |  11.88702, 10.35435, 10.74073, 9.985533;
      |  11.15433, 10.61987, 10.52072, 10.95124;
      |  10.33388, 9.573709, 9.987626, 10.94588;
      |  9.883806, 9.219359, 8.513241, 9.109378;
      |  11.2706, 10.03414, 9.643065, 10.06297] s
      R2_mat=|
      | [0.040653, 0.04799, 0.046915, 0.044404;
      |  0.026828, 0.033189, 0.032279, 0.030363;
      |  0.019744, 0.025225, 0.021211, 0.019613;
      |  0.012414, 0.014827, 0.017004, 0.016763;
      |  0.007363, 0.008356, 0.01135, 0.010173;
      |  0.005882, 0.007703, 0.006532, 0.005526;
      |  0.006739, 0.007058, 0.006772, 0.005603;
      |  0.008222, 0.004287, 0.009601, 0.005034;
      |  0.008985, 0.007821, 0.008932, 0.006662;
      |  0.004704, 0.003171, 0.002422, 0.004036] Ohm
      tau2_mat=|
      | [131.6948, 137.0217, 141.2851, 129.3807;
      |  146.2759, 158.6208, 157.255, 143.944;
      |  158.5443, 177.3225, 156.7434, 144.0735;
      |  144.8009, 123.279, 145.0945, 176.1753;
      |  158.7596, 137.3241, 203.2495, 189.2199;
      |  149.8847, 154.5014, 161.1061, 146.3519;
      |  135.3572, 173.7062, 166.0613, 159.34;
      |  123.823, 144.5727, 209.652, 117.4544;
      |  111.7616, 98.04929, 114.3433, 98.05822;
      |  125.3862, 75.97092, 110.7081, 120.3015] s
      settings: InternalSimscapePortConfiguration="{\"Bottom\":[],\"Left\":[{\"id\":\"p\",\"label\":\"+\",\"type\":\"foundation.electrical.electrical\"}],\"Right\":[{\"id\":\"n\",\"label\":\"-\",\"type\":\"foundation.electrical.electrical\"}],\"Top\":[]}"
      settings: LibrarySourceBlock=|
      | batt_lib/Cells/Battery
      | (Table-Based)
  Battery (Table-Based)32 : batteryecm_lib/Battery (Table-Based)  SOC_vec=[0.1, 0.188889, 0.277778, 0.366667, 0.455556, 0.544444, 0.633333, 0.722222, 0.811111, 0.9]  T_dependence=simscape.enum.tablebattery.temperature_dependence.yes  prm_dir=simscape.enum.tablebattery.prm_dir.noCurrentDirectionality  T_vec=[30, 32.5, 35, 38] degC  V0_mat=|  V0_vec=[3.5057, 3.566, 3.6337, 3.7127, 3.9259, 4.0777, 4.1928] V  V_range=[0, inf] V  R0_mat=|  R0_vec=[.0085, .0085, .0087, .0082, .0083, .0085, .0085] Ohm  R0_dis_mat=[.0117, .0085, .009; .011, .0085, .009; .0114, .0087, .0092; .0107, .0082, .0088; .0107, .0083, .0091; .0113, .0085, .0089; .0116, .0085, .0089] Ohm  R0_dis_vec=[.0085, .0085, .0087, .0082, .0083, .0085, .0085] Ohm  R0_ch_mat=[.0117, .0085, .009; .011, .0085, .009; .0114, .0087, .0092; .0107, .0082, .0088; .0107, .0083, .0091; .0113, .0085, .0089; .0116, .0085, .0089] Ohm  R0_ch_vec=[.0085, .0085, .0087, .0082, .0083, .0085, .0085] Ohm  AH=5 A*hr  prm_leak=simscape.enum.tablebattery.prm_leak.disabled  Rleak_vec=[8000, 7000, 6000] Ohm  Rleak=7e3 Ohm  extrapolation_option=simscape.enum.extrapolation.nearest  SOC_port=simscape.enum.tablebattery.enable.no  prm_dyn=simscape.enum.tablebattery.prm_dyn.rc2  R1_mat=|  R1_vec=[.0029, .0024, .0026, .0016, .0023, .0018, .0017] Ohm  tau1_mat=|  tau1_vec=[36, 45, 105, 29, 77, 33, 39] s  R2_mat=|  R2_vec=[.0029, .0024, .0026, .0016, .0023, .0018, .0017] Ohm  tau2_mat=|  tau2_vec=[36, 45, 105, 29, 77, 33, 39] s  R3_mat=[.0109, .0029, .0013; .0069, .0024, .0012; .0047, .0026, .0013; .0034, .0016, .001; .0033, .0023, .0014; .0033, .0018, .0011; .0028, .0017, .0011] Ohm  R3_vec=[.0029, .0024, .0026, .0016, .0023, .0018, .0017] Ohm  tau3_mat=[20, 36, 39; 31, 45, 39; 109, 105, 61; 36, 29, 26; 59, 77, 67; 40, 33, 29; 25, 39, 33] s  tau3_vec=[36, 45, 105, 29, 77, 33, 39] s  R4_mat=[.0109, .0029, .0013; .0069, .0024, .0012; .0047, .0026, .0013; .0034, .0016, .001; .0033, .0023, .0014; .0033, .0018, .0011; .0028, .0017, .0011] Ohm  R4_vec=[.0029, .0024, .0026, .0016, .0023, .0018, .0017] Ohm  tau4_mat=[20, 36, 39; 31, 45, 39; 109, 105, 61; 36, 29, 26; 59, 77, 67; 40, 33, 29; 25, 39, 33] s  tau4_vec=[36, 45, 105, 29, 77, 33, 39] s  R5_mat=[.0109, .0029, .0013; .0069, .0024, .0012; .0047, .0026, .0013; .0034, .0016, .001; .0033, .0023, .0014; .0033, .0018, .0011; .0028, .0017, .0011] Ohm  R5_vec=[.0029, .0024, .0026, .0016, .0023, .0018, .0017] Ohm  tau5_mat=[20, 36, 39; 31, 45, 39; 109, 105, 61; 36, 29, 26; 59, 77, 67; 40, 33, 29; 25, 39, 33] s  tau5_vec=[36, 45, 105, 29, 77, 33, 39] s  prm_fade=simscape.enum.tablebattery.prm_fade.disabled  N0=100  dV0=0  dR0=0  dAH=0  dRleak=0  dR1=0  dR2=0  dR3=0  dR4=0  dR5=0  N0vec=[0, 100, 200, 300]  Tfadevec=[298.15, 323.15] K  dV0vec=[0, 0, 0, 0]  dR0vec=[0, 0, 0, 0]  dAHvec=[0, 0, 0, 0]  dRleakvec=[0, 0, 0, 0]  dR1vec=[0, 0, 0, 0]  dR2vec=[0, 0, 0, 0]  dR3vec=[0, 0, 0, 0]  dR4vec=[0, 0, 0, 0]  dR5vec=[0, 0, 0, 0]  dV0mat=[0, 0; 0, 0; 0, 0; 0, 0]  dR0mat=[0, 0; 0, 0; 0, 0; 0, 0]  dAHmat=[0, 0; 0, 0; 0, 0; 0, 0]  dRleakmat=[0, 0; 0, 0; 0, 0; 0, 0]  dR1mat=[0, 0; 0, 0; 0, 0; 0, 0]  dR2mat=[0, 0; 0, 0; 0, 0; 0, 0]  dR3mat=[0, 0; 0, 0; 0, 0; 0, 0]  dR4mat=[0, 0; 0, 0; 0, 0; 0, 0]  dR5mat=[0, 0; 0, 0; 0, 0; 0, 0]  prm_age_modeling=simscape.enum.tablebattery.prm_age_modeling.equation  storage_dt_age_vec=[0] d  storage_T_age_vec=[273] K  prm_age_OCV=simscape.enum.tablebattery.prm_age_OCV.OCV  OCV_age=0.9  SOC_age=0.6  prm_age_resistance=simscape.enum.tablebattery.prm_age.disabled  OCV_scaling_age_resistance=2.2134e6  OCV_offset_age_resistance=1.632e6  temp_exp_age_resistance=0.515833569 V  t_exp_age_resistance=0.75  T_age_vec_resistance=[273.15, 298.15, 323.15] K  dt_age_vec_resistance=[0, 90, 180, 270] d  dR0_age_vec=[0, 0, 0]  t_meas_dR0_age=100 d  dR0_age_mat=[0, 0, 0; 0, 0, 0; 0, 0, 0; 0, 0, 0]  prm_age_capacity=simscape.enum.tablebattery.prm_age.disabled  OCV_scaling_age_capacity=1.5097e07  OCV_offset_age_capacity=8.3625e06  temp_exp_age_capacity=0.6011 V  t_exp_age_capacity=0.75  T_age_vec_capacity=[273.15, 298.15, 323.15] K  dt_age_vec_capacity=[0, 90, 180, 270] d  dAH_age_vec=[0, 0, 0]  t_meas_dAH_age=100 d  dAH_age_mat=[0, 0, 0; 0, 0, 0; 0, 0, 0; 0, 0, 0]  thermal_port=simscape.enum.thermaleffects.omit  temperature=298.15 K  thermal_mass=100 J/K  i_specify=off  i_priority=None  i=0 A  i_nominal_specify=off  i_nominal_value=1  i_nominal_unit=A  v_specify=off  v_priority=None  v=0 V  v_nominal_specify=off  v_nominal_value=1  v_nominal_unit=V  stateOfCharge_specify=on  stateOfCharge_priority=High  stateOfCharge=1  stateOfCharge_nominal_specify=off  stateOfCharge_nominal_value=1  stateOfCharge_nominal_unit=1  num_cycles_specify=off  num_cycles_priority=High  num_cycles=0  num_cycles_nominal_specify=off  num_cycles_nominal_value=1  num_cycles_nominal_unit=1  cell_temperature_specify=off  cell_temperature_priority=High  cell_temperature=298.15 K  cell_temperature_nominal_specify=off  cell_temperature_nominal_value=1  cell_temperature_nominal_unit=K
      V0_mat=|
      | [3.0263, 3.218033, 3.364889, 3.493933, 3.610678, 3.733744, 3.85405, 3.950717, 4.040478, 4.0819;
      |  3.0376, 3.2248, 3.370311, 3.498533, 3.615311, 3.736956, 3.845633, 3.929256, 4.040056, 4.0821;
      |  3.0439, 3.227633, 3.3731, 3.5007, 3.616611, 3.737589, 3.8457, 3.9287, 4.039133, 4.0826;
      |  3.0283, 3.217989, 3.364589, 3.493767, 3.609467, 3.731156, 3.8417, 3.925833, 4.036322, 4.0821]' V
      R0_mat=|
      | [0.011867, 0.008993, 0.007674, 0.006911, 0.006648, 0.006648, 0.006528, 0.006157, 0.005996, 0.0073;
      |  0.0109, 0.006456, 0.005381, 0.005078, 0.005, 0.005044, 0.005511, 0.006407, 0.006522, 0.005367;
      |  0.0102, 0.007978, 0.006793, 0.0062, 0.006033, 0.005441, 0.0051, 0.005707, 0.005037, 0.005067;
      |  0.0101, 0.007759, 0.006637, 0.006022, 0.005741, 0.005667, 0.005311, 0.004911, 0.005859, 0.004733]' Ohm
      R1_mat=|
      | [0.007451, 0.008294, 0.007745, 0.007391;
      |  0.003783, 0.00363, 0.004415, 0.004051;
      |  0.002841, 0.00298, 0.003698, 0.003391;
      |  0.003185, 0.002661, 0.003493, 0.00379;
      |  0.00379, 0.003147, 0.004204, 0.004229;
      |  0.004015, 0.003677, 0.004233, 0.004481;
      |  0.003791, 0.004051, 0.003886, 0.004189;
      |  0.003416, 0.004883, 0.004387, 0.003743;
      |  0.00328, 0.005238, 0.003472, 0.004883;
      |  0.004816, 0.004218, 0.003847, 0.003891] Ohm
      tau1_mat=|
      | [8.156247, 6.866126, 6.747335, 6.573366;
      |  6.436096, 6.88158, 6.206576, 5.30011;
      |  7.074429, 7.267109, 6.564215, 5.759928;
      |  8.61232, 7.062398, 6.553799, 7.485573;
      |  10.88135, 8.569373, 8.681328, 8.99043;
      |  11.88702, 10.35435, 10.74073, 9.985533;
      |  11.15433, 10.61987, 10.52072, 10.95124;
      |  10.33388, 9.573709, 9.987626, 10.94588;
      |  9.883806, 9.219359, 8.513241, 9.109378;
      |  11.2706, 10.03414, 9.643065, 10.06297] s
      R2_mat=|
      | [0.040653, 0.04799, 0.046915, 0.044404;
      |  0.026828, 0.033189, 0.032279, 0.030363;
      |  0.019744, 0.025225, 0.021211, 0.019613;
      |  0.012414, 0.014827, 0.017004, 0.016763;
      |  0.007363, 0.008356, 0.01135, 0.010173;
      |  0.005882, 0.007703, 0.006532, 0.005526;
      |  0.006739, 0.007058, 0.006772, 0.005603;
      |  0.008222, 0.004287, 0.009601, 0.005034;
      |  0.008985, 0.007821, 0.008932, 0.006662;
      |  0.004704, 0.003171, 0.002422, 0.004036] Ohm
      tau2_mat=|
      | [131.6948, 137.0217, 141.2851, 129.3807;
      |  146.2759, 158.6208, 157.255, 143.944;
      |  158.5443, 177.3225, 156.7434, 144.0735;
      |  144.8009, 123.279, 145.0945, 176.1753;
      |  158.7596, 137.3241, 203.2495, 189.2199;
      |  149.8847, 154.5014, 161.1061, 146.3519;
      |  135.3572, 173.7062, 166.0613, 159.34;
      |  123.823, 144.5727, 209.652, 117.4544;
      |  111.7616, 98.04929, 114.3433, 98.05822;
      |  125.3862, 75.97092, 110.7081, 120.3015] s
      settings: InternalSimscapePortConfiguration="{\"Bottom\":[],\"Left\":[{\"id\":\"p\",\"label\":\"+\",\"type\":\"foundation.electrical.electrical\"}],\"Right\":[{\"id\":\"n\",\"label\":\"-\",\"type\":\"foundation.electrical.electrical\"}],\"Top\":[]}"
      settings: LibrarySourceBlock=|
      | batt_lib/Cells/Battery
      | (Table-Based)
  Battery (Table-Based)33 : batteryecm_lib/Battery (Table-Based)  SOC_vec=[0.1, 0.188889, 0.277778, 0.366667, 0.455556, 0.544444, 0.633333, 0.722222, 0.811111, 0.9]  T_dependence=simscape.enum.tablebattery.temperature_dependence.yes  prm_dir=simscape.enum.tablebattery.prm_dir.noCurrentDirectionality  T_vec=[30, 32.5, 35, 38] degC  V0_mat=|  V0_vec=[3.5057, 3.566, 3.6337, 3.7127, 3.9259, 4.0777, 4.1928] V  V_range=[0, inf] V  R0_mat=|  R0_vec=[.0085, .0085, .0087, .0082, .0083, .0085, .0085] Ohm  R0_dis_mat=[.0117, .0085, .009; .011, .0085, .009; .0114, .0087, .0092; .0107, .0082, .0088; .0107, .0083, .0091; .0113, .0085, .0089; .0116, .0085, .0089] Ohm  R0_dis_vec=[.0085, .0085, .0087, .0082, .0083, .0085, .0085] Ohm  R0_ch_mat=[.0117, .0085, .009; .011, .0085, .009; .0114, .0087, .0092; .0107, .0082, .0088; .0107, .0083, .0091; .0113, .0085, .0089; .0116, .0085, .0089] Ohm  R0_ch_vec=[.0085, .0085, .0087, .0082, .0083, .0085, .0085] Ohm  AH=5 A*hr  prm_leak=simscape.enum.tablebattery.prm_leak.disabled  Rleak_vec=[8000, 7000, 6000] Ohm  Rleak=7e3 Ohm  extrapolation_option=simscape.enum.extrapolation.nearest  SOC_port=simscape.enum.tablebattery.enable.no  prm_dyn=simscape.enum.tablebattery.prm_dyn.rc2  R1_mat=|  R1_vec=[.0029, .0024, .0026, .0016, .0023, .0018, .0017] Ohm  tau1_mat=|  tau1_vec=[36, 45, 105, 29, 77, 33, 39] s  R2_mat=|  R2_vec=[.0029, .0024, .0026, .0016, .0023, .0018, .0017] Ohm  tau2_mat=|  tau2_vec=[36, 45, 105, 29, 77, 33, 39] s  R3_mat=[.0109, .0029, .0013; .0069, .0024, .0012; .0047, .0026, .0013; .0034, .0016, .001; .0033, .0023, .0014; .0033, .0018, .0011; .0028, .0017, .0011] Ohm  R3_vec=[.0029, .0024, .0026, .0016, .0023, .0018, .0017] Ohm  tau3_mat=[20, 36, 39; 31, 45, 39; 109, 105, 61; 36, 29, 26; 59, 77, 67; 40, 33, 29; 25, 39, 33] s  tau3_vec=[36, 45, 105, 29, 77, 33, 39] s  R4_mat=[.0109, .0029, .0013; .0069, .0024, .0012; .0047, .0026, .0013; .0034, .0016, .001; .0033, .0023, .0014; .0033, .0018, .0011; .0028, .0017, .0011] Ohm  R4_vec=[.0029, .0024, .0026, .0016, .0023, .0018, .0017] Ohm  tau4_mat=[20, 36, 39; 31, 45, 39; 109, 105, 61; 36, 29, 26; 59, 77, 67; 40, 33, 29; 25, 39, 33] s  tau4_vec=[36, 45, 105, 29, 77, 33, 39] s  R5_mat=[.0109, .0029, .0013; .0069, .0024, .0012; .0047, .0026, .0013; .0034, .0016, .001; .0033, .0023, .0014; .0033, .0018, .0011; .0028, .0017, .0011] Ohm  R5_vec=[.0029, .0024, .0026, .0016, .0023, .0018, .0017] Ohm  tau5_mat=[20, 36, 39; 31, 45, 39; 109, 105, 61; 36, 29, 26; 59, 77, 67; 40, 33, 29; 25, 39, 33] s  tau5_vec=[36, 45, 105, 29, 77, 33, 39] s  prm_fade=simscape.enum.tablebattery.prm_fade.disabled  N0=100  dV0=0  dR0=0  dAH=0  dRleak=0  dR1=0  dR2=0  dR3=0  dR4=0  dR5=0  N0vec=[0, 100, 200, 300]  Tfadevec=[298.15, 323.15] K  dV0vec=[0, 0, 0, 0]  dR0vec=[0, 0, 0, 0]  dAHvec=[0, 0, 0, 0]  dRleakvec=[0, 0, 0, 0]  dR1vec=[0, 0, 0, 0]  dR2vec=[0, 0, 0, 0]  dR3vec=[0, 0, 0, 0]  dR4vec=[0, 0, 0, 0]  dR5vec=[0, 0, 0, 0]  dV0mat=[0, 0; 0, 0; 0, 0; 0, 0]  dR0mat=[0, 0; 0, 0; 0, 0; 0, 0]  dAHmat=[0, 0; 0, 0; 0, 0; 0, 0]  dRleakmat=[0, 0; 0, 0; 0, 0; 0, 0]  dR1mat=[0, 0; 0, 0; 0, 0; 0, 0]  dR2mat=[0, 0; 0, 0; 0, 0; 0, 0]  dR3mat=[0, 0; 0, 0; 0, 0; 0, 0]  dR4mat=[0, 0; 0, 0; 0, 0; 0, 0]  dR5mat=[0, 0; 0, 0; 0, 0; 0, 0]  prm_age_modeling=simscape.enum.tablebattery.prm_age_modeling.equation  storage_dt_age_vec=[0] d  storage_T_age_vec=[273] K  prm_age_OCV=simscape.enum.tablebattery.prm_age_OCV.OCV  OCV_age=0.9  SOC_age=0.6  prm_age_resistance=simscape.enum.tablebattery.prm_age.disabled  OCV_scaling_age_resistance=2.2134e6  OCV_offset_age_resistance=1.632e6  temp_exp_age_resistance=0.515833569 V  t_exp_age_resistance=0.75  T_age_vec_resistance=[273.15, 298.15, 323.15] K  dt_age_vec_resistance=[0, 90, 180, 270] d  dR0_age_vec=[0, 0, 0]  t_meas_dR0_age=100 d  dR0_age_mat=[0, 0, 0; 0, 0, 0; 0, 0, 0; 0, 0, 0]  prm_age_capacity=simscape.enum.tablebattery.prm_age.disabled  OCV_scaling_age_capacity=1.5097e07  OCV_offset_age_capacity=8.3625e06  temp_exp_age_capacity=0.6011 V  t_exp_age_capacity=0.75  T_age_vec_capacity=[273.15, 298.15, 323.15] K  dt_age_vec_capacity=[0, 90, 180, 270] d  dAH_age_vec=[0, 0, 0]  t_meas_dAH_age=100 d  dAH_age_mat=[0, 0, 0; 0, 0, 0; 0, 0, 0; 0, 0, 0]  thermal_port=simscape.enum.thermaleffects.omit  temperature=298.15 K  thermal_mass=100 J/K  i_specify=off  i_priority=None  i=0 A  i_nominal_specify=off  i_nominal_value=1  i_nominal_unit=A  v_specify=off  v_priority=None  v=0 V  v_nominal_specify=off  v_nominal_value=1  v_nominal_unit=V  stateOfCharge_specify=on  stateOfCharge_priority=High  stateOfCharge=1  stateOfCharge_nominal_specify=off  stateOfCharge_nominal_value=1  stateOfCharge_nominal_unit=1  num_cycles_specify=off  num_cycles_priority=High  num_cycles=0  num_cycles_nominal_specify=off  num_cycles_nominal_value=1  num_cycles_nominal_unit=1  cell_temperature_specify=off  cell_temperature_priority=High  cell_temperature=298.15 K  cell_temperature_nominal_specify=off  cell_temperature_nominal_value=1  cell_temperature_nominal_unit=K
      V0_mat=|
      | [3.0263, 3.218033, 3.364889, 3.493933, 3.610678, 3.733744, 3.85405, 3.950717, 4.040478, 4.0819;
      |  3.0376, 3.2248, 3.370311, 3.498533, 3.615311, 3.736956, 3.845633, 3.929256, 4.040056, 4.0821;
      |  3.0439, 3.227633, 3.3731, 3.5007, 3.616611, 3.737589, 3.8457, 3.9287, 4.039133, 4.0826;
      |  3.0283, 3.217989, 3.364589, 3.493767, 3.609467, 3.731156, 3.8417, 3.925833, 4.036322, 4.0821]' V
      R0_mat=|
      | [0.011867, 0.008993, 0.007674, 0.006911, 0.006648, 0.006648, 0.006528, 0.006157, 0.005996, 0.0073;
      |  0.0109, 0.006456, 0.005381, 0.005078, 0.005, 0.005044, 0.005511, 0.006407, 0.006522, 0.005367;
      |  0.0102, 0.007978, 0.006793, 0.0062, 0.006033, 0.005441, 0.0051, 0.005707, 0.005037, 0.005067;
      |  0.0101, 0.007759, 0.006637, 0.006022, 0.005741, 0.005667, 0.005311, 0.004911, 0.005859, 0.004733]' Ohm
      R1_mat=|
      | [0.007451, 0.008294, 0.007745, 0.007391;
      |  0.003783, 0.00363, 0.004415, 0.004051;
      |  0.002841, 0.00298, 0.003698, 0.003391;
      |  0.003185, 0.002661, 0.003493, 0.00379;
      |  0.00379, 0.003147, 0.004204, 0.004229;
      |  0.004015, 0.003677, 0.004233, 0.004481;
      |  0.003791, 0.004051, 0.003886, 0.004189;
      |  0.003416, 0.004883, 0.004387, 0.003743;
      |  0.00328, 0.005238, 0.003472, 0.004883;
      |  0.004816, 0.004218, 0.003847, 0.003891] Ohm
      tau1_mat=|
      | [8.156247, 6.866126, 6.747335, 6.573366;
      |  6.436096, 6.88158, 6.206576, 5.30011;
      |  7.074429, 7.267109, 6.564215, 5.759928;
      |  8.61232, 7.062398, 6.553799, 7.485573;
      |  10.88135, 8.569373, 8.681328, 8.99043;
      |  11.88702, 10.35435, 10.74073, 9.985533;
      |  11.15433, 10.61987, 10.52072, 10.95124;
      |  10.33388, 9.573709, 9.987626, 10.94588;
      |  9.883806, 9.219359, 8.513241, 9.109378;
      |  11.2706, 10.03414, 9.643065, 10.06297] s
      R2_mat=|
      | [0.040653, 0.04799, 0.046915, 0.044404;
      |  0.026828, 0.033189, 0.032279, 0.030363;
      |  0.019744, 0.025225, 0.021211, 0.019613;
      |  0.012414, 0.014827, 0.017004, 0.016763;
      |  0.007363, 0.008356, 0.01135, 0.010173;
      |  0.005882, 0.007703, 0.006532, 0.005526;
      |  0.006739, 0.007058, 0.006772, 0.005603;
      |  0.008222, 0.004287, 0.009601, 0.005034;
      |  0.008985, 0.007821, 0.008932, 0.006662;
      |  0.004704, 0.003171, 0.002422, 0.004036] Ohm
      tau2_mat=|
      | [131.6948, 137.0217, 141.2851, 129.3807;
      |  146.2759, 158.6208, 157.255, 143.944;
      |  158.5443, 177.3225, 156.7434, 144.0735;
      |  144.8009, 123.279, 145.0945, 176.1753;
      |  158.7596, 137.3241, 203.2495, 189.2199;
      |  149.8847, 154.5014, 161.1061, 146.3519;
      |  135.3572, 173.7062, 166.0613, 159.34;
      |  123.823, 144.5727, 209.652, 117.4544;
      |  111.7616, 98.04929, 114.3433, 98.05822;
      |  125.3862, 75.97092, 110.7081, 120.3015] s
      settings: InternalSimscapePortConfiguration="{\"Bottom\":[],\"Left\":[{\"id\":\"p\",\"label\":\"+\",\"type\":\"foundation.electrical.electrical\"}],\"Right\":[{\"id\":\"n\",\"label\":\"-\",\"type\":\"foundation.electrical.electrical\"}],\"Top\":[]}"
      settings: LibrarySourceBlock=|
      | batt_lib/Cells/Battery
      | (Table-Based)
  Battery (Table-Based)34 : batteryecm_lib/Battery (Table-Based)  SOC_vec=[0.1, 0.188889, 0.277778, 0.366667, 0.455556, 0.544444, 0.633333, 0.722222, 0.811111, 0.9]  T_dependence=simscape.enum.tablebattery.temperature_dependence.yes  prm_dir=simscape.enum.tablebattery.prm_dir.noCurrentDirectionality  T_vec=[30, 32.5, 35, 38] degC  V0_mat=|  V0_vec=[3.5057, 3.566, 3.6337, 3.7127, 3.9259, 4.0777, 4.1928] V  V_range=[0, inf] V  R0_mat=|  R0_vec=[.0085, .0085, .0087, .0082, .0083, .0085, .0085] Ohm  R0_dis_mat=[.0117, .0085, .009; .011, .0085, .009; .0114, .0087, .0092; .0107, .0082, .0088; .0107, .0083, .0091; .0113, .0085, .0089; .0116, .0085, .0089] Ohm  R0_dis_vec=[.0085, .0085, .0087, .0082, .0083, .0085, .0085] Ohm  R0_ch_mat=[.0117, .0085, .009; .011, .0085, .009; .0114, .0087, .0092; .0107, .0082, .0088; .0107, .0083, .0091; .0113, .0085, .0089; .0116, .0085, .0089] Ohm  R0_ch_vec=[.0085, .0085, .0087, .0082, .0083, .0085, .0085] Ohm  AH=5 A*hr  prm_leak=simscape.enum.tablebattery.prm_leak.disabled  Rleak_vec=[8000, 7000, 6000] Ohm  Rleak=7e3 Ohm  extrapolation_option=simscape.enum.extrapolation.nearest  SOC_port=simscape.enum.tablebattery.enable.no  prm_dyn=simscape.enum.tablebattery.prm_dyn.rc2  R1_mat=|  R1_vec=[.0029, .0024, .0026, .0016, .0023, .0018, .0017] Ohm  tau1_mat=|  tau1_vec=[36, 45, 105, 29, 77, 33, 39] s  R2_mat=|  R2_vec=[.0029, .0024, .0026, .0016, .0023, .0018, .0017] Ohm  tau2_mat=|  tau2_vec=[36, 45, 105, 29, 77, 33, 39] s  R3_mat=[.0109, .0029, .0013; .0069, .0024, .0012; .0047, .0026, .0013; .0034, .0016, .001; .0033, .0023, .0014; .0033, .0018, .0011; .0028, .0017, .0011] Ohm  R3_vec=[.0029, .0024, .0026, .0016, .0023, .0018, .0017] Ohm  tau3_mat=[20, 36, 39; 31, 45, 39; 109, 105, 61; 36, 29, 26; 59, 77, 67; 40, 33, 29; 25, 39, 33] s  tau3_vec=[36, 45, 105, 29, 77, 33, 39] s  R4_mat=[.0109, .0029, .0013; .0069, .0024, .0012; .0047, .0026, .0013; .0034, .0016, .001; .0033, .0023, .0014; .0033, .0018, .0011; .0028, .0017, .0011] Ohm  R4_vec=[.0029, .0024, .0026, .0016, .0023, .0018, .0017] Ohm  tau4_mat=[20, 36, 39; 31, 45, 39; 109, 105, 61; 36, 29, 26; 59, 77, 67; 40, 33, 29; 25, 39, 33] s  tau4_vec=[36, 45, 105, 29, 77, 33, 39] s  R5_mat=[.0109, .0029, .0013; .0069, .0024, .0012; .0047, .0026, .0013; .0034, .0016, .001; .0033, .0023, .0014; .0033, .0018, .0011; .0028, .0017, .0011] Ohm  R5_vec=[.0029, .0024, .0026, .0016, .0023, .0018, .0017] Ohm  tau5_mat=[20, 36, 39; 31, 45, 39; 109, 105, 61; 36, 29, 26; 59, 77, 67; 40, 33, 29; 25, 39, 33] s  tau5_vec=[36, 45, 105, 29, 77, 33, 39] s  prm_fade=simscape.enum.tablebattery.prm_fade.disabled  N0=100  dV0=0  dR0=0  dAH=0  dRleak=0  dR1=0  dR2=0  dR3=0  dR4=0  dR5=0  N0vec=[0, 100, 200, 300]  Tfadevec=[298.15, 323.15] K  dV0vec=[0, 0, 0, 0]  dR0vec=[0, 0, 0, 0]  dAHvec=[0, 0, 0, 0]  dRleakvec=[0, 0, 0, 0]  dR1vec=[0, 0, 0, 0]  dR2vec=[0, 0, 0, 0]  dR3vec=[0, 0, 0, 0]  dR4vec=[0, 0, 0, 0]  dR5vec=[0, 0, 0, 0]  dV0mat=[0, 0; 0, 0; 0, 0; 0, 0]  dR0mat=[0, 0; 0, 0; 0, 0; 0, 0]  dAHmat=[0, 0; 0, 0; 0, 0; 0, 0]  dRleakmat=[0, 0; 0, 0; 0, 0; 0, 0]  dR1mat=[0, 0; 0, 0; 0, 0; 0, 0]  dR2mat=[0, 0; 0, 0; 0, 0; 0, 0]  dR3mat=[0, 0; 0, 0; 0, 0; 0, 0]  dR4mat=[0, 0; 0, 0; 0, 0; 0, 0]  dR5mat=[0, 0; 0, 0; 0, 0; 0, 0]  prm_age_modeling=simscape.enum.tablebattery.prm_age_modeling.equation  storage_dt_age_vec=[0] d  storage_T_age_vec=[273] K  prm_age_OCV=simscape.enum.tablebattery.prm_age_OCV.OCV  OCV_age=0.9  SOC_age=0.6  prm_age_resistance=simscape.enum.tablebattery.prm_age.disabled  OCV_scaling_age_resistance=2.2134e6  OCV_offset_age_resistance=1.632e6  temp_exp_age_resistance=0.515833569 V  t_exp_age_resistance=0.75  T_age_vec_resistance=[273.15, 298.15, 323.15] K  dt_age_vec_resistance=[0, 90, 180, 270] d  dR0_age_vec=[0, 0, 0]  t_meas_dR0_age=100 d  dR0_age_mat=[0, 0, 0; 0, 0, 0; 0, 0, 0; 0, 0, 0]  prm_age_capacity=simscape.enum.tablebattery.prm_age.disabled  OCV_scaling_age_capacity=1.5097e07  OCV_offset_age_capacity=8.3625e06  temp_exp_age_capacity=0.6011 V  t_exp_age_capacity=0.75  T_age_vec_capacity=[273.15, 298.15, 323.15] K  dt_age_vec_capacity=[0, 90, 180, 270] d  dAH_age_vec=[0, 0, 0]  t_meas_dAH_age=100 d  dAH_age_mat=[0, 0, 0; 0, 0, 0; 0, 0, 0; 0, 0, 0]  thermal_port=simscape.enum.thermaleffects.omit  temperature=298.15 K  thermal_mass=100 J/K  i_specify=off  i_priority=None  i=0 A  i_nominal_specify=off  i_nominal_value=1  i_nominal_unit=A  v_specify=off  v_priority=None  v=0 V  v_nominal_specify=off  v_nominal_value=1  v_nominal_unit=V  stateOfCharge_specify=on  stateOfCharge_priority=High  stateOfCharge=1  stateOfCharge_nominal_specify=off  stateOfCharge_nominal_value=1  stateOfCharge_nominal_unit=1  num_cycles_specify=off  num_cycles_priority=High  num_cycles=0  num_cycles_nominal_specify=off  num_cycles_nominal_value=1  num_cycles_nominal_unit=1  cell_temperature_specify=off  cell_temperature_priority=High  cell_temperature=298.15 K  cell_temperature_nominal_specify=off  cell_temperature_nominal_value=1  cell_temperature_nominal_unit=K
      V0_mat=|
      | [3.0263, 3.218033, 3.364889, 3.493933, 3.610678, 3.733744, 3.85405, 3.950717, 4.040478, 4.0819;
      |  3.0376, 3.2248, 3.370311, 3.498533, 3.615311, 3.736956, 3.845633, 3.929256, 4.040056, 4.0821;
      |  3.0439, 3.227633, 3.3731, 3.5007, 3.616611, 3.737589, 3.8457, 3.9287, 4.039133, 4.0826;
      |  3.0283, 3.217989, 3.364589, 3.493767, 3.609467, 3.731156, 3.8417, 3.925833, 4.036322, 4.0821]' V
      R0_mat=|
      | [0.011867, 0.008993, 0.007674, 0.006911, 0.006648, 0.006648, 0.006528, 0.006157, 0.005996, 0.0073;
      |  0.0109, 0.006456, 0.005381, 0.005078, 0.005, 0.005044, 0.005511, 0.006407, 0.006522, 0.005367;
      |  0.0102, 0.007978, 0.006793, 0.0062, 0.006033, 0.005441, 0.0051, 0.005707, 0.005037, 0.005067;
      |  0.0101, 0.007759, 0.006637, 0.006022, 0.005741, 0.005667, 0.005311, 0.004911, 0.005859, 0.004733]' Ohm
      R1_mat=|
      | [0.007451, 0.008294, 0.007745, 0.007391;
      |  0.003783, 0.00363, 0.004415, 0.004051;
      |  0.002841, 0.00298, 0.003698, 0.003391;
      |  0.003185, 0.002661, 0.003493, 0.00379;
      |  0.00379, 0.003147, 0.004204, 0.004229;
      |  0.004015, 0.003677, 0.004233, 0.004481;
      |  0.003791, 0.004051, 0.003886, 0.004189;
      |  0.003416, 0.004883, 0.004387, 0.003743;
      |  0.00328, 0.005238, 0.003472, 0.004883;
      |  0.004816, 0.004218, 0.003847, 0.003891] Ohm
      tau1_mat=|
      | [8.156247, 6.866126, 6.747335, 6.573366;
      |  6.436096, 6.88158, 6.206576, 5.30011;
      |  7.074429, 7.267109, 6.564215, 5.759928;
      |  8.61232, 7.062398, 6.553799, 7.485573;
      |  10.88135, 8.569373, 8.681328, 8.99043;
      |  11.88702, 10.35435, 10.74073, 9.985533;
      |  11.15433, 10.61987, 10.52072, 10.95124;
      |  10.33388, 9.573709, 9.987626, 10.94588;
      |  9.883806, 9.219359, 8.513241, 9.109378;
      |  11.2706, 10.03414, 9.643065, 10.06297] s
      R2_mat=|
      | [0.040653, 0.04799, 0.046915, 0.044404;
      |  0.026828, 0.033189, 0.032279, 0.030363;
      |  0.019744, 0.025225, 0.021211, 0.019613;
      |  0.012414, 0.014827, 0.017004, 0.016763;
      |  0.007363, 0.008356, 0.01135, 0.010173;
      |  0.005882, 0.007703, 0.006532, 0.005526;
      |  0.006739, 0.007058, 0.006772, 0.005603;
      |  0.008222, 0.004287, 0.009601, 0.005034;
      |  0.008985, 0.007821, 0.008932, 0.006662;
      |  0.004704, 0.003171, 0.002422, 0.004036] Ohm
      tau2_mat=|
      | [131.6948, 137.0217, 141.2851, 129.3807;
      |  146.2759, 158.6208, 157.255, 143.944;
      |  158.5443, 177.3225, 156.7434, 144.0735;
      |  144.8009, 123.279, 145.0945, 176.1753;
      |  158.7596, 137.3241, 203.2495, 189.2199;
      |  149.8847, 154.5014, 161.1061, 146.3519;
      |  135.3572, 173.7062, 166.0613, 159.34;
      |  123.823, 144.5727, 209.652, 117.4544;
      |  111.7616, 98.04929, 114.3433, 98.05822;
      |  125.3862, 75.97092, 110.7081, 120.3015] s
      settings: InternalSimscapePortConfiguration="{\"Bottom\":[],\"Left\":[{\"id\":\"p\",\"label\":\"+\",\"type\":\"foundation.electrical.electrical\"}],\"Right\":[{\"id\":\"n\",\"label\":\"-\",\"type\":\"foundation.electrical.electrical\"}],\"Top\":[]}"
      settings: LibrarySourceBlock=|
      | batt_lib/Cells/Battery
      | (Table-Based)
  Battery (Table-Based)35 : batteryecm_lib/Battery (Table-Based)  SOC_vec=[0.1, 0.188889, 0.277778, 0.366667, 0.455556, 0.544444, 0.633333, 0.722222, 0.811111, 0.9]  T_dependence=simscape.enum.tablebattery.temperature_dependence.yes  prm_dir=simscape.enum.tablebattery.prm_dir.noCurrentDirectionality  T_vec=[30, 32.5, 35, 38] degC  V0_mat=|  V0_vec=[3.5057, 3.566, 3.6337, 3.7127, 3.9259, 4.0777, 4.1928] V  V_range=[0, inf] V  R0_mat=|  R0_vec=[.0085, .0085, .0087, .0082, .0083, .0085, .0085] Ohm  R0_dis_mat=[.0117, .0085, .009; .011, .0085, .009; .0114, .0087, .0092; .0107, .0082, .0088; .0107, .0083, .0091; .0113, .0085, .0089; .0116, .0085, .0089] Ohm  R0_dis_vec=[.0085, .0085, .0087, .0082, .0083, .0085, .0085] Ohm  R0_ch_mat=[.0117, .0085, .009; .011, .0085, .009; .0114, .0087, .0092; .0107, .0082, .0088; .0107, .0083, .0091; .0113, .0085, .0089; .0116, .0085, .0089] Ohm  R0_ch_vec=[.0085, .0085, .0087, .0082, .0083, .0085, .0085] Ohm  AH=5 A*hr  prm_leak=simscape.enum.tablebattery.prm_leak.disabled  Rleak_vec=[8000, 7000, 6000] Ohm  Rleak=7e3 Ohm  extrapolation_option=simscape.enum.extrapolation.nearest  SOC_port=simscape.enum.tablebattery.enable.no  prm_dyn=simscape.enum.tablebattery.prm_dyn.rc2  R1_mat=|  R1_vec=[.0029, .0024, .0026, .0016, .0023, .0018, .0017] Ohm  tau1_mat=|  tau1_vec=[36, 45, 105, 29, 77, 33, 39] s  R2_mat=|  R2_vec=[.0029, .0024, .0026, .0016, .0023, .0018, .0017] Ohm  tau2_mat=|  tau2_vec=[36, 45, 105, 29, 77, 33, 39] s  R3_mat=[.0109, .0029, .0013; .0069, .0024, .0012; .0047, .0026, .0013; .0034, .0016, .001; .0033, .0023, .0014; .0033, .0018, .0011; .0028, .0017, .0011] Ohm  R3_vec=[.0029, .0024, .0026, .0016, .0023, .0018, .0017] Ohm  tau3_mat=[20, 36, 39; 31, 45, 39; 109, 105, 61; 36, 29, 26; 59, 77, 67; 40, 33, 29; 25, 39, 33] s  tau3_vec=[36, 45, 105, 29, 77, 33, 39] s  R4_mat=[.0109, .0029, .0013; .0069, .0024, .0012; .0047, .0026, .0013; .0034, .0016, .001; .0033, .0023, .0014; .0033, .0018, .0011; .0028, .0017, .0011] Ohm  R4_vec=[.0029, .0024, .0026, .0016, .0023, .0018, .0017] Ohm  tau4_mat=[20, 36, 39; 31, 45, 39; 109, 105, 61; 36, 29, 26; 59, 77, 67; 40, 33, 29; 25, 39, 33] s  tau4_vec=[36, 45, 105, 29, 77, 33, 39] s  R5_mat=[.0109, .0029, .0013; .0069, .0024, .0012; .0047, .0026, .0013; .0034, .0016, .001; .0033, .0023, .0014; .0033, .0018, .0011; .0028, .0017, .0011] Ohm  R5_vec=[.0029, .0024, .0026, .0016, .0023, .0018, .0017] Ohm  tau5_mat=[20, 36, 39; 31, 45, 39; 109, 105, 61; 36, 29, 26; 59, 77, 67; 40, 33, 29; 25, 39, 33] s  tau5_vec=[36, 45, 105, 29, 77, 33, 39] s  prm_fade=simscape.enum.tablebattery.prm_fade.disabled  N0=100  dV0=0  dR0=0  dAH=0  dRleak=0  dR1=0  dR2=0  dR3=0  dR4=0  dR5=0  N0vec=[0, 100, 200, 300]  Tfadevec=[298.15, 323.15] K  dV0vec=[0, 0, 0, 0]  dR0vec=[0, 0, 0, 0]  dAHvec=[0, 0, 0, 0]  dRleakvec=[0, 0, 0, 0]  dR1vec=[0, 0, 0, 0]  dR2vec=[0, 0, 0, 0]  dR3vec=[0, 0, 0, 0]  dR4vec=[0, 0, 0, 0]  dR5vec=[0, 0, 0, 0]  dV0mat=[0, 0; 0, 0; 0, 0; 0, 0]  dR0mat=[0, 0; 0, 0; 0, 0; 0, 0]  dAHmat=[0, 0; 0, 0; 0, 0; 0, 0]  dRleakmat=[0, 0; 0, 0; 0, 0; 0, 0]  dR1mat=[0, 0; 0, 0; 0, 0; 0, 0]  dR2mat=[0, 0; 0, 0; 0, 0; 0, 0]  dR3mat=[0, 0; 0, 0; 0, 0; 0, 0]  dR4mat=[0, 0; 0, 0; 0, 0; 0, 0]  dR5mat=[0, 0; 0, 0; 0, 0; 0, 0]  prm_age_modeling=simscape.enum.tablebattery.prm_age_modeling.equation  storage_dt_age_vec=[0] d  storage_T_age_vec=[273] K  prm_age_OCV=simscape.enum.tablebattery.prm_age_OCV.OCV  OCV_age=0.9  SOC_age=0.6  prm_age_resistance=simscape.enum.tablebattery.prm_age.disabled  OCV_scaling_age_resistance=2.2134e6  OCV_offset_age_resistance=1.632e6  temp_exp_age_resistance=0.515833569 V  t_exp_age_resistance=0.75  T_age_vec_resistance=[273.15, 298.15, 323.15] K  dt_age_vec_resistance=[0, 90, 180, 270] d  dR0_age_vec=[0, 0, 0]  t_meas_dR0_age=100 d  dR0_age_mat=[0, 0, 0; 0, 0, 0; 0, 0, 0; 0, 0, 0]  prm_age_capacity=simscape.enum.tablebattery.prm_age.disabled  OCV_scaling_age_capacity=1.5097e07  OCV_offset_age_capacity=8.3625e06  temp_exp_age_capacity=0.6011 V  t_exp_age_capacity=0.75  T_age_vec_capacity=[273.15, 298.15, 323.15] K  dt_age_vec_capacity=[0, 90, 180, 270] d  dAH_age_vec=[0, 0, 0]  t_meas_dAH_age=100 d  dAH_age_mat=[0, 0, 0; 0, 0, 0; 0, 0, 0; 0, 0, 0]  thermal_port=simscape.enum.thermaleffects.omit  temperature=298.15 K  thermal_mass=100 J/K  i_specify=off  i_priority=None  i=0 A  i_nominal_specify=off  i_nominal_value=1  i_nominal_unit=A  v_specify=off  v_priority=None  v=0 V  v_nominal_specify=off  v_nominal_value=1  v_nominal_unit=V  stateOfCharge_specify=on  stateOfCharge_priority=High  stateOfCharge=1  stateOfCharge_nominal_specify=off  stateOfCharge_nominal_value=1  stateOfCharge_nominal_unit=1  num_cycles_specify=off  num_cycles_priority=High  num_cycles=0  num_cycles_nominal_specify=off  num_cycles_nominal_value=1  num_cycles_nominal_unit=1  cell_temperature_specify=off  cell_temperature_priority=High  cell_temperature=298.15 K  cell_temperature_nominal_specify=off  cell_temperature_nominal_value=1  cell_temperature_nominal_unit=K
      V0_mat=|
      | [3.0263, 3.218033, 3.364889, 3.493933, 3.610678, 3.733744, 3.85405, 3.950717, 4.040478, 4.0819;
      |  3.0376, 3.2248, 3.370311, 3.498533, 3.615311, 3.736956, 3.845633, 3.929256, 4.040056, 4.0821;
      |  3.0439, 3.227633, 3.3731, 3.5007, 3.616611, 3.737589, 3.8457, 3.9287, 4.039133, 4.0826;
      |  3.0283, 3.217989, 3.364589, 3.493767, 3.609467, 3.731156, 3.8417, 3.925833, 4.036322, 4.0821]' V
      R0_mat=|
      | [0.011867, 0.008993, 0.007674, 0.006911, 0.006648, 0.006648, 0.006528, 0.006157, 0.005996, 0.0073;
      |  0.0109, 0.006456, 0.005381, 0.005078, 0.005, 0.005044, 0.005511, 0.006407, 0.006522, 0.005367;
      |  0.0102, 0.007978, 0.006793, 0.0062, 0.006033, 0.005441, 0.0051, 0.005707, 0.005037, 0.005067;
      |  0.0101, 0.007759, 0.006637, 0.006022, 0.005741, 0.005667, 0.005311, 0.004911, 0.005859, 0.004733]' Ohm
      R1_mat=|
      | [0.007451, 0.008294, 0.007745, 0.007391;
      |  0.003783, 0.00363, 0.004415, 0.004051;
      |  0.002841, 0.00298, 0.003698, 0.003391;
      |  0.003185, 0.002661, 0.003493, 0.00379;
      |  0.00379, 0.003147, 0.004204, 0.004229;
      |  0.004015, 0.003677, 0.004233, 0.004481;
      |  0.003791, 0.004051, 0.003886, 0.004189;
      |  0.003416, 0.004883, 0.004387, 0.003743;
      |  0.00328, 0.005238, 0.003472, 0.004883;
      |  0.004816, 0.004218, 0.003847, 0.003891] Ohm
      tau1_mat=|
      | [8.156247, 6.866126, 6.747335, 6.573366;
      |  6.436096, 6.88158, 6.206576, 5.30011;
      |  7.074429, 7.267109, 6.564215, 5.759928;
      |  8.61232, 7.062398, 6.553799, 7.485573;
      |  10.88135, 8.569373, 8.681328, 8.99043;
      |  11.88702, 10.35435, 10.74073, 9.985533;
      |  11.15433, 10.61987, 10.52072, 10.95124;
      |  10.33388, 9.573709, 9.987626, 10.94588;
      |  9.883806, 9.219359, 8.513241, 9.109378;
      |  11.2706, 10.03414, 9.643065, 10.06297] s
      R2_mat=|
      | [0.040653, 0.04799, 0.046915, 0.044404;
      |  0.026828, 0.033189, 0.032279, 0.030363;
      |  0.019744, 0.025225, 0.021211, 0.019613;
      |  0.012414, 0.014827, 0.017004, 0.016763;
      |  0.007363, 0.008356, 0.01135, 0.010173;
      |  0.005882, 0.007703, 0.006532, 0.005526;
      |  0.006739, 0.007058, 0.006772, 0.005603;
      |  0.008222, 0.004287, 0.009601, 0.005034;
      |  0.008985, 0.007821, 0.008932, 0.006662;
      |  0.004704, 0.003171, 0.002422, 0.004036] Ohm
      tau2_mat=|
      | [131.6948, 137.0217, 141.2851, 129.3807;
      |  146.2759, 158.6208, 157.255, 143.944;
      |  158.5443, 177.3225, 156.7434, 144.0735;
      |  144.8009, 123.279, 145.0945, 176.1753;
      |  158.7596, 137.3241, 203.2495, 189.2199;
      |  149.8847, 154.5014, 161.1061, 146.3519;
      |  135.3572, 173.7062, 166.0613, 159.34;
      |  123.823, 144.5727, 209.652, 117.4544;
      |  111.7616, 98.04929, 114.3433, 98.05822;
      |  125.3862, 75.97092, 110.7081, 120.3015] s
      settings: InternalSimscapePortConfiguration="{\"Bottom\":[],\"Left\":[{\"id\":\"p\",\"label\":\"+\",\"type\":\"foundation.electrical.electrical\"}],\"Right\":[{\"id\":\"n\",\"label\":\"-\",\"type\":\"foundation.electrical.electrical\"}],\"Top\":[]}"
      settings: LibrarySourceBlock=|
      | batt_lib/Cells/Battery
      | (Table-Based)
  Battery (Table-Based)36 : batteryecm_lib/Battery (Table-Based)  SOC_vec=[0.1, 0.188889, 0.277778, 0.366667, 0.455556, 0.544444, 0.633333, 0.722222, 0.811111, 0.9]  T_dependence=simscape.enum.tablebattery.temperature_dependence.yes  prm_dir=simscape.enum.tablebattery.prm_dir.noCurrentDirectionality  T_vec=[30, 32.5, 35, 38] degC  V0_mat=|  V0_vec=[3.5057, 3.566, 3.6337, 3.7127, 3.9259, 4.0777, 4.1928] V  V_range=[0, inf] V  R0_mat=|  R0_vec=[.0085, .0085, .0087, .0082, .0083, .0085, .0085] Ohm  R0_dis_mat=[.0117, .0085, .009; .011, .0085, .009; .0114, .0087, .0092; .0107, .0082, .0088; .0107, .0083, .0091; .0113, .0085, .0089; .0116, .0085, .0089] Ohm  R0_dis_vec=[.0085, .0085, .0087, .0082, .0083, .0085, .0085] Ohm  R0_ch_mat=[.0117, .0085, .009; .011, .0085, .009; .0114, .0087, .0092; .0107, .0082, .0088; .0107, .0083, .0091; .0113, .0085, .0089; .0116, .0085, .0089] Ohm  R0_ch_vec=[.0085, .0085, .0087, .0082, .0083, .0085, .0085] Ohm  AH=5 A*hr  prm_leak=simscape.enum.tablebattery.prm_leak.disabled  Rleak_vec=[8000, 7000, 6000] Ohm  Rleak=7e3 Ohm  extrapolation_option=simscape.enum.extrapolation.nearest  SOC_port=simscape.enum.tablebattery.enable.no  prm_dyn=simscape.enum.tablebattery.prm_dyn.rc2  R1_mat=|  R1_vec=[.0029, .0024, .0026, .0016, .0023, .0018, .0017] Ohm  tau1_mat=|  tau1_vec=[36, 45, 105, 29, 77, 33, 39] s  R2_mat=|  R2_vec=[.0029, .0024, .0026, .0016, .0023, .0018, .0017] Ohm  tau2_mat=|  tau2_vec=[36, 45, 105, 29, 77, 33, 39] s  R3_mat=[.0109, .0029, .0013; .0069, .0024, .0012; .0047, .0026, .0013; .0034, .0016, .001; .0033, .0023, .0014; .0033, .0018, .0011; .0028, .0017, .0011] Ohm  R3_vec=[.0029, .0024, .0026, .0016, .0023, .0018, .0017] Ohm  tau3_mat=[20, 36, 39; 31, 45, 39; 109, 105, 61; 36, 29, 26; 59, 77, 67; 40, 33, 29; 25, 39, 33] s  tau3_vec=[36, 45, 105, 29, 77, 33, 39] s  R4_mat=[.0109, .0029, .0013; .0069, .0024, .0012; .0047, .0026, .0013; .0034, .0016, .001; .0033, .0023, .0014; .0033, .0018, .0011; .0028, .0017, .0011] Ohm  R4_vec=[.0029, .0024, .0026, .0016, .0023, .0018, .0017] Ohm  tau4_mat=[20, 36, 39; 31, 45, 39; 109, 105, 61; 36, 29, 26; 59, 77, 67; 40, 33, 29; 25, 39, 33] s  tau4_vec=[36, 45, 105, 29, 77, 33, 39] s  R5_mat=[.0109, .0029, .0013; .0069, .0024, .0012; .0047, .0026, .0013; .0034, .0016, .001; .0033, .0023, .0014; .0033, .0018, .0011; .0028, .0017, .0011] Ohm  R5_vec=[.0029, .0024, .0026, .0016, .0023, .0018, .0017] Ohm  tau5_mat=[20, 36, 39; 31, 45, 39; 109, 105, 61; 36, 29, 26; 59, 77, 67; 40, 33, 29; 25, 39, 33] s  tau5_vec=[36, 45, 105, 29, 77, 33, 39] s  prm_fade=simscape.enum.tablebattery.prm_fade.disabled  N0=100  dV0=0  dR0=0  dAH=0  dRleak=0  dR1=0  dR2=0  dR3=0  dR4=0  dR5=0  N0vec=[0, 100, 200, 300]  Tfadevec=[298.15, 323.15] K  dV0vec=[0, 0, 0, 0]  dR0vec=[0, 0, 0, 0]  dAHvec=[0, 0, 0, 0]  dRleakvec=[0, 0, 0, 0]  dR1vec=[0, 0, 0, 0]  dR2vec=[0, 0, 0, 0]  dR3vec=[0, 0, 0, 0]  dR4vec=[0, 0, 0, 0]  dR5vec=[0, 0, 0, 0]  dV0mat=[0, 0; 0, 0; 0, 0; 0, 0]  dR0mat=[0, 0; 0, 0; 0, 0; 0, 0]  dAHmat=[0, 0; 0, 0; 0, 0; 0, 0]  dRleakmat=[0, 0; 0, 0; 0, 0; 0, 0]  dR1mat=[0, 0; 0, 0; 0, 0; 0, 0]  dR2mat=[0, 0; 0, 0; 0, 0; 0, 0]  dR3mat=[0, 0; 0, 0; 0, 0; 0, 0]  dR4mat=[0, 0; 0, 0; 0, 0; 0, 0]  dR5mat=[0, 0; 0, 0; 0, 0; 0, 0]  prm_age_modeling=simscape.enum.tablebattery.prm_age_modeling.equation  storage_dt_age_vec=[0] d  storage_T_age_vec=[273] K  prm_age_OCV=simscape.enum.tablebattery.prm_age_OCV.OCV  OCV_age=0.9  SOC_age=0.6  prm_age_resistance=simscape.enum.tablebattery.prm_age.disabled  OCV_scaling_age_resistance=2.2134e6  OCV_offset_age_resistance=1.632e6  temp_exp_age_resistance=0.515833569 V  t_exp_age_resistance=0.75  T_age_vec_resistance=[273.15, 298.15, 323.15] K  dt_age_vec_resistance=[0, 90, 180, 270] d  dR0_age_vec=[0, 0, 0]  t_meas_dR0_age=100 d  dR0_age_mat=[0, 0, 0; 0, 0, 0; 0, 0, 0; 0, 0, 0]  prm_age_capacity=simscape.enum.tablebattery.prm_age.disabled  OCV_scaling_age_capacity=1.5097e07  OCV_offset_age_capacity=8.3625e06  temp_exp_age_capacity=0.6011 V  t_exp_age_capacity=0.75  T_age_vec_capacity=[273.15, 298.15, 323.15] K  dt_age_vec_capacity=[0, 90, 180, 270] d  dAH_age_vec=[0, 0, 0]  t_meas_dAH_age=100 d  dAH_age_mat=[0, 0, 0; 0, 0, 0; 0, 0, 0; 0, 0, 0]  thermal_port=simscape.enum.thermaleffects.omit  temperature=298.15 K  thermal_mass=100 J/K  i_specify=off  i_priority=None  i=0 A  i_nominal_specify=off  i_nominal_value=1  i_nominal_unit=A  v_specify=off  v_priority=None  v=0 V  v_nominal_specify=off  v_nominal_value=1  v_nominal_unit=V  stateOfCharge_specify=on  stateOfCharge_priority=High  stateOfCharge=1  stateOfCharge_nominal_specify=off  stateOfCharge_nominal_value=1  stateOfCharge_nominal_unit=1  num_cycles_specify=off  num_cycles_priority=High  num_cycles=0  num_cycles_nominal_specify=off  num_cycles_nominal_value=1  num_cycles_nominal_unit=1  cell_temperature_specify=off  cell_temperature_priority=High  cell_temperature=298.15 K  cell_temperature_nominal_specify=off  cell_temperature_nominal_value=1  cell_temperature_nominal_unit=K
      V0_mat=|
      | [3.0263, 3.218033, 3.364889, 3.493933, 3.610678, 3.733744, 3.85405, 3.950717, 4.040478, 4.0819;
      |  3.0376, 3.2248, 3.370311, 3.498533, 3.615311, 3.736956, 3.845633, 3.929256, 4.040056, 4.0821;
      |  3.0439, 3.227633, 3.3731, 3.5007, 3.616611, 3.737589, 3.8457, 3.9287, 4.039133, 4.0826;
      |  3.0283, 3.217989, 3.364589, 3.493767, 3.609467, 3.731156, 3.8417, 3.925833, 4.036322, 4.0821]' V
      R0_mat=|
      | [0.011867, 0.008993, 0.007674, 0.006911, 0.006648, 0.006648, 0.006528, 0.006157, 0.005996, 0.0073;
      |  0.0109, 0.006456, 0.005381, 0.005078, 0.005, 0.005044, 0.005511, 0.006407, 0.006522, 0.005367;
      |  0.0102, 0.007978, 0.006793, 0.0062, 0.006033, 0.005441, 0.0051, 0.005707, 0.005037, 0.005067;
      |  0.0101, 0.007759, 0.006637, 0.006022, 0.005741, 0.005667, 0.005311, 0.004911, 0.005859, 0.004733]' Ohm
      R1_mat=|
      | [0.007451, 0.008294, 0.007745, 0.007391;
      |  0.003783, 0.00363, 0.004415, 0.004051;
      |  0.002841, 0.00298, 0.003698, 0.003391;
      |  0.003185, 0.002661, 0.003493, 0.00379;
      |  0.00379, 0.003147, 0.004204, 0.004229;
      |  0.004015, 0.003677, 0.004233, 0.004481;
      |  0.003791, 0.004051, 0.003886, 0.004189;
      |  0.003416, 0.004883, 0.004387, 0.003743;
      |  0.00328, 0.005238, 0.003472, 0.004883;
      |  0.004816, 0.004218, 0.003847, 0.003891] Ohm
      tau1_mat=|
      | [8.156247, 6.866126, 6.747335, 6.573366;
      |  6.436096, 6.88158, 6.206576, 5.30011;
      |  7.074429, 7.267109, 6.564215, 5.759928;
      |  8.61232, 7.062398, 6.553799, 7.485573;
      |  10.88135, 8.569373, 8.681328, 8.99043;
      |  11.88702, 10.35435, 10.74073, 9.985533;
      |  11.15433, 10.61987, 10.52072, 10.95124;
      |  10.33388, 9.573709, 9.987626, 10.94588;
      |  9.883806, 9.219359, 8.513241, 9.109378;
      |  11.2706, 10.03414, 9.643065, 10.06297] s
      R2_mat=|
      | [0.040653, 0.04799, 0.046915, 0.044404;
      |  0.026828, 0.033189, 0.032279, 0.030363;
      |  0.019744, 0.025225, 0.021211, 0.019613;
      |  0.012414, 0.014827, 0.017004, 0.016763;
      |  0.007363, 0.008356, 0.01135, 0.010173;
      |  0.005882, 0.007703, 0.006532, 0.005526;
      |  0.006739, 0.007058, 0.006772, 0.005603;
      |  0.008222, 0.004287, 0.009601, 0.005034;
      |  0.008985, 0.007821, 0.008932, 0.006662;
      |  0.004704, 0.003171, 0.002422, 0.004036] Ohm
      tau2_mat=|
      | [131.6948, 137.0217, 141.2851, 129.3807;
      |  146.2759, 158.6208, 157.255, 143.944;
      |  158.5443, 177.3225, 156.7434, 144.0735;
      |  144.8009, 123.279, 145.0945, 176.1753;
      |  158.7596, 137.3241, 203.2495, 189.2199;
      |  149.8847, 154.5014, 161.1061, 146.3519;
      |  135.3572, 173.7062, 166.0613, 159.34;
      |  123.823, 144.5727, 209.652, 117.4544;
      |  111.7616, 98.04929, 114.3433, 98.05822;
      |  125.3862, 75.97092, 110.7081, 120.3015] s
      settings: InternalSimscapePortConfiguration="{\"Bottom\":[],\"Left\":[{\"id\":\"p\",\"label\":\"+\",\"type\":\"foundation.electrical.electrical\"}],\"Right\":[{\"id\":\"n\",\"label\":\"-\",\"type\":\"foundation.electrical.electrical\"}],\"Top\":[]}"
      settings: LibrarySourceBlock=|
      | batt_lib/Cells/Battery
      | (Table-Based)
  Battery (Table-Based)37 : batteryecm_lib/Battery (Table-Based)  SOC_vec=[0.1, 0.188889, 0.277778, 0.366667, 0.455556, 0.544444, 0.633333, 0.722222, 0.811111, 0.9]  T_dependence=simscape.enum.tablebattery.temperature_dependence.yes  prm_dir=simscape.enum.tablebattery.prm_dir.noCurrentDirectionality  T_vec=[30, 32.5, 35, 38] degC  V0_mat=|  V0_vec=[3.5057, 3.566, 3.6337, 3.7127, 3.9259, 4.0777, 4.1928] V  V_range=[0, inf] V  R0_mat=|  R0_vec=[.0085, .0085, .0087, .0082, .0083, .0085, .0085] Ohm  R0_dis_mat=[.0117, .0085, .009; .011, .0085, .009; .0114, .0087, .0092; .0107, .0082, .0088; .0107, .0083, .0091; .0113, .0085, .0089; .0116, .0085, .0089] Ohm  R0_dis_vec=[.0085, .0085, .0087, .0082, .0083, .0085, .0085] Ohm  R0_ch_mat=[.0117, .0085, .009; .011, .0085, .009; .0114, .0087, .0092; .0107, .0082, .0088; .0107, .0083, .0091; .0113, .0085, .0089; .0116, .0085, .0089] Ohm  R0_ch_vec=[.0085, .0085, .0087, .0082, .0083, .0085, .0085] Ohm  AH=5 A*hr  prm_leak=simscape.enum.tablebattery.prm_leak.disabled  Rleak_vec=[8000, 7000, 6000] Ohm  Rleak=7e3 Ohm  extrapolation_option=simscape.enum.extrapolation.nearest  SOC_port=simscape.enum.tablebattery.enable.no  prm_dyn=simscape.enum.tablebattery.prm_dyn.rc2  R1_mat=|  R1_vec=[.0029, .0024, .0026, .0016, .0023, .0018, .0017] Ohm  tau1_mat=|  tau1_vec=[36, 45, 105, 29, 77, 33, 39] s  R2_mat=|  R2_vec=[.0029, .0024, .0026, .0016, .0023, .0018, .0017] Ohm  tau2_mat=|  tau2_vec=[36, 45, 105, 29, 77, 33, 39] s  R3_mat=[.0109, .0029, .0013; .0069, .0024, .0012; .0047, .0026, .0013; .0034, .0016, .001; .0033, .0023, .0014; .0033, .0018, .0011; .0028, .0017, .0011] Ohm  R3_vec=[.0029, .0024, .0026, .0016, .0023, .0018, .0017] Ohm  tau3_mat=[20, 36, 39; 31, 45, 39; 109, 105, 61; 36, 29, 26; 59, 77, 67; 40, 33, 29; 25, 39, 33] s  tau3_vec=[36, 45, 105, 29, 77, 33, 39] s  R4_mat=[.0109, .0029, .0013; .0069, .0024, .0012; .0047, .0026, .0013; .0034, .0016, .001; .0033, .0023, .0014; .0033, .0018, .0011; .0028, .0017, .0011] Ohm  R4_vec=[.0029, .0024, .0026, .0016, .0023, .0018, .0017] Ohm  tau4_mat=[20, 36, 39; 31, 45, 39; 109, 105, 61; 36, 29, 26; 59, 77, 67; 40, 33, 29; 25, 39, 33] s  tau4_vec=[36, 45, 105, 29, 77, 33, 39] s  R5_mat=[.0109, .0029, .0013; .0069, .0024, .0012; .0047, .0026, .0013; .0034, .0016, .001; .0033, .0023, .0014; .0033, .0018, .0011; .0028, .0017, .0011] Ohm  R5_vec=[.0029, .0024, .0026, .0016, .0023, .0018, .0017] Ohm  tau5_mat=[20, 36, 39; 31, 45, 39; 109, 105, 61; 36, 29, 26; 59, 77, 67; 40, 33, 29; 25, 39, 33] s  tau5_vec=[36, 45, 105, 29, 77, 33, 39] s  prm_fade=simscape.enum.tablebattery.prm_fade.disabled  N0=100  dV0=0  dR0=0  dAH=0  dRleak=0  dR1=0  dR2=0  dR3=0  dR4=0  dR5=0  N0vec=[0, 100, 200, 300]  Tfadevec=[298.15, 323.15] K  dV0vec=[0, 0, 0, 0]  dR0vec=[0, 0, 0, 0]  dAHvec=[0, 0, 0, 0]  dRleakvec=[0, 0, 0, 0]  dR1vec=[0, 0, 0, 0]  dR2vec=[0, 0, 0, 0]  dR3vec=[0, 0, 0, 0]  dR4vec=[0, 0, 0, 0]  dR5vec=[0, 0, 0, 0]  dV0mat=[0, 0; 0, 0; 0, 0; 0, 0]  dR0mat=[0, 0; 0, 0; 0, 0; 0, 0]  dAHmat=[0, 0; 0, 0; 0, 0; 0, 0]  dRleakmat=[0, 0; 0, 0; 0, 0; 0, 0]  dR1mat=[0, 0; 0, 0; 0, 0; 0, 0]  dR2mat=[0, 0; 0, 0; 0, 0; 0, 0]  dR3mat=[0, 0; 0, 0; 0, 0; 0, 0]  dR4mat=[0, 0; 0, 0; 0, 0; 0, 0]  dR5mat=[0, 0; 0, 0; 0, 0; 0, 0]  prm_age_modeling=simscape.enum.tablebattery.prm_age_modeling.equation  storage_dt_age_vec=[0] d  storage_T_age_vec=[273] K  prm_age_OCV=simscape.enum.tablebattery.prm_age_OCV.OCV  OCV_age=0.9  SOC_age=0.6  prm_age_resistance=simscape.enum.tablebattery.prm_age.disabled  OCV_scaling_age_resistance=2.2134e6  OCV_offset_age_resistance=1.632e6  temp_exp_age_resistance=0.515833569 V  t_exp_age_resistance=0.75  T_age_vec_resistance=[273.15, 298.15, 323.15] K  dt_age_vec_resistance=[0, 90, 180, 270] d  dR0_age_vec=[0, 0, 0]  t_meas_dR0_age=100 d  dR0_age_mat=[0, 0, 0; 0, 0, 0; 0, 0, 0; 0, 0, 0]  prm_age_capacity=simscape.enum.tablebattery.prm_age.disabled  OCV_scaling_age_capacity=1.5097e07  OCV_offset_age_capacity=8.3625e06  temp_exp_age_capacity=0.6011 V  t_exp_age_capacity=0.75  T_age_vec_capacity=[273.15, 298.15, 323.15] K  dt_age_vec_capacity=[0, 90, 180, 270] d  dAH_age_vec=[0, 0, 0]  t_meas_dAH_age=100 d  dAH_age_mat=[0, 0, 0; 0, 0, 0; 0, 0, 0; 0, 0, 0]  thermal_port=simscape.enum.thermaleffects.omit  temperature=298.15 K  thermal_mass=100 J/K  i_specify=off  i_priority=None  i=0 A  i_nominal_specify=off  i_nominal_value=1  i_nominal_unit=A  v_specify=off  v_priority=None  v=0 V  v_nominal_specify=off  v_nominal_value=1  v_nominal_unit=V  stateOfCharge_specify=on  stateOfCharge_priority=High  stateOfCharge=1  stateOfCharge_nominal_specify=off  stateOfCharge_nominal_value=1  stateOfCharge_nominal_unit=1  num_cycles_specify=off  num_cycles_priority=High  num_cycles=0  num_cycles_nominal_specify=off  num_cycles_nominal_value=1  num_cycles_nominal_unit=1  cell_temperature_specify=off  cell_temperature_priority=High  cell_temperature=298.15 K  cell_temperature_nominal_specify=off  cell_temperature_nominal_value=1  cell_temperature_nominal_unit=K
      V0_mat=|
      | [3.0263, 3.218033, 3.364889, 3.493933, 3.610678, 3.733744, 3.85405, 3.950717, 4.040478, 4.0819;
      |  3.0376, 3.2248, 3.370311, 3.498533, 3.615311, 3.736956, 3.845633, 3.929256, 4.040056, 4.0821;
      |  3.0439, 3.227633, 3.3731, 3.5007, 3.616611, 3.737589, 3.8457, 3.9287, 4.039133, 4.0826;
      |  3.0283, 3.217989, 3.364589, 3.493767, 3.609467, 3.731156, 3.8417, 3.925833, 4.036322, 4.0821]' V
      R0_mat=|
      | [0.011867, 0.008993, 0.007674, 0.006911, 0.006648, 0.006648, 0.006528, 0.006157, 0.005996, 0.0073;
      |  0.0109, 0.006456, 0.005381, 0.005078, 0.005, 0.005044, 0.005511, 0.006407, 0.006522, 0.005367;
      |  0.0102, 0.007978, 0.006793, 0.0062, 0.006033, 0.005441, 0.0051, 0.005707, 0.005037, 0.005067;
      |  0.0101, 0.007759, 0.006637, 0.006022, 0.005741, 0.005667, 0.005311, 0.004911, 0.005859, 0.004733]' Ohm
      R1_mat=|
      | [0.007451, 0.008294, 0.007745, 0.007391;
      |  0.003783, 0.00363, 0.004415, 0.004051;
      |  0.002841, 0.00298, 0.003698, 0.003391;
      |  0.003185, 0.002661, 0.003493, 0.00379;
      |  0.00379, 0.003147, 0.004204, 0.004229;
      |  0.004015, 0.003677, 0.004233, 0.004481;
      |  0.003791, 0.004051, 0.003886, 0.004189;
      |  0.003416, 0.004883, 0.004387, 0.003743;
      |  0.00328, 0.005238, 0.003472, 0.004883;
      |  0.004816, 0.004218, 0.003847, 0.003891] Ohm
      tau1_mat=|
      | [8.156247, 6.866126, 6.747335, 6.573366;
      |  6.436096, 6.88158, 6.206576, 5.30011;
      |  7.074429, 7.267109, 6.564215, 5.759928;
      |  8.61232, 7.062398, 6.553799, 7.485573;
      |  10.88135, 8.569373, 8.681328, 8.99043;
      |  11.88702, 10.35435, 10.74073, 9.985533;
      |  11.15433, 10.61987, 10.52072, 10.95124;
      |  10.33388, 9.573709, 9.987626, 10.94588;
      |  9.883806, 9.219359, 8.513241, 9.109378;
      |  11.2706, 10.03414, 9.643065, 10.06297] s
      R2_mat=|
      | [0.040653, 0.04799, 0.046915, 0.044404;
      |  0.026828, 0.033189, 0.032279, 0.030363;
      |  0.019744, 0.025225, 0.021211, 0.019613;
      |  0.012414, 0.014827, 0.017004, 0.016763;
      |  0.007363, 0.008356, 0.01135, 0.010173;
      |  0.005882, 0.007703, 0.006532, 0.005526;
      |  0.006739, 0.007058, 0.006772, 0.005603;
      |  0.008222, 0.004287, 0.009601, 0.005034;
      |  0.008985, 0.007821, 0.008932, 0.006662;
      |  0.004704, 0.003171, 0.002422, 0.004036] Ohm
      tau2_mat=|
      | [131.6948, 137.0217, 141.2851, 129.3807;
      |  146.2759, 158.6208, 157.255, 143.944;
      |  158.5443, 177.3225, 156.7434, 144.0735;
      |  144.8009, 123.279, 145.0945, 176.1753;
      |  158.7596, 137.3241, 203.2495, 189.2199;
      |  149.8847, 154.5014, 161.1061, 146.3519;
      |  135.3572, 173.7062, 166.0613, 159.34;
      |  123.823, 144.5727, 209.652, 117.4544;
      |  111.7616, 98.04929, 114.3433, 98.05822;
      |  125.3862, 75.97092, 110.7081, 120.3015] s
      settings: InternalSimscapePortConfiguration="{\"Bottom\":[],\"Left\":[{\"id\":\"p\",\"label\":\"+\",\"type\":\"foundation.electrical.electrical\"}],\"Right\":[{\"id\":\"n\",\"label\":\"-\",\"type\":\"foundation.electrical.electrical\"}],\"Top\":[]}"
      settings: LibrarySourceBlock=|
      | batt_lib/Cells/Battery
      | (Table-Based)
  Battery (Table-Based)38 : batteryecm_lib/Battery (Table-Based)  SOC_vec=[0.1, 0.188889, 0.277778, 0.366667, 0.455556, 0.544444, 0.633333, 0.722222, 0.811111, 0.9]  T_dependence=simscape.enum.tablebattery.temperature_dependence.yes  prm_dir=simscape.enum.tablebattery.prm_dir.noCurrentDirectionality  T_vec=[30, 32.5, 35, 38] degC  V0_mat=|  V0_vec=[3.5057, 3.566, 3.6337, 3.7127, 3.9259, 4.0777, 4.1928] V  V_range=[0, inf] V  R0_mat=|  R0_vec=[.0085, .0085, .0087, .0082, .0083, .0085, .0085] Ohm  R0_dis_mat=[.0117, .0085, .009; .011, .0085, .009; .0114, .0087, .0092; .0107, .0082, .0088; .0107, .0083, .0091; .0113, .0085, .0089; .0116, .0085, .0089] Ohm  R0_dis_vec=[.0085, .0085, .0087, .0082, .0083, .0085, .0085] Ohm  R0_ch_mat=[.0117, .0085, .009; .011, .0085, .009; .0114, .0087, .0092; .0107, .0082, .0088; .0107, .0083, .0091; .0113, .0085, .0089; .0116, .0085, .0089] Ohm  R0_ch_vec=[.0085, .0085, .0087, .0082, .0083, .0085, .0085] Ohm  AH=5 A*hr  prm_leak=simscape.enum.tablebattery.prm_leak.disabled  Rleak_vec=[8000, 7000, 6000] Ohm  Rleak=7e3 Ohm  extrapolation_option=simscape.enum.extrapolation.nearest  SOC_port=simscape.enum.tablebattery.enable.no  prm_dyn=simscape.enum.tablebattery.prm_dyn.rc2  R1_mat=|  R1_vec=[.0029, .0024, .0026, .0016, .0023, .0018, .0017] Ohm  tau1_mat=|  tau1_vec=[36, 45, 105, 29, 77, 33, 39] s  R2_mat=|  R2_vec=[.0029, .0024, .0026, .0016, .0023, .0018, .0017] Ohm  tau2_mat=|  tau2_vec=[36, 45, 105, 29, 77, 33, 39] s  R3_mat=[.0109, .0029, .0013; .0069, .0024, .0012; .0047, .0026, .0013; .0034, .0016, .001; .0033, .0023, .0014; .0033, .0018, .0011; .0028, .0017, .0011] Ohm  R3_vec=[.0029, .0024, .0026, .0016, .0023, .0018, .0017] Ohm  tau3_mat=[20, 36, 39; 31, 45, 39; 109, 105, 61; 36, 29, 26; 59, 77, 67; 40, 33, 29; 25, 39, 33] s  tau3_vec=[36, 45, 105, 29, 77, 33, 39] s  R4_mat=[.0109, .0029, .0013; .0069, .0024, .0012; .0047, .0026, .0013; .0034, .0016, .001; .0033, .0023, .0014; .0033, .0018, .0011; .0028, .0017, .0011] Ohm  R4_vec=[.0029, .0024, .0026, .0016, .0023, .0018, .0017] Ohm  tau4_mat=[20, 36, 39; 31, 45, 39; 109, 105, 61; 36, 29, 26; 59, 77, 67; 40, 33, 29; 25, 39, 33] s  tau4_vec=[36, 45, 105, 29, 77, 33, 39] s  R5_mat=[.0109, .0029, .0013; .0069, .0024, .0012; .0047, .0026, .0013; .0034, .0016, .001; .0033, .0023, .0014; .0033, .0018, .0011; .0028, .0017, .0011] Ohm  R5_vec=[.0029, .0024, .0026, .0016, .0023, .0018, .0017] Ohm  tau5_mat=[20, 36, 39; 31, 45, 39; 109, 105, 61; 36, 29, 26; 59, 77, 67; 40, 33, 29; 25, 39, 33] s  tau5_vec=[36, 45, 105, 29, 77, 33, 39] s  prm_fade=simscape.enum.tablebattery.prm_fade.disabled  N0=100  dV0=0  dR0=0  dAH=0  dRleak=0  dR1=0  dR2=0  dR3=0  dR4=0  dR5=0  N0vec=[0, 100, 200, 300]  Tfadevec=[298.15, 323.15] K  dV0vec=[0, 0, 0, 0]  dR0vec=[0, 0, 0, 0]  dAHvec=[0, 0, 0, 0]  dRleakvec=[0, 0, 0, 0]  dR1vec=[0, 0, 0, 0]  dR2vec=[0, 0, 0, 0]  dR3vec=[0, 0, 0, 0]  dR4vec=[0, 0, 0, 0]  dR5vec=[0, 0, 0, 0]  dV0mat=[0, 0; 0, 0; 0, 0; 0, 0]  dR0mat=[0, 0; 0, 0; 0, 0; 0, 0]  dAHmat=[0, 0; 0, 0; 0, 0; 0, 0]  dRleakmat=[0, 0; 0, 0; 0, 0; 0, 0]  dR1mat=[0, 0; 0, 0; 0, 0; 0, 0]  dR2mat=[0, 0; 0, 0; 0, 0; 0, 0]  dR3mat=[0, 0; 0, 0; 0, 0; 0, 0]  dR4mat=[0, 0; 0, 0; 0, 0; 0, 0]  dR5mat=[0, 0; 0, 0; 0, 0; 0, 0]  prm_age_modeling=simscape.enum.tablebattery.prm_age_modeling.equation  storage_dt_age_vec=[0] d  storage_T_age_vec=[273] K  prm_age_OCV=simscape.enum.tablebattery.prm_age_OCV.OCV  OCV_age=0.9  SOC_age=0.6  prm_age_resistance=simscape.enum.tablebattery.prm_age.disabled  OCV_scaling_age_resistance=2.2134e6  OCV_offset_age_resistance=1.632e6  temp_exp_age_resistance=0.515833569 V  t_exp_age_resistance=0.75  T_age_vec_resistance=[273.15, 298.15, 323.15] K  dt_age_vec_resistance=[0, 90, 180, 270] d  dR0_age_vec=[0, 0, 0]  t_meas_dR0_age=100 d  dR0_age_mat=[0, 0, 0; 0, 0, 0; 0, 0, 0; 0, 0, 0]  prm_age_capacity=simscape.enum.tablebattery.prm_age.disabled  OCV_scaling_age_capacity=1.5097e07  OCV_offset_age_capacity=8.3625e06  temp_exp_age_capacity=0.6011 V  t_exp_age_capacity=0.75  T_age_vec_capacity=[273.15, 298.15, 323.15] K  dt_age_vec_capacity=[0, 90, 180, 270] d  dAH_age_vec=[0, 0, 0]  t_meas_dAH_age=100 d  dAH_age_mat=[0, 0, 0; 0, 0, 0; 0, 0, 0; 0, 0, 0]  thermal_port=simscape.enum.thermaleffects.omit  temperature=298.15 K  thermal_mass=100 J/K  i_specify=off  i_priority=None  i=0 A  i_nominal_specify=off  i_nominal_value=1  i_nominal_unit=A  v_specify=off  v_priority=None  v=0 V  v_nominal_specify=off  v_nominal_value=1  v_nominal_unit=V  stateOfCharge_specify=on  stateOfCharge_priority=High  stateOfCharge=1  stateOfCharge_nominal_specify=off  stateOfCharge_nominal_value=1  stateOfCharge_nominal_unit=1  num_cycles_specify=off  num_cycles_priority=High  num_cycles=0  num_cycles_nominal_specify=off  num_cycles_nominal_value=1  num_cycles_nominal_unit=1  cell_temperature_specify=off  cell_temperature_priority=High  cell_temperature=298.15 K  cell_temperature_nominal_specify=off  cell_temperature_nominal_value=1  cell_temperature_nominal_unit=K
      V0_mat=|
      | [3.0263, 3.218033, 3.364889, 3.493933, 3.610678, 3.733744, 3.85405, 3.950717, 4.040478, 4.0819;
      |  3.0376, 3.2248, 3.370311, 3.498533, 3.615311, 3.736956, 3.845633, 3.929256, 4.040056, 4.0821;
      |  3.0439, 3.227633, 3.3731, 3.5007, 3.616611, 3.737589, 3.8457, 3.9287, 4.039133, 4.0826;
      |  3.0283, 3.217989, 3.364589, 3.493767, 3.609467, 3.731156, 3.8417, 3.925833, 4.036322, 4.0821]' V
      R0_mat=|
      | [0.011867, 0.008993, 0.007674, 0.006911, 0.006648, 0.006648, 0.006528, 0.006157, 0.005996, 0.0073;
      |  0.0109, 0.006456, 0.005381, 0.005078, 0.005, 0.005044, 0.005511, 0.006407, 0.006522, 0.005367;
      |  0.0102, 0.007978, 0.006793, 0.0062, 0.006033, 0.005441, 0.0051, 0.005707, 0.005037, 0.005067;
      |  0.0101, 0.007759, 0.006637, 0.006022, 0.005741, 0.005667, 0.005311, 0.004911, 0.005859, 0.004733]' Ohm
      R1_mat=|
      | [0.007451, 0.008294, 0.007745, 0.007391;
      |  0.003783, 0.00363, 0.004415, 0.004051;
      |  0.002841, 0.00298, 0.003698, 0.003391;
      |  0.003185, 0.002661, 0.003493, 0.00379;
      |  0.00379, 0.003147, 0.004204, 0.004229;
      |  0.004015, 0.003677, 0.004233, 0.004481;
      |  0.003791, 0.004051, 0.003886, 0.004189;
      |  0.003416, 0.004883, 0.004387, 0.003743;
      |  0.00328, 0.005238, 0.003472, 0.004883;
      |  0.004816, 0.004218, 0.003847, 0.003891] Ohm
      tau1_mat=|
      | [8.156247, 6.866126, 6.747335, 6.573366;
      |  6.436096, 6.88158, 6.206576, 5.30011;
      |  7.074429, 7.267109, 6.564215, 5.759928;
      |  8.61232, 7.062398, 6.553799, 7.485573;
      |  10.88135, 8.569373, 8.681328, 8.99043;
      |  11.88702, 10.35435, 10.74073, 9.985533;
      |  11.15433, 10.61987, 10.52072, 10.95124;
      |  10.33388, 9.573709, 9.987626, 10.94588;
      |  9.883806, 9.219359, 8.513241, 9.109378;
      |  11.2706, 10.03414, 9.643065, 10.06297] s
      R2_mat=|
      | [0.040653, 0.04799, 0.046915, 0.044404;
      |  0.026828, 0.033189, 0.032279, 0.030363;
      |  0.019744, 0.025225, 0.021211, 0.019613;
      |  0.012414, 0.014827, 0.017004, 0.016763;
      |  0.007363, 0.008356, 0.01135, 0.010173;
      |  0.005882, 0.007703, 0.006532, 0.005526;
      |  0.006739, 0.007058, 0.006772, 0.005603;
      |  0.008222, 0.004287, 0.009601, 0.005034;
      |  0.008985, 0.007821, 0.008932, 0.006662;
      |  0.004704, 0.003171, 0.002422, 0.004036] Ohm
      tau2_mat=|
      | [131.6948, 137.0217, 141.2851, 129.3807;
      |  146.2759, 158.6208, 157.255, 143.944;
      |  158.5443, 177.3225, 156.7434, 144.0735;
      |  144.8009, 123.279, 145.0945, 176.1753;
      |  158.7596, 137.3241, 203.2495, 189.2199;
      |  149.8847, 154.5014, 161.1061, 146.3519;
      |  135.3572, 173.7062, 166.0613, 159.34;
      |  123.823, 144.5727, 209.652, 117.4544;
      |  111.7616, 98.04929, 114.3433, 98.05822;
      |  125.3862, 75.97092, 110.7081, 120.3015] s
      settings: InternalSimscapePortConfiguration="{\"Bottom\":[],\"Left\":[{\"id\":\"p\",\"label\":\"+\",\"type\":\"foundation.electrical.electrical\"}],\"Right\":[{\"id\":\"n\",\"label\":\"-\",\"type\":\"foundation.electrical.electrical\"}],\"Top\":[]}"
      settings: LibrarySourceBlock=|
      | batt_lib/Cells/Battery
      | (Table-Based)
  Battery (Table-Based)39 : batteryecm_lib/Battery (Table-Based)  SOC_vec=[0.1, 0.188889, 0.277778, 0.366667, 0.455556, 0.544444, 0.633333, 0.722222, 0.811111, 0.9]  T_dependence=simscape.enum.tablebattery.temperature_dependence.yes  prm_dir=simscape.enum.tablebattery.prm_dir.noCurrentDirectionality  T_vec=[30, 32.5, 35, 38] degC  V0_mat=|  V0_vec=[3.5057, 3.566, 3.6337, 3.7127, 3.9259, 4.0777, 4.1928] V  V_range=[0, inf] V  R0_mat=|  R0_vec=[.0085, .0085, .0087, .0082, .0083, .0085, .0085] Ohm  R0_dis_mat=[.0117, .0085, .009; .011, .0085, .009; .0114, .0087, .0092; .0107, .0082, .0088; .0107, .0083, .0091; .0113, .0085, .0089; .0116, .0085, .0089] Ohm  R0_dis_vec=[.0085, .0085, .0087, .0082, .0083, .0085, .0085] Ohm  R0_ch_mat=[.0117, .0085, .009; .011, .0085, .009; .0114, .0087, .0092; .0107, .0082, .0088; .0107, .0083, .0091; .0113, .0085, .0089; .0116, .0085, .0089] Ohm  R0_ch_vec=[.0085, .0085, .0087, .0082, .0083, .0085, .0085] Ohm  AH=5 A*hr  prm_leak=simscape.enum.tablebattery.prm_leak.disabled  Rleak_vec=[8000, 7000, 6000] Ohm  Rleak=7e3 Ohm  extrapolation_option=simscape.enum.extrapolation.nearest  SOC_port=simscape.enum.tablebattery.enable.no  prm_dyn=simscape.enum.tablebattery.prm_dyn.rc2  R1_mat=|  R1_vec=[.0029, .0024, .0026, .0016, .0023, .0018, .0017] Ohm  tau1_mat=|  tau1_vec=[36, 45, 105, 29, 77, 33, 39] s  R2_mat=|  R2_vec=[.0029, .0024, .0026, .0016, .0023, .0018, .0017] Ohm  tau2_mat=|  tau2_vec=[36, 45, 105, 29, 77, 33, 39] s  R3_mat=[.0109, .0029, .0013; .0069, .0024, .0012; .0047, .0026, .0013; .0034, .0016, .001; .0033, .0023, .0014; .0033, .0018, .0011; .0028, .0017, .0011] Ohm  R3_vec=[.0029, .0024, .0026, .0016, .0023, .0018, .0017] Ohm  tau3_mat=[20, 36, 39; 31, 45, 39; 109, 105, 61; 36, 29, 26; 59, 77, 67; 40, 33, 29; 25, 39, 33] s  tau3_vec=[36, 45, 105, 29, 77, 33, 39] s  R4_mat=[.0109, .0029, .0013; .0069, .0024, .0012; .0047, .0026, .0013; .0034, .0016, .001; .0033, .0023, .0014; .0033, .0018, .0011; .0028, .0017, .0011] Ohm  R4_vec=[.0029, .0024, .0026, .0016, .0023, .0018, .0017] Ohm  tau4_mat=[20, 36, 39; 31, 45, 39; 109, 105, 61; 36, 29, 26; 59, 77, 67; 40, 33, 29; 25, 39, 33] s  tau4_vec=[36, 45, 105, 29, 77, 33, 39] s  R5_mat=[.0109, .0029, .0013; .0069, .0024, .0012; .0047, .0026, .0013; .0034, .0016, .001; .0033, .0023, .0014; .0033, .0018, .0011; .0028, .0017, .0011] Ohm  R5_vec=[.0029, .0024, .0026, .0016, .0023, .0018, .0017] Ohm  tau5_mat=[20, 36, 39; 31, 45, 39; 109, 105, 61; 36, 29, 26; 59, 77, 67; 40, 33, 29; 25, 39, 33] s  tau5_vec=[36, 45, 105, 29, 77, 33, 39] s  prm_fade=simscape.enum.tablebattery.prm_fade.disabled  N0=100  dV0=0  dR0=0  dAH=0  dRleak=0  dR1=0  dR2=0  dR3=0  dR4=0  dR5=0  N0vec=[0, 100, 200, 300]  Tfadevec=[298.15, 323.15] K  dV0vec=[0, 0, 0, 0]  dR0vec=[0, 0, 0, 0]  dAHvec=[0, 0, 0, 0]  dRleakvec=[0, 0, 0, 0]  dR1vec=[0, 0, 0, 0]  dR2vec=[0, 0, 0, 0]  dR3vec=[0, 0, 0, 0]  dR4vec=[0, 0, 0, 0]  dR5vec=[0, 0, 0, 0]  dV0mat=[0, 0; 0, 0; 0, 0; 0, 0]  dR0mat=[0, 0; 0, 0; 0, 0; 0, 0]  dAHmat=[0, 0; 0, 0; 0, 0; 0, 0]  dRleakmat=[0, 0; 0, 0; 0, 0; 0, 0]  dR1mat=[0, 0; 0, 0; 0, 0; 0, 0]  dR2mat=[0, 0; 0, 0; 0, 0; 0, 0]  dR3mat=[0, 0; 0, 0; 0, 0; 0, 0]  dR4mat=[0, 0; 0, 0; 0, 0; 0, 0]  dR5mat=[0, 0; 0, 0; 0, 0; 0, 0]  prm_age_modeling=simscape.enum.tablebattery.prm_age_modeling.equation  storage_dt_age_vec=[0] d  storage_T_age_vec=[273] K  prm_age_OCV=simscape.enum.tablebattery.prm_age_OCV.OCV  OCV_age=0.9  SOC_age=0.6  prm_age_resistance=simscape.enum.tablebattery.prm_age.disabled  OCV_scaling_age_resistance=2.2134e6  OCV_offset_age_resistance=1.632e6  temp_exp_age_resistance=0.515833569 V  t_exp_age_resistance=0.75  T_age_vec_resistance=[273.15, 298.15, 323.15] K  dt_age_vec_resistance=[0, 90, 180, 270] d  dR0_age_vec=[0, 0, 0]  t_meas_dR0_age=100 d  dR0_age_mat=[0, 0, 0; 0, 0, 0; 0, 0, 0; 0, 0, 0]  prm_age_capacity=simscape.enum.tablebattery.prm_age.disabled  OCV_scaling_age_capacity=1.5097e07  OCV_offset_age_capacity=8.3625e06  temp_exp_age_capacity=0.6011 V  t_exp_age_capacity=0.75  T_age_vec_capacity=[273.15, 298.15, 323.15] K  dt_age_vec_capacity=[0, 90, 180, 270] d  dAH_age_vec=[0, 0, 0]  t_meas_dAH_age=100 d  dAH_age_mat=[0, 0, 0; 0, 0, 0; 0, 0, 0; 0, 0, 0]  thermal_port=simscape.enum.thermaleffects.omit  temperature=298.15 K  thermal_mass=100 J/K  i_specify=off  i_priority=None  i=0 A  i_nominal_specify=off  i_nominal_value=1  i_nominal_unit=A  v_specify=off  v_priority=None  v=0 V  v_nominal_specify=off  v_nominal_value=1  v_nominal_unit=V  stateOfCharge_specify=on  stateOfCharge_priority=High  stateOfCharge=1  stateOfCharge_nominal_specify=off  stateOfCharge_nominal_value=1  stateOfCharge_nominal_unit=1  num_cycles_specify=off  num_cycles_priority=High  num_cycles=0  num_cycles_nominal_specify=off  num_cycles_nominal_value=1  num_cycles_nominal_unit=1  cell_temperature_specify=off  cell_temperature_priority=High  cell_temperature=298.15 K  cell_temperature_nominal_specify=off  cell_temperature_nominal_value=1  cell_temperature_nominal_unit=K
      V0_mat=|
      | [3.0263, 3.218033, 3.364889, 3.493933, 3.610678, 3.733744, 3.85405, 3.950717, 4.040478, 4.0819;
      |  3.0376, 3.2248, 3.370311, 3.498533, 3.615311, 3.736956, 3.845633, 3.929256, 4.040056, 4.0821;
      |  3.0439, 3.227633, 3.3731, 3.5007, 3.616611, 3.737589, 3.8457, 3.9287, 4.039133, 4.0826;
      |  3.0283, 3.217989, 3.364589, 3.493767, 3.609467, 3.731156, 3.8417, 3.925833, 4.036322, 4.0821]' V
      R0_mat=|
      | [0.011867, 0.008993, 0.007674, 0.006911, 0.006648, 0.006648, 0.006528, 0.006157, 0.005996, 0.0073;
      |  0.0109, 0.006456, 0.005381, 0.005078, 0.005, 0.005044, 0.005511, 0.006407, 0.006522, 0.005367;
      |  0.0102, 0.007978, 0.006793, 0.0062, 0.006033, 0.005441, 0.0051, 0.005707, 0.005037, 0.005067;
      |  0.0101, 0.007759, 0.006637, 0.006022, 0.005741, 0.005667, 0.005311, 0.004911, 0.005859, 0.004733]' Ohm
      R1_mat=|
      | [0.007451, 0.008294, 0.007745, 0.007391;
      |  0.003783, 0.00363, 0.004415, 0.004051;
      |  0.002841, 0.00298, 0.003698, 0.003391;
      |  0.003185, 0.002661, 0.003493, 0.00379;
      |  0.00379, 0.003147, 0.004204, 0.004229;
      |  0.004015, 0.003677, 0.004233, 0.004481;
      |  0.003791, 0.004051, 0.003886, 0.004189;
      |  0.003416, 0.004883, 0.004387, 0.003743;
      |  0.00328, 0.005238, 0.003472, 0.004883;
      |  0.004816, 0.004218, 0.003847, 0.003891] Ohm
      tau1_mat=|
      | [8.156247, 6.866126, 6.747335, 6.573366;
      |  6.436096, 6.88158, 6.206576, 5.30011;
      |  7.074429, 7.267109, 6.564215, 5.759928;
      |  8.61232, 7.062398, 6.553799, 7.485573;
      |  10.88135, 8.569373, 8.681328, 8.99043;
      |  11.88702, 10.35435, 10.74073, 9.985533;
      |  11.15433, 10.61987, 10.52072, 10.95124;
      |  10.33388, 9.573709, 9.987626, 10.94588;
      |  9.883806, 9.219359, 8.513241, 9.109378;
      |  11.2706, 10.03414, 9.643065, 10.06297] s
      R2_mat=|
      | [0.040653, 0.04799, 0.046915, 0.044404;
      |  0.026828, 0.033189, 0.032279, 0.030363;
      |  0.019744, 0.025225, 0.021211, 0.019613;
      |  0.012414, 0.014827, 0.017004, 0.016763;
      |  0.007363, 0.008356, 0.01135, 0.010173;
      |  0.005882, 0.007703, 0.006532, 0.005526;
      |  0.006739, 0.007058, 0.006772, 0.005603;
      |  0.008222, 0.004287, 0.009601, 0.005034;
      |  0.008985, 0.007821, 0.008932, 0.006662;
      |  0.004704, 0.003171, 0.002422, 0.004036] Ohm
      tau2_mat=|
      | [131.6948, 137.0217, 141.2851, 129.3807;
      |  146.2759, 158.6208, 157.255, 143.944;
      |  158.5443, 177.3225, 156.7434, 144.0735;
      |  144.8009, 123.279, 145.0945, 176.1753;
      |  158.7596, 137.3241, 203.2495, 189.2199;
      |  149.8847, 154.5014, 161.1061, 146.3519;
      |  135.3572, 173.7062, 166.0613, 159.34;
      |  123.823, 144.5727, 209.652, 117.4544;
      |  111.7616, 98.04929, 114.3433, 98.05822;
      |  125.3862, 75.97092, 110.7081, 120.3015] s
      settings: InternalSimscapePortConfiguration="{\"Bottom\":[],\"Left\":[{\"id\":\"p\",\"label\":\"+\",\"type\":\"foundation.electrical.electrical\"}],\"Right\":[{\"id\":\"n\",\"label\":\"-\",\"type\":\"foundation.electrical.electrical\"}],\"Top\":[]}"
      settings: LibrarySourceBlock=|
      | batt_lib/Cells/Battery
      | (Table-Based)
  Battery (Table-Based)4 : batteryecm_lib/Battery (Table-Based)  SOC_vec=[0.1, 0.188889, 0.277778, 0.366667, 0.455556, 0.544444, 0.633333, 0.722222, 0.811111, 0.9]  T_dependence=simscape.enum.tablebattery.temperature_dependence.yes  prm_dir=simscape.enum.tablebattery.prm_dir.noCurrentDirectionality  T_vec=[30, 32.5, 35, 38] degC  V0_mat=|  V0_vec=[3.5057, 3.566, 3.6337, 3.7127, 3.9259, 4.0777, 4.1928] V  V_range=[0, inf] V  R0_mat=|  R0_vec=[.0085, .0085, .0087, .0082, .0083, .0085, .0085] Ohm  R0_dis_mat=[.0117, .0085, .009; .011, .0085, .009; .0114, .0087, .0092; .0107, .0082, .0088; .0107, .0083, .0091; .0113, .0085, .0089; .0116, .0085, .0089] Ohm  R0_dis_vec=[.0085, .0085, .0087, .0082, .0083, .0085, .0085] Ohm  R0_ch_mat=[.0117, .0085, .009; .011, .0085, .009; .0114, .0087, .0092; .0107, .0082, .0088; .0107, .0083, .0091; .0113, .0085, .0089; .0116, .0085, .0089] Ohm  R0_ch_vec=[.0085, .0085, .0087, .0082, .0083, .0085, .0085] Ohm  AH=5 A*hr  prm_leak=simscape.enum.tablebattery.prm_leak.disabled  Rleak_vec=[8000, 7000, 6000] Ohm  Rleak=7e3 Ohm  extrapolation_option=simscape.enum.extrapolation.nearest  SOC_port=simscape.enum.tablebattery.enable.no  prm_dyn=simscape.enum.tablebattery.prm_dyn.rc2  R1_mat=|  R1_vec=[.0029, .0024, .0026, .0016, .0023, .0018, .0017] Ohm  tau1_mat=|  tau1_vec=[36, 45, 105, 29, 77, 33, 39] s  R2_mat=|  R2_vec=[.0029, .0024, .0026, .0016, .0023, .0018, .0017] Ohm  tau2_mat=|  tau2_vec=[36, 45, 105, 29, 77, 33, 39] s  R3_mat=[.0109, .0029, .0013; .0069, .0024, .0012; .0047, .0026, .0013; .0034, .0016, .001; .0033, .0023, .0014; .0033, .0018, .0011; .0028, .0017, .0011] Ohm  R3_vec=[.0029, .0024, .0026, .0016, .0023, .0018, .0017] Ohm  tau3_mat=[20, 36, 39; 31, 45, 39; 109, 105, 61; 36, 29, 26; 59, 77, 67; 40, 33, 29; 25, 39, 33] s  tau3_vec=[36, 45, 105, 29, 77, 33, 39] s  R4_mat=[.0109, .0029, .0013; .0069, .0024, .0012; .0047, .0026, .0013; .0034, .0016, .001; .0033, .0023, .0014; .0033, .0018, .0011; .0028, .0017, .0011] Ohm  R4_vec=[.0029, .0024, .0026, .0016, .0023, .0018, .0017] Ohm  tau4_mat=[20, 36, 39; 31, 45, 39; 109, 105, 61; 36, 29, 26; 59, 77, 67; 40, 33, 29; 25, 39, 33] s  tau4_vec=[36, 45, 105, 29, 77, 33, 39] s  R5_mat=[.0109, .0029, .0013; .0069, .0024, .0012; .0047, .0026, .0013; .0034, .0016, .001; .0033, .0023, .0014; .0033, .0018, .0011; .0028, .0017, .0011] Ohm  R5_vec=[.0029, .0024, .0026, .0016, .0023, .0018, .0017] Ohm  tau5_mat=[20, 36, 39; 31, 45, 39; 109, 105, 61; 36, 29, 26; 59, 77, 67; 40, 33, 29; 25, 39, 33] s  tau5_vec=[36, 45, 105, 29, 77, 33, 39] s  prm_fade=simscape.enum.tablebattery.prm_fade.disabled  N0=100  dV0=0  dR0=0  dAH=0  dRleak=0  dR1=0  dR2=0  dR3=0  dR4=0  dR5=0  N0vec=[0, 100, 200, 300]  Tfadevec=[298.15, 323.15] K  dV0vec=[0, 0, 0, 0]  dR0vec=[0, 0, 0, 0]  dAHvec=[0, 0, 0, 0]  dRleakvec=[0, 0, 0, 0]  dR1vec=[0, 0, 0, 0]  dR2vec=[0, 0, 0, 0]  dR3vec=[0, 0, 0, 0]  dR4vec=[0, 0, 0, 0]  dR5vec=[0, 0, 0, 0]  dV0mat=[0, 0; 0, 0; 0, 0; 0, 0]  dR0mat=[0, 0; 0, 0; 0, 0; 0, 0]  dAHmat=[0, 0; 0, 0; 0, 0; 0, 0]  dRleakmat=[0, 0; 0, 0; 0, 0; 0, 0]  dR1mat=[0, 0; 0, 0; 0, 0; 0, 0]  dR2mat=[0, 0; 0, 0; 0, 0; 0, 0]  dR3mat=[0, 0; 0, 0; 0, 0; 0, 0]  dR4mat=[0, 0; 0, 0; 0, 0; 0, 0]  dR5mat=[0, 0; 0, 0; 0, 0; 0, 0]  prm_age_modeling=simscape.enum.tablebattery.prm_age_modeling.equation  storage_dt_age_vec=[0] d  storage_T_age_vec=[273] K  prm_age_OCV=simscape.enum.tablebattery.prm_age_OCV.OCV  OCV_age=0.9  SOC_age=0.6  prm_age_resistance=simscape.enum.tablebattery.prm_age.disabled  OCV_scaling_age_resistance=2.2134e6  OCV_offset_age_resistance=1.632e6  temp_exp_age_resistance=0.515833569 V  t_exp_age_resistance=0.75  T_age_vec_resistance=[273.15, 298.15, 323.15] K  dt_age_vec_resistance=[0, 90, 180, 270] d  dR0_age_vec=[0, 0, 0]  t_meas_dR0_age=100 d  dR0_age_mat=[0, 0, 0; 0, 0, 0; 0, 0, 0; 0, 0, 0]  prm_age_capacity=simscape.enum.tablebattery.prm_age.disabled  OCV_scaling_age_capacity=1.5097e07  OCV_offset_age_capacity=8.3625e06  temp_exp_age_capacity=0.6011 V  t_exp_age_capacity=0.75  T_age_vec_capacity=[273.15, 298.15, 323.15] K  dt_age_vec_capacity=[0, 90, 180, 270] d  dAH_age_vec=[0, 0, 0]  t_meas_dAH_age=100 d  dAH_age_mat=[0, 0, 0; 0, 0, 0; 0, 0, 0; 0, 0, 0]  thermal_port=simscape.enum.thermaleffects.omit  temperature=298.15 K  thermal_mass=100 J/K  i_specify=off  i_priority=None  i=0 A  i_nominal_specify=off  i_nominal_value=1  i_nominal_unit=A  v_specify=off  v_priority=None  v=0 V  v_nominal_specify=off  v_nominal_value=1  v_nominal_unit=V  stateOfCharge_specify=on  stateOfCharge_priority=High  stateOfCharge=1  stateOfCharge_nominal_specify=off  stateOfCharge_nominal_value=1  stateOfCharge_nominal_unit=1  num_cycles_specify=off  num_cycles_priority=High  num_cycles=0  num_cycles_nominal_specify=off  num_cycles_nominal_value=1  num_cycles_nominal_unit=1  cell_temperature_specify=off  cell_temperature_priority=High  cell_temperature=298.15 K  cell_temperature_nominal_specify=off  cell_temperature_nominal_value=1  cell_temperature_nominal_unit=K
      V0_mat=|
      | [3.0263, 3.218033, 3.364889, 3.493933, 3.610678, 3.733744, 3.85405, 3.950717, 4.040478, 4.0819;
      |  3.0376, 3.2248, 3.370311, 3.498533, 3.615311, 3.736956, 3.845633, 3.929256, 4.040056, 4.0821;
      |  3.0439, 3.227633, 3.3731, 3.5007, 3.616611, 3.737589, 3.8457, 3.9287, 4.039133, 4.0826;
      |  3.0283, 3.217989, 3.364589, 3.493767, 3.609467, 3.731156, 3.8417, 3.925833, 4.036322, 4.0821]' V
      R0_mat=|
      | [0.011867, 0.008993, 0.007674, 0.006911, 0.006648, 0.006648, 0.006528, 0.006157, 0.005996, 0.0073;
      |  0.0109, 0.006456, 0.005381, 0.005078, 0.005, 0.005044, 0.005511, 0.006407, 0.006522, 0.005367;
      |  0.0102, 0.007978, 0.006793, 0.0062, 0.006033, 0.005441, 0.0051, 0.005707, 0.005037, 0.005067;
      |  0.0101, 0.007759, 0.006637, 0.006022, 0.005741, 0.005667, 0.005311, 0.004911, 0.005859, 0.004733]' Ohm
      R1_mat=|
      | [0.007451, 0.008294, 0.007745, 0.007391;
      |  0.003783, 0.00363, 0.004415, 0.004051;
      |  0.002841, 0.00298, 0.003698, 0.003391;
      |  0.003185, 0.002661, 0.003493, 0.00379;
      |  0.00379, 0.003147, 0.004204, 0.004229;
      |  0.004015, 0.003677, 0.004233, 0.004481;
      |  0.003791, 0.004051, 0.003886, 0.004189;
      |  0.003416, 0.004883, 0.004387, 0.003743;
      |  0.00328, 0.005238, 0.003472, 0.004883;
      |  0.004816, 0.004218, 0.003847, 0.003891] Ohm
      tau1_mat=|
      | [8.156247, 6.866126, 6.747335, 6.573366;
      |  6.436096, 6.88158, 6.206576, 5.30011;
      |  7.074429, 7.267109, 6.564215, 5.759928;
      |  8.61232, 7.062398, 6.553799, 7.485573;
      |  10.88135, 8.569373, 8.681328, 8.99043;
      |  11.88702, 10.35435, 10.74073, 9.985533;
      |  11.15433, 10.61987, 10.52072, 10.95124;
      |  10.33388, 9.573709, 9.987626, 10.94588;
      |  9.883806, 9.219359, 8.513241, 9.109378;
      |  11.2706, 10.03414, 9.643065, 10.06297] s
      R2_mat=|
      | [0.040653, 0.04799, 0.046915, 0.044404;
      |  0.026828, 0.033189, 0.032279, 0.030363;
      |  0.019744, 0.025225, 0.021211, 0.019613;
      |  0.012414, 0.014827, 0.017004, 0.016763;
      |  0.007363, 0.008356, 0.01135, 0.010173;
      |  0.005882, 0.007703, 0.006532, 0.005526;
      |  0.006739, 0.007058, 0.006772, 0.005603;
      |  0.008222, 0.004287, 0.009601, 0.005034;
      |  0.008985, 0.007821, 0.008932, 0.006662;
      |  0.004704, 0.003171, 0.002422, 0.004036] Ohm
      tau2_mat=|
      | [131.6948, 137.0217, 141.2851, 129.3807;
      |  146.2759, 158.6208, 157.255, 143.944;
      |  158.5443, 177.3225, 156.7434, 144.0735;
      |  144.8009, 123.279, 145.0945, 176.1753;
      |  158.7596, 137.3241, 203.2495, 189.2199;
      |  149.8847, 154.5014, 161.1061, 146.3519;
      |  135.3572, 173.7062, 166.0613, 159.34;
      |  123.823, 144.5727, 209.652, 117.4544;
      |  111.7616, 98.04929, 114.3433, 98.05822;
      |  125.3862, 75.97092, 110.7081, 120.3015] s
      settings: InternalSimscapePortConfiguration="{\"Bottom\":[],\"Left\":[{\"id\":\"p\",\"label\":\"+\",\"type\":\"foundation.electrical.electrical\"}],\"Right\":[{\"id\":\"n\",\"label\":\"-\",\"type\":\"foundation.electrical.electrical\"}],\"Top\":[]}"
      settings: LibrarySourceBlock=|
      | batt_lib/Cells/Battery
      | (Table-Based)
